simulink model "model"  (R2014a)
(part 1 of 4)
settings: Solver=VariableStepAuto  StartTime=0.0  StopTime=10.0  RelTol=1e-3
libraries: powerlib x952
settings Model: Creator=lej  LastModifiedBy=leimhofe
settings DataIOCC: SaveFormat=Dataset
settings OptimizationCC: SimCompilerOptimization=off
settings DebuggingCC: MergeDetectMultiDrivingBlocksExec=error  SolverPrmCheckMsg=none  FrameProcessingCompatibilityMsg=error  AllowSymbolicDim=off
settings HardwareCC: ProdBitPerPointer=64  ProdLargestAtomicFloat=Float  ProdIntDivRoundTo=Zero  ProdEndianess=LittleEndian  ProdWordSize=64  ProdHWDeviceType=Intel->x86-64 (Windows64)
settings RTWCC: RTWCompilerOptimization=off
settings GRTTargetCC: GeneratePreprocessorConditionals=Use local settings
settings ConfigComp: CovMetricSettings=dw  CovHtmlReporting=on  CovSaveCumulativeToWorkspaceVar=on  CovSaveSingleToWorkspaceVar=on  CovExternalEMLEnable=off

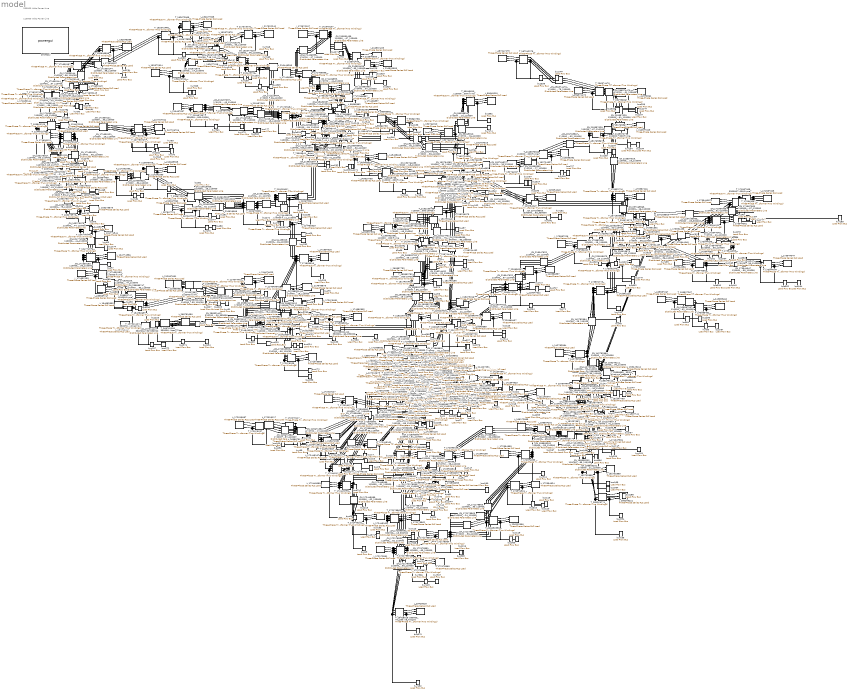
== system model ==
  note: 110000 Volts Power Line
  note: 330000 Volts Power Line
  G_166814917_Kauno_Algirdo_Brazausko_HE : powerlib/Electrical Sources/Three-Phase Source  Voltage=110000  PhaseAngle=0  Frequency=60  InternalConnection=Yg  SpecifyImpedance=on  Resistance=0.8929  Inductance=16.58e-3  ShortCircuitLevel=100e6  BaseVoltage=110000  XRratio=7  BusType=swing  Pref=0  Qref=0  Qmin=-inf  Qmax=inf
  G_172589995_ : powerlib/Electrical Sources/Three-Phase Source  Voltage=330000  PhaseAngle=0  Frequency=60  InternalConnection=Yg  SpecifyImpedance=on  Resistance=0.8929  Inductance=16.58e-3  ShortCircuitLevel=100e6  BaseVoltage=330000  XRratio=7  BusType=swing  Pref=0  Qref=0  Qmin=-inf  Qmax=inf
  L_{25698690,75909941,88726161,95066966,95066982,95866738,99049777,99049787,99049810,103275527,103275551,103275559,103275575,103554499,103560163,104774536,104774544,105587267,106172865,124462106,127212679,130577811..130577812,134987741,135644003,135895688,142782984,149408618,149815795,150992936,151097769,151237667,151783148,151783156,153249112,158244489,158505202,171229484,171406897,171406899,171630121,171630143..171630144,171630149,171630153,171630156..171630157,171809316,171868832,171987005,172018985,172019051,172019085,172019087,172019090,172019115,172019117,172019127,172178550..172178551,172178556,172178560,172178562..172178563,172394893,172394923..172394924,172394941,172407405,172445089,172445101..172445103,172445107,172590051,172590075..172590076,172590080..172590081,172590088,172590095..172590098,172590100..172590101,172590105,172590108,172590115..172590116,172978107,173582215..173582216,173582225..173582226,173591498,173591500,173591502,173593029,173612890,173765447,173944045,173944047,173944055..173944057,173944061,174045384,174586802,175315244,176323123,181769867,187242275,192646598,192672875,192672898,192672903,192672905,192672914,192677018,192702885,192764283,192764310,192764316,192764327,192764330..192764331,192764337,192764347,194082693,207755729..207755730,209204254,210449206,210457037,210457043,210550993,210551439,210555392,210557029,210609525,210612962,210619008,210619011,210995832,212007661,214227031,214455329,214649879,214649882,214674623,215632387,215671382,217323242,217391080,218047622,218214432,218216075,218223015..218223016,219077432,219084048,220065702,220915873,220986987,220989437,221105370,226292390,231990061,239589747,243085462,257169562..257169563,257507721,257684864..257684865,258321412,260552752,265807988,280078882,280269221,296374470} (182 alike) : powerlib/Elements/Three-Phase Series RLC Load  LConnTagsString=A|B|C  Configuration=Y (grounded)  NominalVoltage=110000  NominalFrequency=60  ActivePower=100000  InductivePower=100  CapacitivePower=100  Measurements=None  LoadType=constant Z
  L_{29428018,172590050,197911127,220065689,268781050} (5 alike) : powerlib/Elements/Three-Phase Series RLC Load  LConnTagsString=A|B|C  Configuration=Y (grounded)  NominalVoltage=330000  NominalFrequency=60  ActivePower=100000  InductivePower=100  CapacitivePower=100  Measurements=None  LoadType=constant Z
  T_103275527__ : powerlib/Elements/Three-Phase Transformer (Two Windings)  Winding1Connection=Yg  UNITS=pu  NominalPower=[ 250e6 , 60 ]  Winding1=[110000,0.002,0.08]  Winding2Connection=Yg  Winding2=[110000,0.002,0.08]  SetSaturation=off  Rm=500  Lm=500  Saturation=[ 0,0 ; 0.0024,1.2 ; 1.0,1.52 ]  Hysteresis=off  DataFile='hysteresis'  SetInitialFlux=off  InitialFluxes=[ 0.8 , -0.8 , 0.7 ]  Measurements=None  MoreParameters=off  BreakLoop=off  DataType=off  TransfoNumber=1
  T_103275551__ : powerlib/Elements/Three-Phase Transformer (Two Windings)  Winding1Connection=Yg  UNITS=pu  NominalPower=[ 250e6 , 60 ]  Winding1=[110000,0.002,0.08]  Winding2Connection=Yg  Winding2=[110000,0.002,0.08]  SetSaturation=off  Rm=500  Lm=500  Saturation=[ 0,0 ; 0.0024,1.2 ; 1.0,1.52 ]  Hysteresis=off  DataFile='hysteresis'  SetInitialFlux=off  InitialFluxes=[ 0.8 , -0.8 , 0.7 ]  Measurements=None  MoreParameters=off  BreakLoop=off  DataType=off  TransfoNumber=1
  T_103275559__ : powerlib/Elements/Three-Phase Transformer (Two Windings)  Winding1Connection=Yg  UNITS=pu  NominalPower=[ 250e6 , 60 ]  Winding1=[110000,0.002,0.08]  Winding2Connection=Yg  Winding2=[110000,0.002,0.08]  SetSaturation=off  Rm=500  Lm=500  Saturation=[ 0,0 ; 0.0024,1.2 ; 1.0,1.52 ]  Hysteresis=off  DataFile='hysteresis'  SetInitialFlux=off  InitialFluxes=[ 0.8 , -0.8 , 0.7 ]  Measurements=None  MoreParameters=off  BreakLoop=off  DataType=off  TransfoNumber=1
  T_103275575__ : powerlib/Elements/Three-Phase Transformer (Two Windings)  Winding1Connection=Yg  UNITS=pu  NominalPower=[ 250e6 , 60 ]  Winding1=[110000,0.002,0.08]  Winding2Connection=Yg  Winding2=[110000,0.002,0.08]  SetSaturation=off  Rm=500  Lm=500  Saturation=[ 0,0 ; 0.0024,1.2 ; 1.0,1.52 ]  Hysteresis=off  DataFile='hysteresis'  SetInitialFlux=off  InitialFluxes=[ 0.8 , -0.8 , 0.7 ]  Measurements=None  MoreParameters=off  BreakLoop=off  DataType=off  TransfoNumber=1
  T_103554499__ : powerlib/Elements/Three-Phase Transformer (Two Windings)  Winding1Connection=Yg  UNITS=pu  NominalPower=[ 250e6 , 60 ]  Winding1=[110000,0.002,0.08]  Winding2Connection=Yg  Winding2=[110000,0.002,0.08]  SetSaturation=off  Rm=500  Lm=500  Saturation=[ 0,0 ; 0.0024,1.2 ; 1.0,1.52 ]  Hysteresis=off  DataFile='hysteresis'  SetInitialFlux=off  InitialFluxes=[ 0.8 , -0.8 , 0.7 ]  Measurements=None  MoreParameters=off  BreakLoop=off  DataType=off  TransfoNumber=1
  T_103560163__ : powerlib/Elements/Three-Phase Transformer (Two Windings)  Winding1Connection=Yg  UNITS=pu  NominalPower=[ 250e6 , 60 ]  Winding1=[110000,0.002,0.08]  Winding2Connection=Yg  Winding2=[110000,0.002,0.08]  SetSaturation=off  Rm=500  Lm=500  Saturation=[ 0,0 ; 0.0024,1.2 ; 1.0,1.52 ]  Hysteresis=off  DataFile='hysteresis'  SetInitialFlux=off  InitialFluxes=[ 0.8 , -0.8 , 0.7 ]  Measurements=None  MoreParameters=off  BreakLoop=off  DataType=off  TransfoNumber=1
  T_104774536__ : powerlib/Elements/Three-Phase Transformer (Two Windings)  Winding1Connection=Yg  UNITS=pu  NominalPower=[ 250e6 , 60 ]  Winding1=[110000,0.002,0.08]  Winding2Connection=Yg  Winding2=[110000,0.002,0.08]  SetSaturation=off  Rm=500  Lm=500  Saturation=[ 0,0 ; 0.0024,1.2 ; 1.0,1.52 ]  Hysteresis=off  DataFile='hysteresis'  SetInitialFlux=off  InitialFluxes=[ 0.8 , -0.8 , 0.7 ]  Measurements=None  MoreParameters=off  BreakLoop=off  DataType=off  TransfoNumber=1
  T_104774544__ : powerlib/Elements/Three-Phase Transformer (Two Windings)  Winding1Connection=Yg  UNITS=pu  NominalPower=[ 250e6 , 60 ]  Winding1=[110000,0.002,0.08]  Winding2Connection=Yg  Winding2=[110000,0.002,0.08]  SetSaturation=off  Rm=500  Lm=500  Saturation=[ 0,0 ; 0.0024,1.2 ; 1.0,1.52 ]  Hysteresis=off  DataFile='hysteresis'  SetInitialFlux=off  InitialFluxes=[ 0.8 , -0.8 , 0.7 ]  Measurements=None  MoreParameters=off  BreakLoop=off  DataType=off  TransfoNumber=1
  T_105587267__ : powerlib/Elements/Three-Phase Transformer (Two Windings)  Winding1Connection=Yg  UNITS=pu  NominalPower=[ 250e6 , 60 ]  Winding1=[110000,0.002,0.08]  Winding2Connection=Yg  Winding2=[110000,0.002,0.08]  SetSaturation=off  Rm=500  Lm=500  Saturation=[ 0,0 ; 0.0024,1.2 ; 1.0,1.52 ]  Hysteresis=off  DataFile='hysteresis'  SetInitialFlux=off  InitialFluxes=[ 0.8 , -0.8 , 0.7 ]  Measurements=None  MoreParameters=off  BreakLoop=off  DataType=off  TransfoNumber=1
  T_106172865__ : powerlib/Elements/Three-Phase Transformer (Two Windings)  Winding1Connection=Yg  UNITS=pu  NominalPower=[ 250e6 , 60 ]  Winding1=[110000,0.002,0.08]  Winding2Connection=Yg  Winding2=[110000,0.002,0.08]  SetSaturation=off  Rm=500  Lm=500  Saturation=[ 0,0 ; 0.0024,1.2 ; 1.0,1.52 ]  Hysteresis=off  DataFile='hysteresis'  SetInitialFlux=off  InitialFluxes=[ 0.8 , -0.8 , 0.7 ]  Measurements=None  MoreParameters=off  BreakLoop=off  DataType=off  TransfoNumber=1
  T_124462106__ : powerlib/Elements/Three-Phase Transformer (Two Windings)  Winding1Connection=Yg  UNITS=pu  NominalPower=[ 250e6 , 60 ]  Winding1=[110000,0.002,0.08]  Winding2Connection=Yg  Winding2=[110000,0.002,0.08]  SetSaturation=off  Rm=500  Lm=500  Saturation=[ 0,0 ; 0.0024,1.2 ; 1.0,1.52 ]  Hysteresis=off  DataFile='hysteresis'  SetInitialFlux=off  InitialFluxes=[ 0.8 , -0.8 , 0.7 ]  Measurements=None  MoreParameters=off  BreakLoop=off  DataType=off  TransfoNumber=1
  T_127212679__Noreikiškių_TP : powerlib/Elements/Three-Phase Transformer (Two Windings)  Winding1Connection=Yg  UNITS=pu  NominalPower=[ 250e6 , 60 ]  Winding1=[110000,0.002,0.08]  Winding2Connection=Yg  Winding2=[110000,0.002,0.08]  SetSaturation=off  Rm=500  Lm=500  Saturation=[ 0,0 ; 0.0024,1.2 ; 1.0,1.52 ]  Hysteresis=off  DataFile='hysteresis'  SetInitialFlux=off  InitialFluxes=[ 0.8 , -0.8 , 0.7 ]  Measurements=None  MoreParameters=off  BreakLoop=off  DataType=off  TransfoNumber=1
  T_130577811__Vilijampolės_TP : powerlib/Elements/Three-Phase Transformer (Two Windings)  Winding1Connection=Yg  UNITS=pu  NominalPower=[ 250e6 , 60 ]  Winding1=[110000,0.002,0.08]  Winding2Connection=Yg  Winding2=[110000,0.002,0.08]  SetSaturation=off  Rm=500  Lm=500  Saturation=[ 0,0 ; 0.0024,1.2 ; 1.0,1.52 ]  Hysteresis=off  DataFile='hysteresis'  SetInitialFlux=off  InitialFluxes=[ 0.8 , -0.8 , 0.7 ]  Measurements=None  MoreParameters=off  BreakLoop=off  DataType=off  TransfoNumber=1
  T_130577812__Šilainių_TP : powerlib/Elements/Three-Phase Transformer (Two Windings)  Winding1Connection=Yg  UNITS=pu  NominalPower=[ 250e6 , 60 ]  Winding1=[110000,0.002,0.08]  Winding2Connection=Yg  Winding2=[110000,0.002,0.08]  SetSaturation=off  Rm=500  Lm=500  Saturation=[ 0,0 ; 0.0024,1.2 ; 1.0,1.52 ]  Hysteresis=off  DataFile='hysteresis'  SetInitialFlux=off  InitialFluxes=[ 0.8 , -0.8 , 0.7 ]  Measurements=None  MoreParameters=off  BreakLoop=off  DataType=off  TransfoNumber=1
  T_134987741__ : powerlib/Elements/Three-Phase Transformer (Two Windings)  Winding1Connection=Yg  UNITS=pu  NominalPower=[ 250e6 , 60 ]  Winding1=[110000,0.002,0.08]  Winding2Connection=Yg  Winding2=[110000,0.002,0.08]  SetSaturation=off  Rm=500  Lm=500  Saturation=[ 0,0 ; 0.0024,1.2 ; 1.0,1.52 ]  Hysteresis=off  DataFile='hysteresis'  SetInitialFlux=off  InitialFluxes=[ 0.8 , -0.8 , 0.7 ]  Measurements=None  MoreParameters=off  BreakLoop=off  DataType=off  TransfoNumber=1
  T_135644003__ : powerlib/Elements/Three-Phase Transformer (Two Windings)  Winding1Connection=Yg  UNITS=pu  NominalPower=[ 250e6 , 60 ]  Winding1=[110000,0.002,0.08]  Winding2Connection=Yg  Winding2=[110000,0.002,0.08]  SetSaturation=off  Rm=500  Lm=500  Saturation=[ 0,0 ; 0.0024,1.2 ; 1.0,1.52 ]  Hysteresis=off  DataFile='hysteresis'  SetInitialFlux=off  InitialFluxes=[ 0.8 , -0.8 , 0.7 ]  Measurements=None  MoreParameters=off  BreakLoop=off  DataType=off  TransfoNumber=1
  T_135895688__Palemono_Traukos_TP : powerlib/Elements/Three-Phase Transformer (Two Windings)  Winding1Connection=Yg  UNITS=pu  NominalPower=[ 250e6 , 60 ]  Winding1=[110000,0.002,0.08]  Winding2Connection=Yg  Winding2=[110000,0.002,0.08]  SetSaturation=off  Rm=500  Lm=500  Saturation=[ 0,0 ; 0.0024,1.2 ; 1.0,1.52 ]  Hysteresis=off  DataFile='hysteresis'  SetInitialFlux=off  InitialFluxes=[ 0.8 , -0.8 , 0.7 ]  Measurements=None  MoreParameters=off  BreakLoop=off  DataType=off  TransfoNumber=1
  T_142782984__ : powerlib/Elements/Three-Phase Transformer (Two Windings)  Winding1Connection=Yg  UNITS=pu  NominalPower=[ 250e6 , 60 ]  Winding1=[110000,0.002,0.08]  Winding2Connection=Yg  Winding2=[110000,0.002,0.08]  SetSaturation=off  Rm=500  Lm=500  Saturation=[ 0,0 ; 0.0024,1.2 ; 1.0,1.52 ]  Hysteresis=off  DataFile='hysteresis'  SetInitialFlux=off  InitialFluxes=[ 0.8 , -0.8 , 0.7 ]  Measurements=None  MoreParameters=off  BreakLoop=off  DataType=off  TransfoNumber=1
  T_149408618__ : powerlib/Elements/Three-Phase Transformer (Two Windings)  Winding1Connection=Yg  UNITS=pu  NominalPower=[ 250e6 , 60 ]  Winding1=[110000,0.002,0.08]  Winding2Connection=Yg  Winding2=[110000,0.002,0.08]  SetSaturation=off  Rm=500  Lm=500  Saturation=[ 0,0 ; 0.0024,1.2 ; 1.0,1.52 ]  Hysteresis=off  DataFile='hysteresis'  SetInitialFlux=off  InitialFluxes=[ 0.8 , -0.8 , 0.7 ]  Measurements=None  MoreParameters=off  BreakLoop=off  DataType=off  TransfoNumber=1
  T_149815795_110000;35000;fixme_ : powerlib/Elements/Three-Phase Transformer (Two Windings)  Winding1Connection=Yg  UNITS=pu  NominalPower=[ 250e6 , 60 ]  Winding1=[110000,0.002,0.08]  Winding2Connection=Yg  Winding2=[110000,0.002,0.08]  SetSaturation=off  Rm=500  Lm=500  Saturation=[ 0,0 ; 0.0024,1.2 ; 1.0,1.52 ]  Hysteresis=off  DataFile='hysteresis'  SetInitialFlux=off  InitialFluxes=[ 0.8 , -0.8 , 0.7 ]  Measurements=None  MoreParameters=off  BreakLoop=off  DataType=off  TransfoNumber=1
  T_150992936_110000;35000;fixme_ : powerlib/Elements/Three-Phase Transformer (Two Windings)  Winding1Connection=Yg  UNITS=pu  NominalPower=[ 250e6 , 60 ]  Winding1=[110000,0.002,0.08]  Winding2Connection=Yg  Winding2=[110000,0.002,0.08]  SetSaturation=off  Rm=500  Lm=500  Saturation=[ 0,0 ; 0.0024,1.2 ; 1.0,1.52 ]  Hysteresis=off  DataFile='hysteresis'  SetInitialFlux=off  InitialFluxes=[ 0.8 , -0.8 , 0.7 ]  Measurements=None  MoreParameters=off  BreakLoop=off  DataType=off  TransfoNumber=1
  T_151097769__ : powerlib/Elements/Three-Phase Transformer (Two Windings)  Winding1Connection=Yg  UNITS=pu  NominalPower=[ 250e6 , 60 ]  Winding1=[110000,0.002,0.08]  Winding2Connection=Yg  Winding2=[110000,0.002,0.08]  SetSaturation=off  Rm=500  Lm=500  Saturation=[ 0,0 ; 0.0024,1.2 ; 1.0,1.52 ]  Hysteresis=off  DataFile='hysteresis'  SetInitialFlux=off  InitialFluxes=[ 0.8 , -0.8 , 0.7 ]  Measurements=None  MoreParameters=off  BreakLoop=off  DataType=off  TransfoNumber=1
  T_151237667__ : powerlib/Elements/Three-Phase Transformer (Two Windings)  Winding1Connection=Yg  UNITS=pu  NominalPower=[ 250e6 , 60 ]  Winding1=[110000,0.002,0.08]  Winding2Connection=Yg  Winding2=[110000,0.002,0.08]  SetSaturation=off  Rm=500  Lm=500  Saturation=[ 0,0 ; 0.0024,1.2 ; 1.0,1.52 ]  Hysteresis=off  DataFile='hysteresis'  SetInitialFlux=off  InitialFluxes=[ 0.8 , -0.8 , 0.7 ]  Measurements=None  MoreParameters=off  BreakLoop=off  DataType=off  TransfoNumber=1
  T_151783148_110000;fixme_ : powerlib/Elements/Three-Phase Transformer (Two Windings)  Winding1Connection=Yg  UNITS=pu  NominalPower=[ 250e6 , 60 ]  Winding1=[110000,0.002,0.08]  Winding2Connection=Yg  Winding2=[110000,0.002,0.08]  SetSaturation=off  Rm=500  Lm=500  Saturation=[ 0,0 ; 0.0024,1.2 ; 1.0,1.52 ]  Hysteresis=off  DataFile='hysteresis'  SetInitialFlux=off  InitialFluxes=[ 0.8 , -0.8 , 0.7 ]  Measurements=None  MoreParameters=off  BreakLoop=off  DataType=off  TransfoNumber=1
  T_151783156__ : powerlib/Elements/Three-Phase Transformer (Two Windings)  Winding1Connection=Yg  UNITS=pu  NominalPower=[ 250e6 , 60 ]  Winding1=[110000,0.002,0.08]  Winding2Connection=Yg  Winding2=[110000,0.002,0.08]  SetSaturation=off  Rm=500  Lm=500  Saturation=[ 0,0 ; 0.0024,1.2 ; 1.0,1.52 ]  Hysteresis=off  DataFile='hysteresis'  SetInitialFlux=off  InitialFluxes=[ 0.8 , -0.8 , 0.7 ]  Measurements=None  MoreParameters=off  BreakLoop=off  DataType=off  TransfoNumber=1
  T_153249112__ : powerlib/Elements/Three-Phase Transformer (Two Windings)  Winding1Connection=Yg  UNITS=pu  NominalPower=[ 250e6 , 60 ]  Winding1=[110000,0.002,0.08]  Winding2Connection=Yg  Winding2=[110000,0.002,0.08]  SetSaturation=off  Rm=500  Lm=500  Saturation=[ 0,0 ; 0.0024,1.2 ; 1.0,1.52 ]  Hysteresis=off  DataFile='hysteresis'  SetInitialFlux=off  InitialFluxes=[ 0.8 , -0.8 , 0.7 ]  Measurements=None  MoreParameters=off  BreakLoop=off  DataType=off  TransfoNumber=1
  T_158244489__Palemono_TP : powerlib/Elements/Three-Phase Transformer (Two Windings)  Winding1Connection=Yg  UNITS=pu  NominalPower=[ 250e6 , 60 ]  Winding1=[110000,0.002,0.08]  Winding2Connection=Yg  Winding2=[110000,0.002,0.08]  SetSaturation=off  Rm=500  Lm=500  Saturation=[ 0,0 ; 0.0024,1.2 ; 1.0,1.52 ]  Hysteresis=off  DataFile='hysteresis'  SetInitialFlux=off  InitialFluxes=[ 0.8 , -0.8 , 0.7 ]  Measurements=None  MoreParameters=off  BreakLoop=off  DataType=off  TransfoNumber=1
  T_158505202__ : powerlib/Elements/Three-Phase Transformer (Two Windings)  Winding1Connection=Yg  UNITS=pu  NominalPower=[ 250e6 , 60 ]  Winding1=[330000,0.002,0.08]  Winding2Connection=Yg  Winding2=[110000,0.002,0.08]  SetSaturation=off  Rm=500  Lm=500  Saturation=[ 0,0 ; 0.0024,1.2 ; 1.0,1.52 ]  Hysteresis=off  DataFile='hysteresis'  SetInitialFlux=off  InitialFluxes=[ 0.8 , -0.8 , 0.7 ]  Measurements=None  MoreParameters=off  BreakLoop=off  DataType=off  TransfoNumber=1
  T_171229484__ : powerlib/Elements/Three-Phase Transformer (Two Windings)  Winding1Connection=Yg  UNITS=pu  NominalPower=[ 250e6 , 60 ]  Winding1=[110000,0.002,0.08]  Winding2Connection=Yg  Winding2=[110000,0.002,0.08]  SetSaturation=off  Rm=500  Lm=500  Saturation=[ 0,0 ; 0.0024,1.2 ; 1.0,1.52 ]  Hysteresis=off  DataFile='hysteresis'  SetInitialFlux=off  InitialFluxes=[ 0.8 , -0.8 , 0.7 ]  Measurements=None  MoreParameters=off  BreakLoop=off  DataType=off  TransfoNumber=1
  T_171406897__ : powerlib/Elements/Three-Phase Transformer (Two Windings)  Winding1Connection=Yg  UNITS=pu  NominalPower=[ 250e6 , 60 ]  Winding1=[110000,0.002,0.08]  Winding2Connection=Yg  Winding2=[110000,0.002,0.08]  SetSaturation=off  Rm=500  Lm=500  Saturation=[ 0,0 ; 0.0024,1.2 ; 1.0,1.52 ]  Hysteresis=off  DataFile='hysteresis'  SetInitialFlux=off  InitialFluxes=[ 0.8 , -0.8 , 0.7 ]  Measurements=None  MoreParameters=off  BreakLoop=off  DataType=off  TransfoNumber=1
  T_171406899__ : powerlib/Elements/Three-Phase Transformer (Two Windings)  Winding1Connection=Yg  UNITS=pu  NominalPower=[ 250e6 , 60 ]  Winding1=[110000,0.002,0.08]  Winding2Connection=Yg  Winding2=[110000,0.002,0.08]  SetSaturation=off  Rm=500  Lm=500  Saturation=[ 0,0 ; 0.0024,1.2 ; 1.0,1.52 ]  Hysteresis=off  DataFile='hysteresis'  SetInitialFlux=off  InitialFluxes=[ 0.8 , -0.8 , 0.7 ]  Measurements=None  MoreParameters=off  BreakLoop=off  DataType=off  TransfoNumber=1
  T_171630121__ : powerlib/Elements/Three-Phase Transformer (Two Windings)  Winding1Connection=Yg  UNITS=pu  NominalPower=[ 250e6 , 60 ]  Winding1=[110000,0.002,0.08]  Winding2Connection=Yg  Winding2=[110000,0.002,0.08]  SetSaturation=off  Rm=500  Lm=500  Saturation=[ 0,0 ; 0.0024,1.2 ; 1.0,1.52 ]  Hysteresis=off  DataFile='hysteresis'  SetInitialFlux=off  InitialFluxes=[ 0.8 , -0.8 , 0.7 ]  Measurements=None  MoreParameters=off  BreakLoop=off  DataType=off  TransfoNumber=1
  T_171630143__ : powerlib/Elements/Three-Phase Transformer (Two Windings)  Winding1Connection=Yg  UNITS=pu  NominalPower=[ 250e6 , 60 ]  Winding1=[110000,0.002,0.08]  Winding2Connection=Yg  Winding2=[110000,0.002,0.08]  SetSaturation=off  Rm=500  Lm=500  Saturation=[ 0,0 ; 0.0024,1.2 ; 1.0,1.52 ]  Hysteresis=off  DataFile='hysteresis'  SetInitialFlux=off  InitialFluxes=[ 0.8 , -0.8 , 0.7 ]  Measurements=None  MoreParameters=off  BreakLoop=off  DataType=off  TransfoNumber=1
  T_171630144__ : powerlib/Elements/Three-Phase Transformer (Two Windings)  Winding1Connection=Yg  UNITS=pu  NominalPower=[ 250e6 , 60 ]  Winding1=[110000,0.002,0.08]  Winding2Connection=Yg  Winding2=[110000,0.002,0.08]  SetSaturation=off  Rm=500  Lm=500  Saturation=[ 0,0 ; 0.0024,1.2 ; 1.0,1.52 ]  Hysteresis=off  DataFile='hysteresis'  SetInitialFlux=off  InitialFluxes=[ 0.8 , -0.8 , 0.7 ]  Measurements=None  MoreParameters=off  BreakLoop=off  DataType=off  TransfoNumber=1
  T_171630149__ : powerlib/Elements/Three-Phase Transformer (Two Windings)  Winding1Connection=Yg  UNITS=pu  NominalPower=[ 250e6 , 60 ]  Winding1=[110000,0.002,0.08]  Winding2Connection=Yg  Winding2=[110000,0.002,0.08]  SetSaturation=off  Rm=500  Lm=500  Saturation=[ 0,0 ; 0.0024,1.2 ; 1.0,1.52 ]  Hysteresis=off  DataFile='hysteresis'  SetInitialFlux=off  InitialFluxes=[ 0.8 , -0.8 , 0.7 ]  Measurements=None  MoreParameters=off  BreakLoop=off  DataType=off  TransfoNumber=1
  T_171630153_110000;fixme_ : powerlib/Elements/Three-Phase Transformer (Two Windings)  Winding1Connection=Yg  UNITS=pu  NominalPower=[ 250e6 , 60 ]  Winding1=[110000,0.002,0.08]  Winding2Connection=Yg  Winding2=[110000,0.002,0.08]  SetSaturation=off  Rm=500  Lm=500  Saturation=[ 0,0 ; 0.0024,1.2 ; 1.0,1.52 ]  Hysteresis=off  DataFile='hysteresis'  SetInitialFlux=off  InitialFluxes=[ 0.8 , -0.8 , 0.7 ]  Measurements=None  MoreParameters=off  BreakLoop=off  DataType=off  TransfoNumber=1
  T_171630156__ : powerlib/Elements/Three-Phase Transformer (Two Windings)  Winding1Connection=Yg  UNITS=pu  NominalPower=[ 250e6 , 60 ]  Winding1=[110000,0.002,0.08]  Winding2Connection=Yg  Winding2=[110000,0.002,0.08]  SetSaturation=off  Rm=500  Lm=500  Saturation=[ 0,0 ; 0.0024,1.2 ; 1.0,1.52 ]  Hysteresis=off  DataFile='hysteresis'  SetInitialFlux=off  InitialFluxes=[ 0.8 , -0.8 , 0.7 ]  Measurements=None  MoreParameters=off  BreakLoop=off  DataType=off  TransfoNumber=1
  T_171630157__ : powerlib/Elements/Three-Phase Transformer (Two Windings)  Winding1Connection=Yg  UNITS=pu  NominalPower=[ 250e6 , 60 ]  Winding1=[110000,0.002,0.08]  Winding2Connection=Yg  Winding2=[110000,0.002,0.08]  SetSaturation=off  Rm=500  Lm=500  Saturation=[ 0,0 ; 0.0024,1.2 ; 1.0,1.52 ]  Hysteresis=off  DataFile='hysteresis'  SetInitialFlux=off  InitialFluxes=[ 0.8 , -0.8 , 0.7 ]  Measurements=None  MoreParameters=off  BreakLoop=off  DataType=off  TransfoNumber=1
  T_171809316__ : powerlib/Elements/Three-Phase Transformer (Two Windings)  Winding1Connection=Yg  UNITS=pu  NominalPower=[ 250e6 , 60 ]  Winding1=[110000,0.002,0.08]  Winding2Connection=Yg  Winding2=[110000,0.002,0.08]  SetSaturation=off  Rm=500  Lm=500  Saturation=[ 0,0 ; 0.0024,1.2 ; 1.0,1.52 ]  Hysteresis=off  DataFile='hysteresis'  SetInitialFlux=off  InitialFluxes=[ 0.8 , -0.8 , 0.7 ]  Measurements=None  MoreParameters=off  BreakLoop=off  DataType=off  TransfoNumber=1
  T_171868832__ : powerlib/Elements/Three-Phase Transformer (Two Windings)  Winding1Connection=Yg  UNITS=pu  NominalPower=[ 250e6 , 60 ]  Winding1=[110000,0.002,0.08]  Winding2Connection=Yg  Winding2=[110000,0.002,0.08]  SetSaturation=off  Rm=500  Lm=500  Saturation=[ 0,0 ; 0.0024,1.2 ; 1.0,1.52 ]  Hysteresis=off  DataFile='hysteresis'  SetInitialFlux=off  InitialFluxes=[ 0.8 , -0.8 , 0.7 ]  Measurements=None  MoreParameters=off  BreakLoop=off  DataType=off  TransfoNumber=1
  T_171987005_330000;110000;fixme_ : powerlib/Elements/Three-Phase Transformer (Two Windings)  Winding1Connection=Yg  UNITS=pu  NominalPower=[ 250e6 , 60 ]  Winding1=[330000,0.002,0.08]  Winding2Connection=Yg  Winding2=[110000,0.002,0.08]  SetSaturation=off  Rm=500  Lm=500  Saturation=[ 0,0 ; 0.0024,1.2 ; 1.0,1.52 ]  Hysteresis=off  DataFile='hysteresis'  SetInitialFlux=off  InitialFluxes=[ 0.8 , -0.8 , 0.7 ]  Measurements=None  MoreParameters=off  BreakLoop=off  DataType=off  TransfoNumber=1
  T_172018985__ : powerlib/Elements/Three-Phase Transformer (Two Windings)  Winding1Connection=Yg  UNITS=pu  NominalPower=[ 250e6 , 60 ]  Winding1=[110000,0.002,0.08]  Winding2Connection=Yg  Winding2=[110000,0.002,0.08]  SetSaturation=off  Rm=500  Lm=500  Saturation=[ 0,0 ; 0.0024,1.2 ; 1.0,1.52 ]  Hysteresis=off  DataFile='hysteresis'  SetInitialFlux=off  InitialFluxes=[ 0.8 , -0.8 , 0.7 ]  Measurements=None  MoreParameters=off  BreakLoop=off  DataType=off  TransfoNumber=1
  T_172019051__ : powerlib/Elements/Three-Phase Transformer (Two Windings)  Winding1Connection=Yg  UNITS=pu  NominalPower=[ 250e6 , 60 ]  Winding1=[110000,0.002,0.08]  Winding2Connection=Yg  Winding2=[110000,0.002,0.08]  SetSaturation=off  Rm=500  Lm=500  Saturation=[ 0,0 ; 0.0024,1.2 ; 1.0,1.52 ]  Hysteresis=off  DataFile='hysteresis'  SetInitialFlux=off  InitialFluxes=[ 0.8 , -0.8 , 0.7 ]  Measurements=None  MoreParameters=off  BreakLoop=off  DataType=off  TransfoNumber=1
  T_172019085__ : powerlib/Elements/Three-Phase Transformer (Two Windings)  Winding1Connection=Yg  UNITS=pu  NominalPower=[ 250e6 , 60 ]  Winding1=[110000,0.002,0.08]  Winding2Connection=Yg  Winding2=[110000,0.002,0.08]  SetSaturation=off  Rm=500  Lm=500  Saturation=[ 0,0 ; 0.0024,1.2 ; 1.0,1.52 ]  Hysteresis=off  DataFile='hysteresis'  SetInitialFlux=off  InitialFluxes=[ 0.8 , -0.8 , 0.7 ]  Measurements=None  MoreParameters=off  BreakLoop=off  DataType=off  TransfoNumber=1
  T_172019087__ : powerlib/Elements/Three-Phase Transformer (Two Windings)  Winding1Connection=Yg  UNITS=pu  NominalPower=[ 250e6 , 60 ]  Winding1=[110000,0.002,0.08]  Winding2Connection=Yg  Winding2=[110000,0.002,0.08]  SetSaturation=off  Rm=500  Lm=500  Saturation=[ 0,0 ; 0.0024,1.2 ; 1.0,1.52 ]  Hysteresis=off  DataFile='hysteresis'  SetInitialFlux=off  InitialFluxes=[ 0.8 , -0.8 , 0.7 ]  Measurements=None  MoreParameters=off  BreakLoop=off  DataType=off  TransfoNumber=1
  T_172019090__ : powerlib/Elements/Three-Phase Transformer (Two Windings)  Winding1Connection=Yg  UNITS=pu  NominalPower=[ 250e6 , 60 ]  Winding1=[110000,0.002,0.08]  Winding2Connection=Yg  Winding2=[110000,0.002,0.08]  SetSaturation=off  Rm=500  Lm=500  Saturation=[ 0,0 ; 0.0024,1.2 ; 1.0,1.52 ]  Hysteresis=off  DataFile='hysteresis'  SetInitialFlux=off  InitialFluxes=[ 0.8 , -0.8 , 0.7 ]  Measurements=None  MoreParameters=off  BreakLoop=off  DataType=off  TransfoNumber=1
  T_172019115__Aleksoto_TP : powerlib/Elements/Three-Phase Transformer (Two Windings)  Winding1Connection=Yg  UNITS=pu  NominalPower=[ 250e6 , 60 ]  Winding1=[110000,0.002,0.08]  Winding2Connection=Yg  Winding2=[110000,0.002,0.08]  SetSaturation=off  Rm=500  Lm=500  Saturation=[ 0,0 ; 0.0024,1.2 ; 1.0,1.52 ]  Hysteresis=off  DataFile='hysteresis'  SetInitialFlux=off  InitialFluxes=[ 0.8 , -0.8 , 0.7 ]  Measurements=None  MoreParameters=off  BreakLoop=off  DataType=off  TransfoNumber=1
  T_172019117__ : powerlib/Elements/Three-Phase Transformer (Two Windings)  Winding1Connection=Yg  UNITS=pu  NominalPower=[ 250e6 , 60 ]  Winding1=[110000,0.002,0.08]  Winding2Connection=Yg  Winding2=[110000,0.002,0.08]  SetSaturation=off  Rm=500  Lm=500  Saturation=[ 0,0 ; 0.0024,1.2 ; 1.0,1.52 ]  Hysteresis=off  DataFile='hysteresis'  SetInitialFlux=off  InitialFluxes=[ 0.8 , -0.8 , 0.7 ]  Measurements=None  MoreParameters=off  BreakLoop=off  DataType=off  TransfoNumber=1
  T_172019127__ : powerlib/Elements/Three-Phase Transformer (Two Windings)  Winding1Connection=Yg  UNITS=pu  NominalPower=[ 250e6 , 60 ]  Winding1=[110000,0.002,0.08]  Winding2Connection=Yg  Winding2=[110000,0.002,0.08]  SetSaturation=off  Rm=500  Lm=500  Saturation=[ 0,0 ; 0.0024,1.2 ; 1.0,1.52 ]  Hysteresis=off  DataFile='hysteresis'  SetInitialFlux=off  InitialFluxes=[ 0.8 , -0.8 , 0.7 ]  Measurements=None  MoreParameters=off  BreakLoop=off  DataType=off  TransfoNumber=1
  T_172178550__ : powerlib/Elements/Three-Phase Transformer (Two Windings)  Winding1Connection=Yg  UNITS=pu  NominalPower=[ 250e6 , 60 ]  Winding1=[110000,0.002,0.08]  Winding2Connection=Yg  Winding2=[110000,0.002,0.08]  SetSaturation=off  Rm=500  Lm=500  Saturation=[ 0,0 ; 0.0024,1.2 ; 1.0,1.52 ]  Hysteresis=off  DataFile='hysteresis'  SetInitialFlux=off  InitialFluxes=[ 0.8 , -0.8 , 0.7 ]  Measurements=None  MoreParameters=off  BreakLoop=off  DataType=off  TransfoNumber=1
  T_172178551__ : powerlib/Elements/Three-Phase Transformer (Two Windings)  Winding1Connection=Yg  UNITS=pu  NominalPower=[ 250e6 , 60 ]  Winding1=[110000,0.002,0.08]  Winding2Connection=Yg  Winding2=[110000,0.002,0.08]  SetSaturation=off  Rm=500  Lm=500  Saturation=[ 0,0 ; 0.0024,1.2 ; 1.0,1.52 ]  Hysteresis=off  DataFile='hysteresis'  SetInitialFlux=off  InitialFluxes=[ 0.8 , -0.8 , 0.7 ]  Measurements=None  MoreParameters=off  BreakLoop=off  DataType=off  TransfoNumber=1
  T_172178556__ : powerlib/Elements/Three-Phase Transformer (Two Windings)  Winding1Connection=Yg  UNITS=pu  NominalPower=[ 250e6 , 60 ]  Winding1=[110000,0.002,0.08]  Winding2Connection=Yg  Winding2=[110000,0.002,0.08]  SetSaturation=off  Rm=500  Lm=500  Saturation=[ 0,0 ; 0.0024,1.2 ; 1.0,1.52 ]  Hysteresis=off  DataFile='hysteresis'  SetInitialFlux=off  InitialFluxes=[ 0.8 , -0.8 , 0.7 ]  Measurements=None  MoreParameters=off  BreakLoop=off  DataType=off  TransfoNumber=1
  T_172178560__ : powerlib/Elements/Three-Phase Transformer (Two Windings)  Winding1Connection=Yg  UNITS=pu  NominalPower=[ 250e6 , 60 ]  Winding1=[110000,0.002,0.08]  Winding2Connection=Yg  Winding2=[110000,0.002,0.08]  SetSaturation=off  Rm=500  Lm=500  Saturation=[ 0,0 ; 0.0024,1.2 ; 1.0,1.52 ]  Hysteresis=off  DataFile='hysteresis'  SetInitialFlux=off  InitialFluxes=[ 0.8 , -0.8 , 0.7 ]  Measurements=None  MoreParameters=off  BreakLoop=off  DataType=off  TransfoNumber=1
  T_172178562__ : powerlib/Elements/Three-Phase Transformer (Two Windings)  Winding1Connection=Yg  UNITS=pu  NominalPower=[ 250e6 , 60 ]  Winding1=[110000,0.002,0.08]  Winding2Connection=Yg  Winding2=[110000,0.002,0.08]  SetSaturation=off  Rm=500  Lm=500  Saturation=[ 0,0 ; 0.0024,1.2 ; 1.0,1.52 ]  Hysteresis=off  DataFile='hysteresis'  SetInitialFlux=off  InitialFluxes=[ 0.8 , -0.8 , 0.7 ]  Measurements=None  MoreParameters=off  BreakLoop=off  DataType=off  TransfoNumber=1
  T_172178563__ : powerlib/Elements/Three-Phase Transformer (Two Windings)  Winding1Connection=Yg  UNITS=pu  NominalPower=[ 250e6 , 60 ]  Winding1=[110000,0.002,0.08]  Winding2Connection=Yg  Winding2=[110000,0.002,0.08]  SetSaturation=off  Rm=500  Lm=500  Saturation=[ 0,0 ; 0.0024,1.2 ; 1.0,1.52 ]  Hysteresis=off  DataFile='hysteresis'  SetInitialFlux=off  InitialFluxes=[ 0.8 , -0.8 , 0.7 ]  Measurements=None  MoreParameters=off  BreakLoop=off  DataType=off  TransfoNumber=1
  T_172394893__ : powerlib/Elements/Three-Phase Transformer (Two Windings)  Winding1Connection=Yg  UNITS=pu  NominalPower=[ 250e6 , 60 ]  Winding1=[110000,0.002,0.08]  Winding2Connection=Yg  Winding2=[110000,0.002,0.08]  SetSaturation=off  Rm=500  Lm=500  Saturation=[ 0,0 ; 0.0024,1.2 ; 1.0,1.52 ]  Hysteresis=off  DataFile='hysteresis'  SetInitialFlux=off  InitialFluxes=[ 0.8 , -0.8 , 0.7 ]  Measurements=None  MoreParameters=off  BreakLoop=off  DataType=off  TransfoNumber=1
  T_172394923__ : powerlib/Elements/Three-Phase Transformer (Two Windings)  Winding1Connection=Yg  UNITS=pu  NominalPower=[ 250e6 , 60 ]  Winding1=[110000,0.002,0.08]  Winding2Connection=Yg  Winding2=[110000,0.002,0.08]  SetSaturation=off  Rm=500  Lm=500  Saturation=[ 0,0 ; 0.0024,1.2 ; 1.0,1.52 ]  Hysteresis=off  DataFile='hysteresis'  SetInitialFlux=off  InitialFluxes=[ 0.8 , -0.8 , 0.7 ]  Measurements=None  MoreParameters=off  BreakLoop=off  DataType=off  TransfoNumber=1
  T_172394924__ : powerlib/Elements/Three-Phase Transformer (Two Windings)  Winding1Connection=Yg  UNITS=pu  NominalPower=[ 250e6 , 60 ]  Winding1=[110000,0.002,0.08]  Winding2Connection=Yg  Winding2=[110000,0.002,0.08]  SetSaturation=off  Rm=500  Lm=500  Saturation=[ 0,0 ; 0.0024,1.2 ; 1.0,1.52 ]  Hysteresis=off  DataFile='hysteresis'  SetInitialFlux=off  InitialFluxes=[ 0.8 , -0.8 , 0.7 ]  Measurements=None  MoreParameters=off  BreakLoop=off  DataType=off  TransfoNumber=1
  T_172394941__ : powerlib/Elements/Three-Phase Transformer (Two Windings)  Winding1Connection=Yg  UNITS=pu  NominalPower=[ 250e6 , 60 ]  Winding1=[110000,0.002,0.08]  Winding2Connection=Yg  Winding2=[110000,0.002,0.08]  SetSaturation=off  Rm=500  Lm=500  Saturation=[ 0,0 ; 0.0024,1.2 ; 1.0,1.52 ]  Hysteresis=off  DataFile='hysteresis'  SetInitialFlux=off  InitialFluxes=[ 0.8 , -0.8 , 0.7 ]  Measurements=None  MoreParameters=off  BreakLoop=off  DataType=off  TransfoNumber=1
  T_172407405__ : powerlib/Elements/Three-Phase Transformer (Two Windings)  Winding1Connection=Yg  UNITS=pu  NominalPower=[ 250e6 , 60 ]  Winding1=[110000,0.002,0.08]  Winding2Connection=Yg  Winding2=[110000,0.002,0.08]  SetSaturation=off  Rm=500  Lm=500  Saturation=[ 0,0 ; 0.0024,1.2 ; 1.0,1.52 ]  Hysteresis=off  DataFile='hysteresis'  SetInitialFlux=off  InitialFluxes=[ 0.8 , -0.8 , 0.7 ]  Measurements=None  MoreParameters=off  BreakLoop=off  DataType=off  TransfoNumber=1
  T_172445089__ : powerlib/Elements/Three-Phase Transformer (Two Windings)  Winding1Connection=Yg  UNITS=pu  NominalPower=[ 250e6 , 60 ]  Winding1=[110000,0.002,0.08]  Winding2Connection=Yg  Winding2=[110000,0.002,0.08]  SetSaturation=off  Rm=500  Lm=500  Saturation=[ 0,0 ; 0.0024,1.2 ; 1.0,1.52 ]  Hysteresis=off  DataFile='hysteresis'  SetInitialFlux=off  InitialFluxes=[ 0.8 , -0.8 , 0.7 ]  Measurements=None  MoreParameters=off  BreakLoop=off  DataType=off  TransfoNumber=1
  T_172445101__ : powerlib/Elements/Three-Phase Transformer (Two Windings)  Winding1Connection=Yg  UNITS=pu  NominalPower=[ 250e6 , 60 ]  Winding1=[110000,0.002,0.08]  Winding2Connection=Yg  Winding2=[110000,0.002,0.08]  SetSaturation=off  Rm=500  Lm=500  Saturation=[ 0,0 ; 0.0024,1.2 ; 1.0,1.52 ]  Hysteresis=off  DataFile='hysteresis'  SetInitialFlux=off  InitialFluxes=[ 0.8 , -0.8 , 0.7 ]  Measurements=None  MoreParameters=off  BreakLoop=off  DataType=off  TransfoNumber=1
  T_172445102__ : powerlib/Elements/Three-Phase Transformer (Two Windings)  Winding1Connection=Yg  UNITS=pu  NominalPower=[ 250e6 , 60 ]  Winding1=[110000,0.002,0.08]  Winding2Connection=Yg  Winding2=[110000,0.002,0.08]  SetSaturation=off  Rm=500  Lm=500  Saturation=[ 0,0 ; 0.0024,1.2 ; 1.0,1.52 ]  Hysteresis=off  DataFile='hysteresis'  SetInitialFlux=off  InitialFluxes=[ 0.8 , -0.8 , 0.7 ]  Measurements=None  MoreParameters=off  BreakLoop=off  DataType=off  TransfoNumber=1
  T_172445103__ : powerlib/Elements/Three-Phase Transformer (Two Windings)  Winding1Connection=Yg  UNITS=pu  NominalPower=[ 250e6 , 60 ]  Winding1=[110000,0.002,0.08]  Winding2Connection=Yg  Winding2=[110000,0.002,0.08]  SetSaturation=off  Rm=500  Lm=500  Saturation=[ 0,0 ; 0.0024,1.2 ; 1.0,1.52 ]  Hysteresis=off  DataFile='hysteresis'  SetInitialFlux=off  InitialFluxes=[ 0.8 , -0.8 , 0.7 ]  Measurements=None  MoreParameters=off  BreakLoop=off  DataType=off  TransfoNumber=1
  T_172445107__ : powerlib/Elements/Three-Phase Transformer (Two Windings)  Winding1Connection=Yg  UNITS=pu  NominalPower=[ 250e6 , 60 ]  Winding1=[110000,0.002,0.08]  Winding2Connection=Yg  Winding2=[110000,0.002,0.08]  SetSaturation=off  Rm=500  Lm=500  Saturation=[ 0,0 ; 0.0024,1.2 ; 1.0,1.52 ]  Hysteresis=off  DataFile='hysteresis'  SetInitialFlux=off  InitialFluxes=[ 0.8 , -0.8 , 0.7 ]  Measurements=None  MoreParameters=off  BreakLoop=off  DataType=off  TransfoNumber=1
  T_172590050_330000_ : powerlib/Elements/Three-Phase Transformer (Two Windings)  Winding1Connection=Yg  UNITS=pu  NominalPower=[ 250e6 , 60 ]  Winding1=[330000,0.002,0.08]  Winding2Connection=Yg  Winding2=[330000,0.002,0.08]  SetSaturation=off  Rm=500  Lm=500  Saturation=[ 0,0 ; 0.0024,1.2 ; 1.0,1.52 ]  Hysteresis=off  DataFile='hysteresis'  SetInitialFlux=off  InitialFluxes=[ 0.8 , -0.8 , 0.7 ]  Measurements=None  MoreParameters=off  BreakLoop=off  DataType=off  TransfoNumber=1
  T_172590051__ : powerlib/Elements/Three-Phase Transformer (Two Windings)  Winding1Connection=Yg  UNITS=pu  NominalPower=[ 250e6 , 60 ]  Winding1=[330000,0.002,0.08]  Winding2Connection=Yg  Winding2=[110000,0.002,0.08]  SetSaturation=off  Rm=500  Lm=500  Saturation=[ 0,0 ; 0.0024,1.2 ; 1.0,1.52 ]  Hysteresis=off  DataFile='hysteresis'  SetInitialFlux=off  InitialFluxes=[ 0.8 , -0.8 , 0.7 ]  Measurements=None  MoreParameters=off  BreakLoop=off  DataType=off  TransfoNumber=1
  T_172590075__Žasmos_TP : powerlib/Elements/Three-Phase Transformer (Two Windings)  Winding1Connection=Yg  UNITS=pu  NominalPower=[ 250e6 , 60 ]  Winding1=[110000,0.002,0.08]  Winding2Connection=Yg  Winding2=[110000,0.002,0.08]  SetSaturation=off  Rm=500  Lm=500  Saturation=[ 0,0 ; 0.0024,1.2 ; 1.0,1.52 ]  Hysteresis=off  DataFile='hysteresis'  SetInitialFlux=off  InitialFluxes=[ 0.8 , -0.8 , 0.7 ]  Measurements=None  MoreParameters=off  BreakLoop=off  DataType=off  TransfoNumber=1
  T_172590076__ : powerlib/Elements/Three-Phase Transformer (Two Windings)  Winding1Connection=Yg  UNITS=pu  NominalPower=[ 250e6 , 60 ]  Winding1=[110000,0.002,0.08]  Winding2Connection=Yg  Winding2=[110000,0.002,0.08]  SetSaturation=off  Rm=500  Lm=500  Saturation=[ 0,0 ; 0.0024,1.2 ; 1.0,1.52 ]  Hysteresis=off  DataFile='hysteresis'  SetInitialFlux=off  InitialFluxes=[ 0.8 , -0.8 , 0.7 ]  Measurements=None  MoreParameters=off  BreakLoop=off  DataType=off  TransfoNumber=1
  T_172590080__ : powerlib/Elements/Three-Phase Transformer (Two Windings)  Winding1Connection=Yg  UNITS=pu  NominalPower=[ 250e6 , 60 ]  Winding1=[110000,0.002,0.08]  Winding2Connection=Yg  Winding2=[110000,0.002,0.08]  SetSaturation=off  Rm=500  Lm=500  Saturation=[ 0,0 ; 0.0024,1.2 ; 1.0,1.52 ]  Hysteresis=off  DataFile='hysteresis'  SetInitialFlux=off  InitialFluxes=[ 0.8 , -0.8 , 0.7 ]  Measurements=None  MoreParameters=off  BreakLoop=off  DataType=off  TransfoNumber=1
  T_172590081__ : powerlib/Elements/Three-Phase Transformer (Two Windings)  Winding1Connection=Yg  UNITS=pu  NominalPower=[ 250e6 , 60 ]  Winding1=[110000,0.002,0.08]  Winding2Connection=Yg  Winding2=[110000,0.002,0.08]  SetSaturation=off  Rm=500  Lm=500  Saturation=[ 0,0 ; 0.0024,1.2 ; 1.0,1.52 ]  Hysteresis=off  DataFile='hysteresis'  SetInitialFlux=off  InitialFluxes=[ 0.8 , -0.8 , 0.7 ]  Measurements=None  MoreParameters=off  BreakLoop=off  DataType=off  TransfoNumber=1
  T_172590088__ : powerlib/Elements/Three-Phase Transformer (Two Windings)  Winding1Connection=Yg  UNITS=pu  NominalPower=[ 250e6 , 60 ]  Winding1=[110000,0.002,0.08]  Winding2Connection=Yg  Winding2=[110000,0.002,0.08]  SetSaturation=off  Rm=500  Lm=500  Saturation=[ 0,0 ; 0.0024,1.2 ; 1.0,1.52 ]  Hysteresis=off  DataFile='hysteresis'  SetInitialFlux=off  InitialFluxes=[ 0.8 , -0.8 , 0.7 ]  Measurements=None  MoreParameters=off  BreakLoop=off  DataType=off  TransfoNumber=1
  T_172590095__ : powerlib/Elements/Three-Phase Transformer (Two Windings)  Winding1Connection=Yg  UNITS=pu  NominalPower=[ 250e6 , 60 ]  Winding1=[110000,0.002,0.08]  Winding2Connection=Yg  Winding2=[110000,0.002,0.08]  SetSaturation=off  Rm=500  Lm=500  Saturation=[ 0,0 ; 0.0024,1.2 ; 1.0,1.52 ]  Hysteresis=off  DataFile='hysteresis'  SetInitialFlux=off  InitialFluxes=[ 0.8 , -0.8 , 0.7 ]  Measurements=None  MoreParameters=off  BreakLoop=off  DataType=off  TransfoNumber=1
  T_172590096__ : powerlib/Elements/Three-Phase Transformer (Two Windings)  Winding1Connection=Yg  UNITS=pu  NominalPower=[ 250e6 , 60 ]  Winding1=[110000,0.002,0.08]  Winding2Connection=Yg  Winding2=[110000,0.002,0.08]  SetSaturation=off  Rm=500  Lm=500  Saturation=[ 0,0 ; 0.0024,1.2 ; 1.0,1.52 ]  Hysteresis=off  DataFile='hysteresis'  SetInitialFlux=off  InitialFluxes=[ 0.8 , -0.8 , 0.7 ]  Measurements=None  MoreParameters=off  BreakLoop=off  DataType=off  TransfoNumber=1
  T_172590097__ : powerlib/Elements/Three-Phase Transformer (Two Windings)  Winding1Connection=Yg  UNITS=pu  NominalPower=[ 250e6 , 60 ]  Winding1=[110000,0.002,0.08]  Winding2Connection=Yg  Winding2=[110000,0.002,0.08]  SetSaturation=off  Rm=500  Lm=500  Saturation=[ 0,0 ; 0.0024,1.2 ; 1.0,1.52 ]  Hysteresis=off  DataFile='hysteresis'  SetInitialFlux=off  InitialFluxes=[ 0.8 , -0.8 , 0.7 ]  Measurements=None  MoreParameters=off  BreakLoop=off  DataType=off  TransfoNumber=1
  T_172590098__Drobės_TP : powerlib/Elements/Three-Phase Transformer (Two Windings)  Winding1Connection=Yg  UNITS=pu  NominalPower=[ 250e6 , 60 ]  Winding1=[110000,0.002,0.08]  Winding2Connection=Yg  Winding2=[110000,0.002,0.08]  SetSaturation=off  Rm=500  Lm=500  Saturation=[ 0,0 ; 0.0024,1.2 ; 1.0,1.52 ]  Hysteresis=off  DataFile='hysteresis'  SetInitialFlux=off  InitialFluxes=[ 0.8 , -0.8 , 0.7 ]  Measurements=None  MoreParameters=off  BreakLoop=off  DataType=off  TransfoNumber=1
  T_172590100__Rokų_TP : powerlib/Elements/Three-Phase Transformer (Two Windings)  Winding1Connection=Yg  UNITS=pu  NominalPower=[ 250e6 , 60 ]  Winding1=[110000,0.002,0.08]  Winding2Connection=Yg  Winding2=[110000,0.002,0.08]  SetSaturation=off  Rm=500  Lm=500  Saturation=[ 0,0 ; 0.0024,1.2 ; 1.0,1.52 ]  Hysteresis=off  DataFile='hysteresis'  SetInitialFlux=off  InitialFluxes=[ 0.8 , -0.8 , 0.7 ]  Measurements=None  MoreParameters=off  BreakLoop=off  DataType=off  TransfoNumber=1
  T_172590101__Petrašiūnų_TP : powerlib/Elements/Three-Phase Transformer (Two Windings)  Winding1Connection=Yg  UNITS=pu  NominalPower=[ 250e6 , 60 ]  Winding1=[110000,0.002,0.08]  Winding2Connection=Yg  Winding2=[110000,0.002,0.08]  SetSaturation=off  Rm=500  Lm=500  Saturation=[ 0,0 ; 0.0024,1.2 ; 1.0,1.52 ]  Hysteresis=off  DataFile='hysteresis'  SetInitialFlux=off  InitialFluxes=[ 0.8 , -0.8 , 0.7 ]  Measurements=None  MoreParameters=off  BreakLoop=off  DataType=off  TransfoNumber=1
  T_172590105__Ketaus_TP : powerlib/Elements/Three-Phase Transformer (Two Windings)  Winding1Connection=Yg  UNITS=pu  NominalPower=[ 250e6 , 60 ]  Winding1=[110000,0.002,0.08]  Winding2Connection=Yg  Winding2=[110000,0.002,0.08]  SetSaturation=off  Rm=500  Lm=500  Saturation=[ 0,0 ; 0.0024,1.2 ; 1.0,1.52 ]  Hysteresis=off  DataFile='hysteresis'  SetInitialFlux=off  InitialFluxes=[ 0.8 , -0.8 , 0.7 ]  Measurements=None  MoreParameters=off  BreakLoop=off  DataType=off  TransfoNumber=1
  T_172590108__ : powerlib/Elements/Three-Phase Transformer (Two Windings)  Winding1Connection=Yg  UNITS=pu  NominalPower=[ 250e6 , 60 ]  Winding1=[110000,0.002,0.08]  Winding2Connection=Yg  Winding2=[110000,0.002,0.08]  SetSaturation=off  Rm=500  Lm=500  Saturation=[ 0,0 ; 0.0024,1.2 ; 1.0,1.52 ]  Hysteresis=off  DataFile='hysteresis'  SetInitialFlux=off  InitialFluxes=[ 0.8 , -0.8 , 0.7 ]  Measurements=None  MoreParameters=off  BreakLoop=off  DataType=off  TransfoNumber=1
  T_172590115_330000;110000;fixme_ : powerlib/Elements/Three-Phase Transformer (Two Windings)  Winding1Connection=Yg  UNITS=pu  NominalPower=[ 250e6 , 60 ]  Winding1=[330000,0.002,0.08]  Winding2Connection=Yg  Winding2=[110000,0.002,0.08]  SetSaturation=off  Rm=500  Lm=500  Saturation=[ 0,0 ; 0.0024,1.2 ; 1.0,1.52 ]  Hysteresis=off  DataFile='hysteresis'  SetInitialFlux=off  InitialFluxes=[ 0.8 , -0.8 , 0.7 ]  Measurements=None  MoreParameters=off  BreakLoop=off  DataType=off  TransfoNumber=1
  T_172590116__ : powerlib/Elements/Three-Phase Transformer (Two Windings)  Winding1Connection=Yg  UNITS=pu  NominalPower=[ 250e6 , 60 ]  Winding1=[110000,0.002,0.08]  Winding2Connection=Yg  Winding2=[110000,0.002,0.08]  SetSaturation=off  Rm=500  Lm=500  Saturation=[ 0,0 ; 0.0024,1.2 ; 1.0,1.52 ]  Hysteresis=off  DataFile='hysteresis'  SetInitialFlux=off  InitialFluxes=[ 0.8 , -0.8 , 0.7 ]  Measurements=None  MoreParameters=off  BreakLoop=off  DataType=off  TransfoNumber=1
  T_172978107__ : powerlib/Elements/Three-Phase Transformer (Two Windings)  Winding1Connection=Yg  UNITS=pu  NominalPower=[ 250e6 , 60 ]  Winding1=[110000,0.002,0.08]  Winding2Connection=Yg  Winding2=[110000,0.002,0.08]  SetSaturation=off  Rm=500  Lm=500  Saturation=[ 0,0 ; 0.0024,1.2 ; 1.0,1.52 ]  Hysteresis=off  DataFile='hysteresis'  SetInitialFlux=off  InitialFluxes=[ 0.8 , -0.8 , 0.7 ]  Measurements=None  MoreParameters=off  BreakLoop=off  DataType=off  TransfoNumber=1
  T_173582215__ : powerlib/Elements/Three-Phase Transformer (Two Windings)  Winding1Connection=Yg  UNITS=pu  NominalPower=[ 250e6 , 60 ]  Winding1=[110000,0.002,0.08]  Winding2Connection=Yg  Winding2=[110000,0.002,0.08]  SetSaturation=off  Rm=500  Lm=500  Saturation=[ 0,0 ; 0.0024,1.2 ; 1.0,1.52 ]  Hysteresis=off  DataFile='hysteresis'  SetInitialFlux=off  InitialFluxes=[ 0.8 , -0.8 , 0.7 ]  Measurements=None  MoreParameters=off  BreakLoop=off  DataType=off  TransfoNumber=1
  T_173582216__ : powerlib/Elements/Three-Phase Transformer (Two Windings)  Winding1Connection=Yg  UNITS=pu  NominalPower=[ 250e6 , 60 ]  Winding1=[110000,0.002,0.08]  Winding2Connection=Yg  Winding2=[110000,0.002,0.08]  SetSaturation=off  Rm=500  Lm=500  Saturation=[ 0,0 ; 0.0024,1.2 ; 1.0,1.52 ]  Hysteresis=off  DataFile='hysteresis'  SetInitialFlux=off  InitialFluxes=[ 0.8 , -0.8 , 0.7 ]  Measurements=None  MoreParameters=off  BreakLoop=off  DataType=off  TransfoNumber=1
  T_173582225__ : powerlib/Elements/Three-Phase Transformer (Two Windings)  Winding1Connection=Yg  UNITS=pu  NominalPower=[ 250e6 , 60 ]  Winding1=[110000,0.002,0.08]  Winding2Connection=Yg  Winding2=[110000,0.002,0.08]  SetSaturation=off  Rm=500  Lm=500  Saturation=[ 0,0 ; 0.0024,1.2 ; 1.0,1.52 ]  Hysteresis=off  DataFile='hysteresis'  SetInitialFlux=off  InitialFluxes=[ 0.8 , -0.8 , 0.7 ]  Measurements=None  MoreParameters=off  BreakLoop=off  DataType=off  TransfoNumber=1
  T_173582226__ : powerlib/Elements/Three-Phase Transformer (Two Windings)  Winding1Connection=Yg  UNITS=pu  NominalPower=[ 250e6 , 60 ]  Winding1=[110000,0.002,0.08]  Winding2Connection=Yg  Winding2=[110000,0.002,0.08]  SetSaturation=off  Rm=500  Lm=500  Saturation=[ 0,0 ; 0.0024,1.2 ; 1.0,1.52 ]  Hysteresis=off  DataFile='hysteresis'  SetInitialFlux=off  InitialFluxes=[ 0.8 , -0.8 , 0.7 ]  Measurements=None  MoreParameters=off  BreakLoop=off  DataType=off  TransfoNumber=1
  T_173591498__ : powerlib/Elements/Three-Phase Transformer (Two Windings)  Winding1Connection=Yg  UNITS=pu  NominalPower=[ 250e6 , 60 ]  Winding1=[110000,0.002,0.08]  Winding2Connection=Yg  Winding2=[110000,0.002,0.08]  SetSaturation=off  Rm=500  Lm=500  Saturation=[ 0,0 ; 0.0024,1.2 ; 1.0,1.52 ]  Hysteresis=off  DataFile='hysteresis'  SetInitialFlux=off  InitialFluxes=[ 0.8 , -0.8 , 0.7 ]  Measurements=None  MoreParameters=off  BreakLoop=off  DataType=off  TransfoNumber=1
  T_173591500__ : powerlib/Elements/Three-Phase Transformer (Two Windings)  Winding1Connection=Yg  UNITS=pu  NominalPower=[ 250e6 , 60 ]  Winding1=[110000,0.002,0.08]  Winding2Connection=Yg  Winding2=[110000,0.002,0.08]  SetSaturation=off  Rm=500  Lm=500  Saturation=[ 0,0 ; 0.0024,1.2 ; 1.0,1.52 ]  Hysteresis=off  DataFile='hysteresis'  SetInitialFlux=off  InitialFluxes=[ 0.8 , -0.8 , 0.7 ]  Measurements=None  MoreParameters=off  BreakLoop=off  DataType=off  TransfoNumber=1
  T_173591502__ : powerlib/Elements/Three-Phase Transformer (Two Windings)  Winding1Connection=Yg  UNITS=pu  NominalPower=[ 250e6 , 60 ]  Winding1=[110000,0.002,0.08]  Winding2Connection=Yg  Winding2=[110000,0.002,0.08]  SetSaturation=off  Rm=500  Lm=500  Saturation=[ 0,0 ; 0.0024,1.2 ; 1.0,1.52 ]  Hysteresis=off  DataFile='hysteresis'  SetInitialFlux=off  InitialFluxes=[ 0.8 , -0.8 , 0.7 ]  Measurements=None  MoreParameters=off  BreakLoop=off  DataType=off  TransfoNumber=1
  T_173593029__Šilko_TP : powerlib/Elements/Three-Phase Transformer (Two Windings)  Winding1Connection=Yg  UNITS=pu  NominalPower=[ 250e6 , 60 ]  Winding1=[110000,0.002,0.08]  Winding2Connection=Yg  Winding2=[110000,0.002,0.08]  SetSaturation=off  Rm=500  Lm=500  Saturation=[ 0,0 ; 0.0024,1.2 ; 1.0,1.52 ]  Hysteresis=off  DataFile='hysteresis'  SetInitialFlux=off  InitialFluxes=[ 0.8 , -0.8 , 0.7 ]  Measurements=None  MoreParameters=off  BreakLoop=off  DataType=off  TransfoNumber=1
  T_173612890__Garliavos_TP : powerlib/Elements/Three-Phase Transformer (Two Windings)  Winding1Connection=Yg  UNITS=pu  NominalPower=[ 250e6 , 60 ]  Winding1=[110000,0.002,0.08]  Winding2Connection=Yg  Winding2=[110000,0.002,0.08]  SetSaturation=off  Rm=500  Lm=500  Saturation=[ 0,0 ; 0.0024,1.2 ; 1.0,1.52 ]  Hysteresis=off  DataFile='hysteresis'  SetInitialFlux=off  InitialFluxes=[ 0.8 , -0.8 , 0.7 ]  Measurements=None  MoreParameters=off  BreakLoop=off  DataType=off  TransfoNumber=1
  T_173765447__Pluošto_TP : powerlib/Elements/Three-Phase Transformer (Two Windings)  Winding1Connection=Yg  UNITS=pu  NominalPower=[ 250e6 , 60 ]  Winding1=[110000,0.002,0.08]  Winding2Connection=Yg  Winding2=[110000,0.002,0.08]  SetSaturation=off  Rm=500  Lm=500  Saturation=[ 0,0 ; 0.0024,1.2 ; 1.0,1.52 ]  Hysteresis=off  DataFile='hysteresis'  SetInitialFlux=off  InitialFluxes=[ 0.8 , -0.8 , 0.7 ]  Measurements=None  MoreParameters=off  BreakLoop=off  DataType=off  TransfoNumber=1
  T_173944045__ : powerlib/Elements/Three-Phase Transformer (Two Windings)  Winding1Connection=Yg  UNITS=pu  NominalPower=[ 250e6 , 60 ]  Winding1=[110000,0.002,0.08]  Winding2Connection=Yg  Winding2=[110000,0.002,0.08]  SetSaturation=off  Rm=500  Lm=500  Saturation=[ 0,0 ; 0.0024,1.2 ; 1.0,1.52 ]  Hysteresis=off  DataFile='hysteresis'  SetInitialFlux=off  InitialFluxes=[ 0.8 , -0.8 , 0.7 ]  Measurements=None  MoreParameters=off  BreakLoop=off  DataType=off  TransfoNumber=1
  T_173944047__ : powerlib/Elements/Three-Phase Transformer (Two Windings)  Winding1Connection=Yg  UNITS=pu  NominalPower=[ 250e6 , 60 ]  Winding1=[110000,0.002,0.08]  Winding2Connection=Yg  Winding2=[110000,0.002,0.08]  SetSaturation=off  Rm=500  Lm=500  Saturation=[ 0,0 ; 0.0024,1.2 ; 1.0,1.52 ]  Hysteresis=off  DataFile='hysteresis'  SetInitialFlux=off  InitialFluxes=[ 0.8 , -0.8 , 0.7 ]  Measurements=None  MoreParameters=off  BreakLoop=off  DataType=off  TransfoNumber=1
  T_173944055__ : powerlib/Elements/Three-Phase Transformer (Two Windings)  Winding1Connection=Yg  UNITS=pu  NominalPower=[ 250e6 , 60 ]  Winding1=[110000,0.002,0.08]  Winding2Connection=Yg  Winding2=[110000,0.002,0.08]  SetSaturation=off  Rm=500  Lm=500  Saturation=[ 0,0 ; 0.0024,1.2 ; 1.0,1.52 ]  Hysteresis=off  DataFile='hysteresis'  SetInitialFlux=off  InitialFluxes=[ 0.8 , -0.8 , 0.7 ]  Measurements=None  MoreParameters=off  BreakLoop=off  DataType=off  TransfoNumber=1
  T_173944056__ : powerlib/Elements/Three-Phase Transformer (Two Windings)  Winding1Connection=Yg  UNITS=pu  NominalPower=[ 250e6 , 60 ]  Winding1=[110000,0.002,0.08]  Winding2Connection=Yg  Winding2=[110000,0.002,0.08]  SetSaturation=off  Rm=500  Lm=500  Saturation=[ 0,0 ; 0.0024,1.2 ; 1.0,1.52 ]  Hysteresis=off  DataFile='hysteresis'  SetInitialFlux=off  InitialFluxes=[ 0.8 , -0.8 , 0.7 ]  Measurements=None  MoreParameters=off  BreakLoop=off  DataType=off  TransfoNumber=1
  T_173944057__ : powerlib/Elements/Three-Phase Transformer (Two Windings)  Winding1Connection=Yg  UNITS=pu  NominalPower=[ 250e6 , 60 ]  Winding1=[110000,0.002,0.08]  Winding2Connection=Yg  Winding2=[110000,0.002,0.08]  SetSaturation=off  Rm=500  Lm=500  Saturation=[ 0,0 ; 0.0024,1.2 ; 1.0,1.52 ]  Hysteresis=off  DataFile='hysteresis'  SetInitialFlux=off  InitialFluxes=[ 0.8 , -0.8 , 0.7 ]  Measurements=None  MoreParameters=off  BreakLoop=off  DataType=off  TransfoNumber=1
  T_173944061__ : powerlib/Elements/Three-Phase Transformer (Two Windings)  Winding1Connection=Yg  UNITS=pu  NominalPower=[ 250e6 , 60 ]  Winding1=[110000,0.002,0.08]  Winding2Connection=Yg  Winding2=[110000,0.002,0.08]  SetSaturation=off  Rm=500  Lm=500  Saturation=[ 0,0 ; 0.0024,1.2 ; 1.0,1.52 ]  Hysteresis=off  DataFile='hysteresis'  SetInitialFlux=off  InitialFluxes=[ 0.8 , -0.8 , 0.7 ]  Measurements=None  MoreParameters=off  BreakLoop=off  DataType=off  TransfoNumber=1
  T_174045384__ : powerlib/Elements/Three-Phase Transformer (Two Windings)  Winding1Connection=Yg  UNITS=pu  NominalPower=[ 250e6 , 60 ]  Winding1=[110000,0.002,0.08]  Winding2Connection=Yg  Winding2=[110000,0.002,0.08]  SetSaturation=off  Rm=500  Lm=500  Saturation=[ 0,0 ; 0.0024,1.2 ; 1.0,1.52 ]  Hysteresis=off  DataFile='hysteresis'  SetInitialFlux=off  InitialFluxes=[ 0.8 , -0.8 , 0.7 ]  Measurements=None  MoreParameters=off  BreakLoop=off  DataType=off  TransfoNumber=1
  T_174586802__ : powerlib/Elements/Three-Phase Transformer (Two Windings)  Winding1Connection=Yg  UNITS=pu  NominalPower=[ 250e6 , 60 ]  Winding1=[110000,0.002,0.08]  Winding2Connection=Yg  Winding2=[110000,0.002,0.08]  SetSaturation=off  Rm=500  Lm=500  Saturation=[ 0,0 ; 0.0024,1.2 ; 1.0,1.52 ]  Hysteresis=off  DataFile='hysteresis'  SetInitialFlux=off  InitialFluxes=[ 0.8 , -0.8 , 0.7 ]  Measurements=None  MoreParameters=off  BreakLoop=off  DataType=off  TransfoNumber=1
  T_175315244__ : powerlib/Elements/Three-Phase Transformer (Two Windings)  Winding1Connection=Yg  UNITS=pu  NominalPower=[ 250e6 , 60 ]  Winding1=[110000,0.002,0.08]  Winding2Connection=Yg  Winding2=[110000,0.002,0.08]  SetSaturation=off  Rm=500  Lm=500  Saturation=[ 0,0 ; 0.0024,1.2 ; 1.0,1.52 ]  Hysteresis=off  DataFile='hysteresis'  SetInitialFlux=off  InitialFluxes=[ 0.8 , -0.8 , 0.7 ]  Measurements=None  MoreParameters=off  BreakLoop=off  DataType=off  TransfoNumber=1
  T_176323123__ : powerlib/Elements/Three-Phase Transformer (Two Windings)  Winding1Connection=Yg  UNITS=pu  NominalPower=[ 250e6 , 60 ]  Winding1=[110000,0.002,0.08]  Winding2Connection=Yg  Winding2=[110000,0.002,0.08]  SetSaturation=off  Rm=500  Lm=500  Saturation=[ 0,0 ; 0.0024,1.2 ; 1.0,1.52 ]  Hysteresis=off  DataFile='hysteresis'  SetInitialFlux=off  InitialFluxes=[ 0.8 , -0.8 , 0.7 ]  Measurements=None  MoreParameters=off  BreakLoop=off  DataType=off  TransfoNumber=1
  T_181769867__ : powerlib/Elements/Three-Phase Transformer (Two Windings)  Winding1Connection=Yg  UNITS=pu  NominalPower=[ 250e6 , 60 ]  Winding1=[110000,0.002,0.08]  Winding2Connection=Yg  Winding2=[110000,0.002,0.08]  SetSaturation=off  Rm=500  Lm=500  Saturation=[ 0,0 ; 0.0024,1.2 ; 1.0,1.52 ]  Hysteresis=off  DataFile='hysteresis'  SetInitialFlux=off  InitialFluxes=[ 0.8 , -0.8 , 0.7 ]  Measurements=None  MoreParameters=off  BreakLoop=off  DataType=off  TransfoNumber=1
  T_187242275__ : powerlib/Elements/Three-Phase Transformer (Two Windings)  Winding1Connection=Yg  UNITS=pu  NominalPower=[ 250e6 , 60 ]  Winding1=[110000,0.002,0.08]  Winding2Connection=Yg  Winding2=[110000,0.002,0.08]  SetSaturation=off  Rm=500  Lm=500  Saturation=[ 0,0 ; 0.0024,1.2 ; 1.0,1.52 ]  Hysteresis=off  DataFile='hysteresis'  SetInitialFlux=off  InitialFluxes=[ 0.8 , -0.8 , 0.7 ]  Measurements=None  MoreParameters=off  BreakLoop=off  DataType=off  TransfoNumber=1
  T_192646598__ : powerlib/Elements/Three-Phase Transformer (Two Windings)  Winding1Connection=Yg  UNITS=pu  NominalPower=[ 250e6 , 60 ]  Winding1=[110000,0.002,0.08]  Winding2Connection=Yg  Winding2=[110000,0.002,0.08]  SetSaturation=off  Rm=500  Lm=500  Saturation=[ 0,0 ; 0.0024,1.2 ; 1.0,1.52 ]  Hysteresis=off  DataFile='hysteresis'  SetInitialFlux=off  InitialFluxes=[ 0.8 , -0.8 , 0.7 ]  Measurements=None  MoreParameters=off  BreakLoop=off  DataType=off  TransfoNumber=1
  T_192672875__ : powerlib/Elements/Three-Phase Transformer (Two Windings)  Winding1Connection=Yg  UNITS=pu  NominalPower=[ 250e6 , 60 ]  Winding1=[110000,0.002,0.08]  Winding2Connection=Yg  Winding2=[110000,0.002,0.08]  SetSaturation=off  Rm=500  Lm=500  Saturation=[ 0,0 ; 0.0024,1.2 ; 1.0,1.52 ]  Hysteresis=off  DataFile='hysteresis'  SetInitialFlux=off  InitialFluxes=[ 0.8 , -0.8 , 0.7 ]  Measurements=None  MoreParameters=off  BreakLoop=off  DataType=off  TransfoNumber=1
  T_192672898__ : powerlib/Elements/Three-Phase Transformer (Two Windings)  Winding1Connection=Yg  UNITS=pu  NominalPower=[ 250e6 , 60 ]  Winding1=[110000,0.002,0.08]  Winding2Connection=Yg  Winding2=[110000,0.002,0.08]  SetSaturation=off  Rm=500  Lm=500  Saturation=[ 0,0 ; 0.0024,1.2 ; 1.0,1.52 ]  Hysteresis=off  DataFile='hysteresis'  SetInitialFlux=off  InitialFluxes=[ 0.8 , -0.8 , 0.7 ]  Measurements=None  MoreParameters=off  BreakLoop=off  DataType=off  TransfoNumber=1
  T_192672903__ : powerlib/Elements/Three-Phase Transformer (Two Windings)  Winding1Connection=Yg  UNITS=pu  NominalPower=[ 250e6 , 60 ]  Winding1=[110000,0.002,0.08]  Winding2Connection=Yg  Winding2=[110000,0.002,0.08]  SetSaturation=off  Rm=500  Lm=500  Saturation=[ 0,0 ; 0.0024,1.2 ; 1.0,1.52 ]  Hysteresis=off  DataFile='hysteresis'  SetInitialFlux=off  InitialFluxes=[ 0.8 , -0.8 , 0.7 ]  Measurements=None  MoreParameters=off  BreakLoop=off  DataType=off  TransfoNumber=1
  T_192672905__ : powerlib/Elements/Three-Phase Transformer (Two Windings)  Winding1Connection=Yg  UNITS=pu  NominalPower=[ 250e6 , 60 ]  Winding1=[110000,0.002,0.08]  Winding2Connection=Yg  Winding2=[110000,0.002,0.08]  SetSaturation=off  Rm=500  Lm=500  Saturation=[ 0,0 ; 0.0024,1.2 ; 1.0,1.52 ]  Hysteresis=off  DataFile='hysteresis'  SetInitialFlux=off  InitialFluxes=[ 0.8 , -0.8 , 0.7 ]  Measurements=None  MoreParameters=off  BreakLoop=off  DataType=off  TransfoNumber=1
  T_192672914__ : powerlib/Elements/Three-Phase Transformer (Two Windings)  Winding1Connection=Yg  UNITS=pu  NominalPower=[ 250e6 , 60 ]  Winding1=[110000,0.002,0.08]  Winding2Connection=Yg  Winding2=[110000,0.002,0.08]  SetSaturation=off  Rm=500  Lm=500  Saturation=[ 0,0 ; 0.0024,1.2 ; 1.0,1.52 ]  Hysteresis=off  DataFile='hysteresis'  SetInitialFlux=off  InitialFluxes=[ 0.8 , -0.8 , 0.7 ]  Measurements=None  MoreParameters=off  BreakLoop=off  DataType=off  TransfoNumber=1
  T_192677018__ : powerlib/Elements/Three-Phase Transformer (Two Windings)  Winding1Connection=Yg  UNITS=pu  NominalPower=[ 250e6 , 60 ]  Winding1=[110000,0.002,0.08]  Winding2Connection=Yg  Winding2=[110000,0.002,0.08]  SetSaturation=off  Rm=500  Lm=500  Saturation=[ 0,0 ; 0.0024,1.2 ; 1.0,1.52 ]  Hysteresis=off  DataFile='hysteresis'  SetInitialFlux=off  InitialFluxes=[ 0.8 , -0.8 , 0.7 ]  Measurements=None  MoreParameters=off  BreakLoop=off  DataType=off  TransfoNumber=1
  T_192702885__ : powerlib/Elements/Three-Phase Transformer (Two Windings)  Winding1Connection=Yg  UNITS=pu  NominalPower=[ 250e6 , 60 ]  Winding1=[110000,0.002,0.08]  Winding2Connection=Yg  Winding2=[110000,0.002,0.08]  SetSaturation=off  Rm=500  Lm=500  Saturation=[ 0,0 ; 0.0024,1.2 ; 1.0,1.52 ]  Hysteresis=off  DataFile='hysteresis'  SetInitialFlux=off  InitialFluxes=[ 0.8 , -0.8 , 0.7 ]  Measurements=None  MoreParameters=off  BreakLoop=off  DataType=off  TransfoNumber=1
  T_192764283_330000;110000;fixme_ : powerlib/Elements/Three-Phase Transformer (Two Windings)  Winding1Connection=Yg  UNITS=pu  NominalPower=[ 250e6 , 60 ]  Winding1=[330000,0.002,0.08]  Winding2Connection=Yg  Winding2=[110000,0.002,0.08]  SetSaturation=off  Rm=500  Lm=500  Saturation=[ 0,0 ; 0.0024,1.2 ; 1.0,1.52 ]  Hysteresis=off  DataFile='hysteresis'  SetInitialFlux=off  InitialFluxes=[ 0.8 , -0.8 , 0.7 ]  Measurements=None  MoreParameters=off  BreakLoop=off  DataType=off  TransfoNumber=1
  T_192764310__ : powerlib/Elements/Three-Phase Transformer (Two Windings)  Winding1Connection=Yg  UNITS=pu  NominalPower=[ 250e6 , 60 ]  Winding1=[110000,0.002,0.08]  Winding2Connection=Yg  Winding2=[110000,0.002,0.08]  SetSaturation=off  Rm=500  Lm=500  Saturation=[ 0,0 ; 0.0024,1.2 ; 1.0,1.52 ]  Hysteresis=off  DataFile='hysteresis'  SetInitialFlux=off  InitialFluxes=[ 0.8 , -0.8 , 0.7 ]  Measurements=None  MoreParameters=off  BreakLoop=off  DataType=off  TransfoNumber=1
  T_192764316__ : powerlib/Elements/Three-Phase Transformer (Two Windings)  Winding1Connection=Yg  UNITS=pu  NominalPower=[ 250e6 , 60 ]  Winding1=[110000,0.002,0.08]  Winding2Connection=Yg  Winding2=[110000,0.002,0.08]  SetSaturation=off  Rm=500  Lm=500  Saturation=[ 0,0 ; 0.0024,1.2 ; 1.0,1.52 ]  Hysteresis=off  DataFile='hysteresis'  SetInitialFlux=off  InitialFluxes=[ 0.8 , -0.8 , 0.7 ]  Measurements=None  MoreParameters=off  BreakLoop=off  DataType=off  TransfoNumber=1
  T_192764327__ : powerlib/Elements/Three-Phase Transformer (Two Windings)  Winding1Connection=Yg  UNITS=pu  NominalPower=[ 250e6 , 60 ]  Winding1=[110000,0.002,0.08]  Winding2Connection=Yg  Winding2=[110000,0.002,0.08]  SetSaturation=off  Rm=500  Lm=500  Saturation=[ 0,0 ; 0.0024,1.2 ; 1.0,1.52 ]  Hysteresis=off  DataFile='hysteresis'  SetInitialFlux=off  InitialFluxes=[ 0.8 , -0.8 , 0.7 ]  Measurements=None  MoreParameters=off  BreakLoop=off  DataType=off  TransfoNumber=1
  T_192764330__ : powerlib/Elements/Three-Phase Transformer (Two Windings)  Winding1Connection=Yg  UNITS=pu  NominalPower=[ 250e6 , 60 ]  Winding1=[110000,0.002,0.08]  Winding2Connection=Yg  Winding2=[110000,0.002,0.08]  SetSaturation=off  Rm=500  Lm=500  Saturation=[ 0,0 ; 0.0024,1.2 ; 1.0,1.52 ]  Hysteresis=off  DataFile='hysteresis'  SetInitialFlux=off  InitialFluxes=[ 0.8 , -0.8 , 0.7 ]  Measurements=None  MoreParameters=off  BreakLoop=off  DataType=off  TransfoNumber=1
  T_192764331__ : powerlib/Elements/Three-Phase Transformer (Two Windings)  Winding1Connection=Yg  UNITS=pu  NominalPower=[ 250e6 , 60 ]  Winding1=[110000,0.002,0.08]  Winding2Connection=Yg  Winding2=[110000,0.002,0.08]  SetSaturation=off  Rm=500  Lm=500  Saturation=[ 0,0 ; 0.0024,1.2 ; 1.0,1.52 ]  Hysteresis=off  DataFile='hysteresis'  SetInitialFlux=off  InitialFluxes=[ 0.8 , -0.8 , 0.7 ]  Measurements=None  MoreParameters=off  BreakLoop=off  DataType=off  TransfoNumber=1
  T_192764337_110000;fixme_ : powerlib/Elements/Three-Phase Transformer (Two Windings)  Winding1Connection=Yg  UNITS=pu  NominalPower=[ 250e6 , 60 ]  Winding1=[110000,0.002,0.08]  Winding2Connection=Yg  Winding2=[110000,0.002,0.08]  SetSaturation=off  Rm=500  Lm=500  Saturation=[ 0,0 ; 0.0024,1.2 ; 1.0,1.52 ]  Hysteresis=off  DataFile='hysteresis'  SetInitialFlux=off  InitialFluxes=[ 0.8 , -0.8 , 0.7 ]  Measurements=None  MoreParameters=off  BreakLoop=off  DataType=off  TransfoNumber=1
  T_192764347_110000;fixme_ : powerlib/Elements/Three-Phase Transformer (Two Windings)  Winding1Connection=Yg  UNITS=pu  NominalPower=[ 250e6 , 60 ]  Winding1=[110000,0.002,0.08]  Winding2Connection=Yg  Winding2=[110000,0.002,0.08]  SetSaturation=off  Rm=500  Lm=500  Saturation=[ 0,0 ; 0.0024,1.2 ; 1.0,1.52 ]  Hysteresis=off  DataFile='hysteresis'  SetInitialFlux=off  InitialFluxes=[ 0.8 , -0.8 , 0.7 ]  Measurements=None  MoreParameters=off  BreakLoop=off  DataType=off  TransfoNumber=1
  T_194082693__ : powerlib/Elements/Three-Phase Transformer (Two Windings)  Winding1Connection=Yg  UNITS=pu  NominalPower=[ 250e6 , 60 ]  Winding1=[110000,0.002,0.08]  Winding2Connection=Yg  Winding2=[110000,0.002,0.08]  SetSaturation=off  Rm=500  Lm=500  Saturation=[ 0,0 ; 0.0024,1.2 ; 1.0,1.52 ]  Hysteresis=off  DataFile='hysteresis'  SetInitialFlux=off  InitialFluxes=[ 0.8 , -0.8 , 0.7 ]  Measurements=None  MoreParameters=off  BreakLoop=off  DataType=off  TransfoNumber=1
  T_197911127_330000;110000;15000;6000_ПС_330_кВ_«Советск» : powerlib/Elements/Three-Phase Transformer (Two Windings)  Winding1Connection=Yg  UNITS=pu  NominalPower=[ 250e6 , 60 ]  Winding1=[330000,0.002,0.08]  Winding2Connection=Yg  Winding2=[330000,0.002,0.08]  SetSaturation=off  Rm=500  Lm=500  Saturation=[ 0,0 ; 0.0024,1.2 ; 1.0,1.52 ]  Hysteresis=off  DataFile='hysteresis'  SetInitialFlux=off  InitialFluxes=[ 0.8 , -0.8 , 0.7 ]  Measurements=None  MoreParameters=off  BreakLoop=off  DataType=off  TransfoNumber=1
  T_207755729__ : powerlib/Elements/Three-Phase Transformer (Two Windings)  Winding1Connection=Yg  UNITS=pu  NominalPower=[ 250e6 , 60 ]  Winding1=[110000,0.002,0.08]  Winding2Connection=Yg  Winding2=[110000,0.002,0.08]  SetSaturation=off  Rm=500  Lm=500  Saturation=[ 0,0 ; 0.0024,1.2 ; 1.0,1.52 ]  Hysteresis=off  DataFile='hysteresis'  SetInitialFlux=off  InitialFluxes=[ 0.8 , -0.8 , 0.7 ]  Measurements=None  MoreParameters=off  BreakLoop=off  DataType=off  TransfoNumber=1
  T_207755730__ : powerlib/Elements/Three-Phase Transformer (Two Windings)  Winding1Connection=Yg  UNITS=pu  NominalPower=[ 250e6 , 60 ]  Winding1=[110000,0.002,0.08]  Winding2Connection=Yg  Winding2=[110000,0.002,0.08]  SetSaturation=off  Rm=500  Lm=500  Saturation=[ 0,0 ; 0.0024,1.2 ; 1.0,1.52 ]  Hysteresis=off  DataFile='hysteresis'  SetInitialFlux=off  InitialFluxes=[ 0.8 , -0.8 , 0.7 ]  Measurements=None  MoreParameters=off  BreakLoop=off  DataType=off  TransfoNumber=1
  T_209204254__ : powerlib/Elements/Three-Phase Transformer (Two Windings)  Winding1Connection=Yg  UNITS=pu  NominalPower=[ 250e6 , 60 ]  Winding1=[110000,0.002,0.08]  Winding2Connection=Yg  Winding2=[110000,0.002,0.08]  SetSaturation=off  Rm=500  Lm=500  Saturation=[ 0,0 ; 0.0024,1.2 ; 1.0,1.52 ]  Hysteresis=off  DataFile='hysteresis'  SetInitialFlux=off  InitialFluxes=[ 0.8 , -0.8 , 0.7 ]  Measurements=None  MoreParameters=off  BreakLoop=off  DataType=off  TransfoNumber=1
  T_210449206__ : powerlib/Elements/Three-Phase Transformer (Two Windings)  Winding1Connection=Yg  UNITS=pu  NominalPower=[ 250e6 , 60 ]  Winding1=[110000,0.002,0.08]  Winding2Connection=Yg  Winding2=[110000,0.002,0.08]  SetSaturation=off  Rm=500  Lm=500  Saturation=[ 0,0 ; 0.0024,1.2 ; 1.0,1.52 ]  Hysteresis=off  DataFile='hysteresis'  SetInitialFlux=off  InitialFluxes=[ 0.8 , -0.8 , 0.7 ]  Measurements=None  MoreParameters=off  BreakLoop=off  DataType=off  TransfoNumber=1
  T_210457037_330000;110000;10000_ : powerlib/Elements/Three-Phase Transformer (Two Windings)  Winding1Connection=Yg  UNITS=pu  NominalPower=[ 250e6 , 60 ]  Winding1=[110000,0.002,0.08]  Winding2Connection=Yg  Winding2=[110000,0.002,0.08]  SetSaturation=off  Rm=500  Lm=500  Saturation=[ 0,0 ; 0.0024,1.2 ; 1.0,1.52 ]  Hysteresis=off  DataFile='hysteresis'  SetInitialFlux=off  InitialFluxes=[ 0.8 , -0.8 , 0.7 ]  Measurements=None  MoreParameters=off  BreakLoop=off  DataType=off  TransfoNumber=1
  T_210457043__ : powerlib/Elements/Three-Phase Transformer (Two Windings)  Winding1Connection=Yg  UNITS=pu  NominalPower=[ 250e6 , 60 ]  Winding1=[110000,0.002,0.08]  Winding2Connection=Yg  Winding2=[110000,0.002,0.08]  SetSaturation=off  Rm=500  Lm=500  Saturation=[ 0,0 ; 0.0024,1.2 ; 1.0,1.52 ]  Hysteresis=off  DataFile='hysteresis'  SetInitialFlux=off  InitialFluxes=[ 0.8 , -0.8 , 0.7 ]  Measurements=None  MoreParameters=off  BreakLoop=off  DataType=off  TransfoNumber=1
  T_210550993__ : powerlib/Elements/Three-Phase Transformer (Two Windings)  Winding1Connection=Yg  UNITS=pu  NominalPower=[ 250e6 , 60 ]  Winding1=[110000,0.002,0.08]  Winding2Connection=Yg  Winding2=[110000,0.002,0.08]  SetSaturation=off  Rm=500  Lm=500  Saturation=[ 0,0 ; 0.0024,1.2 ; 1.0,1.52 ]  Hysteresis=off  DataFile='hysteresis'  SetInitialFlux=off  InitialFluxes=[ 0.8 , -0.8 , 0.7 ]  Measurements=None  MoreParameters=off  BreakLoop=off  DataType=off  TransfoNumber=1
  T_210551439__ : powerlib/Elements/Three-Phase Transformer (Two Windings)  Winding1Connection=Yg  UNITS=pu  NominalPower=[ 250e6 , 60 ]  Winding1=[110000,0.002,0.08]  Winding2Connection=Yg  Winding2=[110000,0.002,0.08]  SetSaturation=off  Rm=500  Lm=500  Saturation=[ 0,0 ; 0.0024,1.2 ; 1.0,1.52 ]  Hysteresis=off  DataFile='hysteresis'  SetInitialFlux=off  InitialFluxes=[ 0.8 , -0.8 , 0.7 ]  Measurements=None  MoreParameters=off  BreakLoop=off  DataType=off  TransfoNumber=1
  T_210555392_110000;35000;fixme_ : powerlib/Elements/Three-Phase Transformer (Two Windings)  Winding1Connection=Yg  UNITS=pu  NominalPower=[ 250e6 , 60 ]  Winding1=[110000,0.002,0.08]  Winding2Connection=Yg  Winding2=[110000,0.002,0.08]  SetSaturation=off  Rm=500  Lm=500  Saturation=[ 0,0 ; 0.0024,1.2 ; 1.0,1.52 ]  Hysteresis=off  DataFile='hysteresis'  SetInitialFlux=off  InitialFluxes=[ 0.8 , -0.8 , 0.7 ]  Measurements=None  MoreParameters=off  BreakLoop=off  DataType=off  TransfoNumber=1
  T_210557029_110000;35000;fixme_ : powerlib/Elements/Three-Phase Transformer (Two Windings)  Winding1Connection=Yg  UNITS=pu  NominalPower=[ 250e6 , 60 ]  Winding1=[110000,0.002,0.08]  Winding2Connection=Yg  Winding2=[110000,0.002,0.08]  SetSaturation=off  Rm=500  Lm=500  Saturation=[ 0,0 ; 0.0024,1.2 ; 1.0,1.52 ]  Hysteresis=off  DataFile='hysteresis'  SetInitialFlux=off  InitialFluxes=[ 0.8 , -0.8 , 0.7 ]  Measurements=None  MoreParameters=off  BreakLoop=off  DataType=off  TransfoNumber=1
  T_210609525__ : powerlib/Elements/Three-Phase Transformer (Two Windings)  Winding1Connection=Yg  UNITS=pu  NominalPower=[ 250e6 , 60 ]  Winding1=[110000,0.002,0.08]  Winding2Connection=Yg  Winding2=[110000,0.002,0.08]  SetSaturation=off  Rm=500  Lm=500  Saturation=[ 0,0 ; 0.0024,1.2 ; 1.0,1.52 ]  Hysteresis=off  DataFile='hysteresis'  SetInitialFlux=off  InitialFluxes=[ 0.8 , -0.8 , 0.7 ]  Measurements=None  MoreParameters=off  BreakLoop=off  DataType=off  TransfoNumber=1
  T_210612962__ : powerlib/Elements/Three-Phase Transformer (Two Windings)  Winding1Connection=Yg  UNITS=pu  NominalPower=[ 250e6 , 60 ]  Winding1=[110000,0.002,0.08]  Winding2Connection=Yg  Winding2=[110000,0.002,0.08]  SetSaturation=off  Rm=500  Lm=500  Saturation=[ 0,0 ; 0.0024,1.2 ; 1.0,1.52 ]  Hysteresis=off  DataFile='hysteresis'  SetInitialFlux=off  InitialFluxes=[ 0.8 , -0.8 , 0.7 ]  Measurements=None  MoreParameters=off  BreakLoop=off  DataType=off  TransfoNumber=1
  T_210619008__ : powerlib/Elements/Three-Phase Transformer (Two Windings)  Winding1Connection=Yg  UNITS=pu  NominalPower=[ 250e6 , 60 ]  Winding1=[110000,0.002,0.08]  Winding2Connection=Yg  Winding2=[110000,0.002,0.08]  SetSaturation=off  Rm=500  Lm=500  Saturation=[ 0,0 ; 0.0024,1.2 ; 1.0,1.52 ]  Hysteresis=off  DataFile='hysteresis'  SetInitialFlux=off  InitialFluxes=[ 0.8 , -0.8 , 0.7 ]  Measurements=None  MoreParameters=off  BreakLoop=off  DataType=off  TransfoNumber=1
  T_210619011__ : powerlib/Elements/Three-Phase Transformer (Two Windings)  Winding1Connection=Yg  UNITS=pu  NominalPower=[ 250e6 , 60 ]  Winding1=[110000,0.002,0.08]  Winding2Connection=Yg  Winding2=[110000,0.002,0.08]  SetSaturation=off  Rm=500  Lm=500  Saturation=[ 0,0 ; 0.0024,1.2 ; 1.0,1.52 ]  Hysteresis=off  DataFile='hysteresis'  SetInitialFlux=off  InitialFluxes=[ 0.8 , -0.8 , 0.7 ]  Measurements=None  MoreParameters=off  BreakLoop=off  DataType=off  TransfoNumber=1
  T_210995832__ : powerlib/Elements/Three-Phase Transformer (Two Windings)  Winding1Connection=Yg  UNITS=pu  NominalPower=[ 250e6 , 60 ]  Winding1=[110000,0.002,0.08]  Winding2Connection=Yg  Winding2=[110000,0.002,0.08]  SetSaturation=off  Rm=500  Lm=500  Saturation=[ 0,0 ; 0.0024,1.2 ; 1.0,1.52 ]  Hysteresis=off  DataFile='hysteresis'  SetInitialFlux=off  InitialFluxes=[ 0.8 , -0.8 , 0.7 ]  Measurements=None  MoreParameters=off  BreakLoop=off  DataType=off  TransfoNumber=1
  T_212007661_110000;fixme_ : powerlib/Elements/Three-Phase Transformer (Two Windings)  Winding1Connection=Yg  UNITS=pu  NominalPower=[ 250e6 , 60 ]  Winding1=[110000,0.002,0.08]  Winding2Connection=Yg  Winding2=[110000,0.002,0.08]  SetSaturation=off  Rm=500  Lm=500  Saturation=[ 0,0 ; 0.0024,1.2 ; 1.0,1.52 ]  Hysteresis=off  DataFile='hysteresis'  SetInitialFlux=off  InitialFluxes=[ 0.8 , -0.8 , 0.7 ]  Measurements=None  MoreParameters=off  BreakLoop=off  DataType=off  TransfoNumber=1
  T_214227031__ : powerlib/Elements/Three-Phase Transformer (Two Windings)  Winding1Connection=Yg  UNITS=pu  NominalPower=[ 250e6 , 60 ]  Winding1=[110000,0.002,0.08]  Winding2Connection=Yg  Winding2=[110000,0.002,0.08]  SetSaturation=off  Rm=500  Lm=500  Saturation=[ 0,0 ; 0.0024,1.2 ; 1.0,1.52 ]  Hysteresis=off  DataFile='hysteresis'  SetInitialFlux=off  InitialFluxes=[ 0.8 , -0.8 , 0.7 ]  Measurements=None  MoreParameters=off  BreakLoop=off  DataType=off  TransfoNumber=1
  T_214455329__ : powerlib/Elements/Three-Phase Transformer (Two Windings)  Winding1Connection=Yg  UNITS=pu  NominalPower=[ 250e6 , 60 ]  Winding1=[110000,0.002,0.08]  Winding2Connection=Yg  Winding2=[110000,0.002,0.08]  SetSaturation=off  Rm=500  Lm=500  Saturation=[ 0,0 ; 0.0024,1.2 ; 1.0,1.52 ]  Hysteresis=off  DataFile='hysteresis'  SetInitialFlux=off  InitialFluxes=[ 0.8 , -0.8 , 0.7 ]  Measurements=None  MoreParameters=off  BreakLoop=off  DataType=off  TransfoNumber=1
  T_214649879__ : powerlib/Elements/Three-Phase Transformer (Two Windings)  Winding1Connection=Yg  UNITS=pu  NominalPower=[ 250e6 , 60 ]  Winding1=[110000,0.002,0.08]  Winding2Connection=Yg  Winding2=[110000,0.002,0.08]  SetSaturation=off  Rm=500  Lm=500  Saturation=[ 0,0 ; 0.0024,1.2 ; 1.0,1.52 ]  Hysteresis=off  DataFile='hysteresis'  SetInitialFlux=off  InitialFluxes=[ 0.8 , -0.8 , 0.7 ]  Measurements=None  MoreParameters=off  BreakLoop=off  DataType=off  TransfoNumber=1
  T_214649882__ : powerlib/Elements/Three-Phase Transformer (Two Windings)  Winding1Connection=Yg  UNITS=pu  NominalPower=[ 250e6 , 60 ]  Winding1=[110000,0.002,0.08]  Winding2Connection=Yg  Winding2=[110000,0.002,0.08]  SetSaturation=off  Rm=500  Lm=500  Saturation=[ 0,0 ; 0.0024,1.2 ; 1.0,1.52 ]  Hysteresis=off  DataFile='hysteresis'  SetInitialFlux=off  InitialFluxes=[ 0.8 , -0.8 , 0.7 ]  Measurements=None  MoreParameters=off  BreakLoop=off  DataType=off  TransfoNumber=1
  T_214674623__ : powerlib/Elements/Three-Phase Transformer (Two Windings)  Winding1Connection=Yg  UNITS=pu  NominalPower=[ 250e6 , 60 ]  Winding1=[110000,0.002,0.08]  Winding2Connection=Yg  Winding2=[110000,0.002,0.08]  SetSaturation=off  Rm=500  Lm=500  Saturation=[ 0,0 ; 0.0024,1.2 ; 1.0,1.52 ]  Hysteresis=off  DataFile='hysteresis'  SetInitialFlux=off  InitialFluxes=[ 0.8 , -0.8 , 0.7 ]  Measurements=None  MoreParameters=off  BreakLoop=off  DataType=off  TransfoNumber=1
  T_215632387__ : powerlib/Elements/Three-Phase Transformer (Two Windings)  Winding1Connection=Yg  UNITS=pu  NominalPower=[ 250e6 , 60 ]  Winding1=[110000,0.002,0.08]  Winding2Connection=Yg  Winding2=[110000,0.002,0.08]  SetSaturation=off  Rm=500  Lm=500  Saturation=[ 0,0 ; 0.0024,1.2 ; 1.0,1.52 ]  Hysteresis=off  DataFile='hysteresis'  SetInitialFlux=off  InitialFluxes=[ 0.8 , -0.8 , 0.7 ]  Measurements=None  MoreParameters=off  BreakLoop=off  DataType=off  TransfoNumber=1
  T_215671382__ : powerlib/Elements/Three-Phase Transformer (Two Windings)  Winding1Connection=Yg  UNITS=pu  NominalPower=[ 250e6 , 60 ]  Winding1=[110000,0.002,0.08]  Winding2Connection=Yg  Winding2=[110000,0.002,0.08]  SetSaturation=off  Rm=500  Lm=500  Saturation=[ 0,0 ; 0.0024,1.2 ; 1.0,1.52 ]  Hysteresis=off  DataFile='hysteresis'  SetInitialFlux=off  InitialFluxes=[ 0.8 , -0.8 , 0.7 ]  Measurements=None  MoreParameters=off  BreakLoop=off  DataType=off  TransfoNumber=1
  T_217323242__ : powerlib/Elements/Three-Phase Transformer (Two Windings)  Winding1Connection=Yg  UNITS=pu  NominalPower=[ 250e6 , 60 ]  Winding1=[110000,0.002,0.08]  Winding2Connection=Yg  Winding2=[110000,0.002,0.08]  SetSaturation=off  Rm=500  Lm=500  Saturation=[ 0,0 ; 0.0024,1.2 ; 1.0,1.52 ]  Hysteresis=off  DataFile='hysteresis'  SetInitialFlux=off  InitialFluxes=[ 0.8 , -0.8 , 0.7 ]  Measurements=None  MoreParameters=off  BreakLoop=off  DataType=off  TransfoNumber=1
  T_217391080__ : powerlib/Elements/Three-Phase Transformer (Two Windings)  Winding1Connection=Yg  UNITS=pu  NominalPower=[ 250e6 , 60 ]  Winding1=[110000,0.002,0.08]  Winding2Connection=Yg  Winding2=[110000,0.002,0.08]  SetSaturation=off  Rm=500  Lm=500  Saturation=[ 0,0 ; 0.0024,1.2 ; 1.0,1.52 ]  Hysteresis=off  DataFile='hysteresis'  SetInitialFlux=off  InitialFluxes=[ 0.8 , -0.8 , 0.7 ]  Measurements=None  MoreParameters=off  BreakLoop=off  DataType=off  TransfoNumber=1
  T_218047622__ : powerlib/Elements/Three-Phase Transformer (Two Windings)  Winding1Connection=Yg  UNITS=pu  NominalPower=[ 250e6 , 60 ]  Winding1=[110000,0.002,0.08]  Winding2Connection=Yg  Winding2=[110000,0.002,0.08]  SetSaturation=off  Rm=500  Lm=500  Saturation=[ 0,0 ; 0.0024,1.2 ; 1.0,1.52 ]  Hysteresis=off  DataFile='hysteresis'  SetInitialFlux=off  InitialFluxes=[ 0.8 , -0.8 , 0.7 ]  Measurements=None  MoreParameters=off  BreakLoop=off  DataType=off  TransfoNumber=1
  T_218214432__ : powerlib/Elements/Three-Phase Transformer (Two Windings)  Winding1Connection=Yg  UNITS=pu  NominalPower=[ 250e6 , 60 ]  Winding1=[110000,0.002,0.08]  Winding2Connection=Yg  Winding2=[110000,0.002,0.08]  SetSaturation=off  Rm=500  Lm=500  Saturation=[ 0,0 ; 0.0024,1.2 ; 1.0,1.52 ]  Hysteresis=off  DataFile='hysteresis'  SetInitialFlux=off  InitialFluxes=[ 0.8 , -0.8 , 0.7 ]  Measurements=None  MoreParameters=off  BreakLoop=off  DataType=off  TransfoNumber=1
  T_218216075_110000;35000;10000_ : powerlib/Elements/Three-Phase Transformer (Two Windings)  Winding1Connection=Yg  UNITS=pu  NominalPower=[ 250e6 , 60 ]  Winding1=[110000,0.002,0.08]  Winding2Connection=Yg  Winding2=[110000,0.002,0.08]  SetSaturation=off  Rm=500  Lm=500  Saturation=[ 0,0 ; 0.0024,1.2 ; 1.0,1.52 ]  Hysteresis=off  DataFile='hysteresis'  SetInitialFlux=off  InitialFluxes=[ 0.8 , -0.8 , 0.7 ]  Measurements=None  MoreParameters=off  BreakLoop=off  DataType=off  TransfoNumber=1
  T_218223015__ : powerlib/Elements/Three-Phase Transformer (Two Windings)  Winding1Connection=Yg  UNITS=pu  NominalPower=[ 250e6 , 60 ]  Winding1=[110000,0.002,0.08]  Winding2Connection=Yg  Winding2=[110000,0.002,0.08]  SetSaturation=off  Rm=500  Lm=500  Saturation=[ 0,0 ; 0.0024,1.2 ; 1.0,1.52 ]  Hysteresis=off  DataFile='hysteresis'  SetInitialFlux=off  InitialFluxes=[ 0.8 , -0.8 , 0.7 ]  Measurements=None  MoreParameters=off  BreakLoop=off  DataType=off  TransfoNumber=1
  T_218223016__ : powerlib/Elements/Three-Phase Transformer (Two Windings)  Winding1Connection=Yg  UNITS=pu  NominalPower=[ 250e6 , 60 ]  Winding1=[110000,0.002,0.08]  Winding2Connection=Yg  Winding2=[110000,0.002,0.08]  SetSaturation=off  Rm=500  Lm=500  Saturation=[ 0,0 ; 0.0024,1.2 ; 1.0,1.52 ]  Hysteresis=off  DataFile='hysteresis'  SetInitialFlux=off  InitialFluxes=[ 0.8 , -0.8 , 0.7 ]  Measurements=None  MoreParameters=off  BreakLoop=off  DataType=off  TransfoNumber=1
  T_219077432_110000;fixme_ : powerlib/Elements/Three-Phase Transformer (Two Windings)  Winding1Connection=Yg  UNITS=pu  NominalPower=[ 250e6 , 60 ]  Winding1=[110000,0.002,0.08]  Winding2Connection=Yg  Winding2=[110000,0.002,0.08]  SetSaturation=off  Rm=500  Lm=500  Saturation=[ 0,0 ; 0.0024,1.2 ; 1.0,1.52 ]  Hysteresis=off  DataFile='hysteresis'  SetInitialFlux=off  InitialFluxes=[ 0.8 , -0.8 , 0.7 ]  Measurements=None  MoreParameters=off  BreakLoop=off  DataType=off  TransfoNumber=1
  T_219084048__ : powerlib/Elements/Three-Phase Transformer (Two Windings)  Winding1Connection=Yg  UNITS=pu  NominalPower=[ 250e6 , 60 ]  Winding1=[110000,0.002,0.08]  Winding2Connection=Yg  Winding2=[110000,0.002,0.08]  SetSaturation=off  Rm=500  Lm=500  Saturation=[ 0,0 ; 0.0024,1.2 ; 1.0,1.52 ]  Hysteresis=off  DataFile='hysteresis'  SetInitialFlux=off  InitialFluxes=[ 0.8 , -0.8 , 0.7 ]  Measurements=None  MoreParameters=off  BreakLoop=off  DataType=off  TransfoNumber=1
  T_220065689__ : powerlib/Elements/Three-Phase Transformer (Two Windings)  Winding1Connection=Yg  UNITS=pu  NominalPower=[ 250e6 , 60 ]  Winding1=[330000,0.002,0.08]  Winding2Connection=Yg  Winding2=[330000,0.002,0.08]  SetSaturation=off  Rm=500  Lm=500  Saturation=[ 0,0 ; 0.0024,1.2 ; 1.0,1.52 ]  Hysteresis=off  DataFile='hysteresis'  SetInitialFlux=off  InitialFluxes=[ 0.8 , -0.8 , 0.7 ]  Measurements=None  MoreParameters=off  BreakLoop=off  DataType=off  TransfoNumber=1
  T_220065702__ : powerlib/Elements/Three-Phase Transformer (Two Windings)  Winding1Connection=Yg  UNITS=pu  NominalPower=[ 250e6 , 60 ]  Winding1=[110000,0.002,0.08]  Winding2Connection=Yg  Winding2=[110000,0.002,0.08]  SetSaturation=off  Rm=500  Lm=500  Saturation=[ 0,0 ; 0.0024,1.2 ; 1.0,1.52 ]  Hysteresis=off  DataFile='hysteresis'  SetInitialFlux=off  InitialFluxes=[ 0.8 , -0.8 , 0.7 ]  Measurements=None  MoreParameters=off  BreakLoop=off  DataType=off  TransfoNumber=1
  T_220915873__ : powerlib/Elements/Three-Phase Transformer (Two Windings)  Winding1Connection=Yg  UNITS=pu  NominalPower=[ 250e6 , 60 ]  Winding1=[110000,0.002,0.08]  Winding2Connection=Yg  Winding2=[110000,0.002,0.08]  SetSaturation=off  Rm=500  Lm=500  Saturation=[ 0,0 ; 0.0024,1.2 ; 1.0,1.52 ]  Hysteresis=off  DataFile='hysteresis'  SetInitialFlux=off  InitialFluxes=[ 0.8 , -0.8 , 0.7 ]  Measurements=None  MoreParameters=off  BreakLoop=off  DataType=off  TransfoNumber=1
  T_220986987__ : powerlib/Elements/Three-Phase Transformer (Two Windings)  Winding1Connection=Yg  UNITS=pu  NominalPower=[ 250e6 , 60 ]  Winding1=[110000,0.002,0.08]  Winding2Connection=Yg  Winding2=[110000,0.002,0.08]  SetSaturation=off  Rm=500  Lm=500  Saturation=[ 0,0 ; 0.0024,1.2 ; 1.0,1.52 ]  Hysteresis=off  DataFile='hysteresis'  SetInitialFlux=off  InitialFluxes=[ 0.8 , -0.8 , 0.7 ]  Measurements=None  MoreParameters=off  BreakLoop=off  DataType=off  TransfoNumber=1
  T_220989437__ : powerlib/Elements/Three-Phase Transformer (Two Windings)  Winding1Connection=Yg  UNITS=pu  NominalPower=[ 250e6 , 60 ]  Winding1=[110000,0.002,0.08]  Winding2Connection=Yg  Winding2=[110000,0.002,0.08]  SetSaturation=off  Rm=500  Lm=500  Saturation=[ 0,0 ; 0.0024,1.2 ; 1.0,1.52 ]  Hysteresis=off  DataFile='hysteresis'  SetInitialFlux=off  InitialFluxes=[ 0.8 , -0.8 , 0.7 ]  Measurements=None  MoreParameters=off  BreakLoop=off  DataType=off  TransfoNumber=1
  T_221105370__ : powerlib/Elements/Three-Phase Transformer (Two Windings)  Winding1Connection=Yg  UNITS=pu  NominalPower=[ 250e6 , 60 ]  Winding1=[110000,0.002,0.08]  Winding2Connection=Yg  Winding2=[110000,0.002,0.08]  SetSaturation=off  Rm=500  Lm=500  Saturation=[ 0,0 ; 0.0024,1.2 ; 1.0,1.52 ]  Hysteresis=off  DataFile='hysteresis'  SetInitialFlux=off  InitialFluxes=[ 0.8 , -0.8 , 0.7 ]  Measurements=None  MoreParameters=off  BreakLoop=off  DataType=off  TransfoNumber=1
  T_226292390__ : powerlib/Elements/Three-Phase Transformer (Two Windings)  Winding1Connection=Yg  UNITS=pu  NominalPower=[ 250e6 , 60 ]  Winding1=[110000,0.002,0.08]  Winding2Connection=Yg  Winding2=[110000,0.002,0.08]  SetSaturation=off  Rm=500  Lm=500  Saturation=[ 0,0 ; 0.0024,1.2 ; 1.0,1.52 ]  Hysteresis=off  DataFile='hysteresis'  SetInitialFlux=off  InitialFluxes=[ 0.8 , -0.8 , 0.7 ]  Measurements=None  MoreParameters=off  BreakLoop=off  DataType=off  TransfoNumber=1
  T_231990061__ : powerlib/Elements/Three-Phase Transformer (Two Windings)  Winding1Connection=Yg  UNITS=pu  NominalPower=[ 250e6 , 60 ]  Winding1=[110000,0.002,0.08]  Winding2Connection=Yg  Winding2=[110000,0.002,0.08]  SetSaturation=off  Rm=500  Lm=500  Saturation=[ 0,0 ; 0.0024,1.2 ; 1.0,1.52 ]  Hysteresis=off  DataFile='hysteresis'  SetInitialFlux=off  InitialFluxes=[ 0.8 , -0.8 , 0.7 ]  Measurements=None  MoreParameters=off  BreakLoop=off  DataType=off  TransfoNumber=1
  T_239589747_110000;fixme_ : powerlib/Elements/Three-Phase Transformer (Two Windings)  Winding1Connection=Yg  UNITS=pu  NominalPower=[ 250e6 , 60 ]  Winding1=[110000,0.002,0.08]  Winding2Connection=Yg  Winding2=[110000,0.002,0.08]  SetSaturation=off  Rm=500  Lm=500  Saturation=[ 0,0 ; 0.0024,1.2 ; 1.0,1.52 ]  Hysteresis=off  DataFile='hysteresis'  SetInitialFlux=off  InitialFluxes=[ 0.8 , -0.8 , 0.7 ]  Measurements=None  MoreParameters=off  BreakLoop=off  DataType=off  TransfoNumber=1
  T_243085462__ : powerlib/Elements/Three-Phase Transformer (Two Windings)  Winding1Connection=Yg  UNITS=pu  NominalPower=[ 250e6 , 60 ]  Winding1=[110000,0.002,0.08]  Winding2Connection=Yg  Winding2=[110000,0.002,0.08]  SetSaturation=off  Rm=500  Lm=500  Saturation=[ 0,0 ; 0.0024,1.2 ; 1.0,1.52 ]  Hysteresis=off  DataFile='hysteresis'  SetInitialFlux=off  InitialFluxes=[ 0.8 , -0.8 , 0.7 ]  Measurements=None  MoreParameters=off  BreakLoop=off  DataType=off  TransfoNumber=1
  T_25698690__330kV_skirstymo_pastotė : powerlib/Elements/Three-Phase Transformer (Two Windings)  Winding1Connection=Yg  UNITS=pu  NominalPower=[ 250e6 , 60 ]  Winding1=[330000,0.002,0.08]  Winding2Connection=Yg  Winding2=[110000,0.002,0.08]  SetSaturation=off  Rm=500  Lm=500  Saturation=[ 0,0 ; 0.0024,1.2 ; 1.0,1.52 ]  Hysteresis=off  DataFile='hysteresis'  SetInitialFlux=off  InitialFluxes=[ 0.8 , -0.8 , 0.7 ]  Measurements=None  MoreParameters=off  BreakLoop=off  DataType=off  TransfoNumber=1
  T_257169562__Kauno_transformatorinė_pastotė : powerlib/Elements/Three-Phase Transformer (Two Windings)  Winding1Connection=Yg  UNITS=pu  NominalPower=[ 250e6 , 60 ]  Winding1=[330000,0.002,0.08]  Winding2Connection=Yg  Winding2=[110000,0.002,0.08]  SetSaturation=off  Rm=500  Lm=500  Saturation=[ 0,0 ; 0.0024,1.2 ; 1.0,1.52 ]  Hysteresis=off  DataFile='hysteresis'  SetInitialFlux=off  InitialFluxes=[ 0.8 , -0.8 , 0.7 ]  Measurements=None  MoreParameters=off  BreakLoop=off  DataType=off  TransfoNumber=1
  T_257169563__ : powerlib/Elements/Three-Phase Transformer (Two Windings)  Winding1Connection=Yg  UNITS=pu  NominalPower=[ 250e6 , 60 ]  Winding1=[330000,0.002,0.08]  Winding2Connection=Yg  Winding2=[110000,0.002,0.08]  SetSaturation=off  Rm=500  Lm=500  Saturation=[ 0,0 ; 0.0024,1.2 ; 1.0,1.52 ]  Hysteresis=off  DataFile='hysteresis'  SetInitialFlux=off  InitialFluxes=[ 0.8 , -0.8 , 0.7 ]  Measurements=None  MoreParameters=off  BreakLoop=off  DataType=off  TransfoNumber=1
  T_257507721__ : powerlib/Elements/Three-Phase Transformer (Two Windings)  Winding1Connection=Yg  UNITS=pu  NominalPower=[ 250e6 , 60 ]  Winding1=[110000,0.002,0.08]  Winding2Connection=Yg  Winding2=[110000,0.002,0.08]  SetSaturation=off  Rm=500  Lm=500  Saturation=[ 0,0 ; 0.0024,1.2 ; 1.0,1.52 ]  Hysteresis=off  DataFile='hysteresis'  SetInitialFlux=off  InitialFluxes=[ 0.8 , -0.8 , 0.7 ]  Measurements=None  MoreParameters=off  BreakLoop=off  DataType=off  TransfoNumber=1
  T_257684864__ : powerlib/Elements/Three-Phase Transformer (Two Windings)  Winding1Connection=Yg  UNITS=pu  NominalPower=[ 250e6 , 60 ]  Winding1=[110000,0.002,0.08]  Winding2Connection=Yg  Winding2=[110000,0.002,0.08]  SetSaturation=off  Rm=500  Lm=500  Saturation=[ 0,0 ; 0.0024,1.2 ; 1.0,1.52 ]  Hysteresis=off  DataFile='hysteresis'  SetInitialFlux=off  InitialFluxes=[ 0.8 , -0.8 , 0.7 ]  Measurements=None  MoreParameters=off  BreakLoop=off  DataType=off  TransfoNumber=1
  T_257684865__ : powerlib/Elements/Three-Phase Transformer (Two Windings)  Winding1Connection=Yg  UNITS=pu  NominalPower=[ 250e6 , 60 ]  Winding1=[110000,0.002,0.08]  Winding2Connection=Yg  Winding2=[110000,0.002,0.08]  SetSaturation=off  Rm=500  Lm=500  Saturation=[ 0,0 ; 0.0024,1.2 ; 1.0,1.52 ]  Hysteresis=off  DataFile='hysteresis'  SetInitialFlux=off  InitialFluxes=[ 0.8 , -0.8 , 0.7 ]  Measurements=None  MoreParameters=off  BreakLoop=off  DataType=off  TransfoNumber=1
  T_258321412__ : powerlib/Elements/Three-Phase Transformer (Two Windings)  Winding1Connection=Yg  UNITS=pu  NominalPower=[ 250e6 , 60 ]  Winding1=[330000,0.002,0.08]  Winding2Connection=Yg  Winding2=[110000,0.002,0.08]  SetSaturation=off  Rm=500  Lm=500  Saturation=[ 0,0 ; 0.0024,1.2 ; 1.0,1.52 ]  Hysteresis=off  DataFile='hysteresis'  SetInitialFlux=off  InitialFluxes=[ 0.8 , -0.8 , 0.7 ]  Measurements=None  MoreParameters=off  BreakLoop=off  DataType=off  TransfoNumber=1
  T_260552752_110000;35000;10000_ : powerlib/Elements/Three-Phase Transformer (Two Windings)  Winding1Connection=Yg  UNITS=pu  NominalPower=[ 250e6 , 60 ]  Winding1=[110000,0.002,0.08]  Winding2Connection=Yg  Winding2=[110000,0.002,0.08]  SetSaturation=off  Rm=500  Lm=500  Saturation=[ 0,0 ; 0.0024,1.2 ; 1.0,1.52 ]  Hysteresis=off  DataFile='hysteresis'  SetInitialFlux=off  InitialFluxes=[ 0.8 , -0.8 , 0.7 ]  Measurements=None  MoreParameters=off  BreakLoop=off  DataType=off  TransfoNumber=1
  T_265807988__ : powerlib/Elements/Three-Phase Transformer (Two Windings)  Winding1Connection=Yg  UNITS=pu  NominalPower=[ 250e6 , 60 ]  Winding1=[110000,0.002,0.08]  Winding2Connection=Yg  Winding2=[110000,0.002,0.08]  SetSaturation=off  Rm=500  Lm=500  Saturation=[ 0,0 ; 0.0024,1.2 ; 1.0,1.52 ]  Hysteresis=off  DataFile='hysteresis'  SetInitialFlux=off  InitialFluxes=[ 0.8 , -0.8 , 0.7 ]  Measurements=None  MoreParameters=off  BreakLoop=off  DataType=off  TransfoNumber=1
  T_268781050_330000_Bitėnai_Elektros_Tiltas : powerlib/Elements/Three-Phase Transformer (Two Windings)  Winding1Connection=Yg  UNITS=pu  NominalPower=[ 250e6 , 60 ]  Winding1=[330000,0.002,0.08]  Winding2Connection=Yg  Winding2=[330000,0.002,0.08]  SetSaturation=off  Rm=500  Lm=500  Saturation=[ 0,0 ; 0.0024,1.2 ; 1.0,1.52 ]  Hysteresis=off  DataFile='hysteresis'  SetInitialFlux=off  InitialFluxes=[ 0.8 , -0.8 , 0.7 ]  Measurements=None  MoreParameters=off  BreakLoop=off  DataType=off  TransfoNumber=1
  T_280078882__ : powerlib/Elements/Three-Phase Transformer (Two Windings)  Winding1Connection=Yg  UNITS=pu  NominalPower=[ 250e6 , 60 ]  Winding1=[110000,0.002,0.08]  Winding2Connection=Yg  Winding2=[110000,0.002,0.08]  SetSaturation=off  Rm=500  Lm=500  Saturation=[ 0,0 ; 0.0024,1.2 ; 1.0,1.52 ]  Hysteresis=off  DataFile='hysteresis'  SetInitialFlux=off  InitialFluxes=[ 0.8 , -0.8 , 0.7 ]  Measurements=None  MoreParameters=off  BreakLoop=off  DataType=off  TransfoNumber=1
  T_280269221__ : powerlib/Elements/Three-Phase Transformer (Two Windings)  Winding1Connection=Yg  UNITS=pu  NominalPower=[ 250e6 , 60 ]  Winding1=[110000,0.002,0.08]  Winding2Connection=Yg  Winding2=[110000,0.002,0.08]  SetSaturation=off  Rm=500  Lm=500  Saturation=[ 0,0 ; 0.0024,1.2 ; 1.0,1.52 ]  Hysteresis=off  DataFile='hysteresis'  SetInitialFlux=off  InitialFluxes=[ 0.8 , -0.8 , 0.7 ]  Measurements=None  MoreParameters=off  BreakLoop=off  DataType=off  TransfoNumber=1
  T_29428018_330000_ПС_330_кВ_Гродно : powerlib/Elements/Three-Phase Transformer (Two Windings)  Winding1Connection=Yg  UNITS=pu  NominalPower=[ 250e6 , 60 ]  Winding1=[330000,0.002,0.08]  Winding2Connection=Yg  Winding2=[330000,0.002,0.08]  SetSaturation=off  Rm=500  Lm=500  Saturation=[ 0,0 ; 0.0024,1.2 ; 1.0,1.52 ]  Hysteresis=off  DataFile='hysteresis'  SetInitialFlux=off  InitialFluxes=[ 0.8 , -0.8 , 0.7 ]  Measurements=None  MoreParameters=off  BreakLoop=off  DataType=off  TransfoNumber=1
  T_296374470__ : powerlib/Elements/Three-Phase Transformer (Two Windings)  Winding1Connection=Yg  UNITS=pu  NominalPower=[ 250e6 , 60 ]  Winding1=[110000,0.002,0.08]  Winding2Connection=Yg  Winding2=[110000,0.002,0.08]  SetSaturation=off  Rm=500  Lm=500  Saturation=[ 0,0 ; 0.0024,1.2 ; 1.0,1.52 ]  Hysteresis=off  DataFile='hysteresis'  SetInitialFlux=off  InitialFluxes=[ 0.8 , -0.8 , 0.7 ]  Measurements=None  MoreParameters=off  BreakLoop=off  DataType=off  TransfoNumber=1
  T_75909941__Bubių_pastotė : powerlib/Elements/Three-Phase Transformer (Two Windings)  Winding1Connection=Yg  UNITS=pu  NominalPower=[ 250e6 , 60 ]  Winding1=[110000,0.002,0.08]  Winding2Connection=Yg  Winding2=[110000,0.002,0.08]  SetSaturation=off  Rm=500  Lm=500  Saturation=[ 0,0 ; 0.0024,1.2 ; 1.0,1.52 ]  Hysteresis=off  DataFile='hysteresis'  SetInitialFlux=off  InitialFluxes=[ 0.8 , -0.8 , 0.7 ]  Measurements=None  MoreParameters=off  BreakLoop=off  DataType=off  TransfoNumber=1
  T_88726161__Eigulių_TP : powerlib/Elements/Three-Phase Transformer (Two Windings)  Winding1Connection=Yg  UNITS=pu  NominalPower=[ 250e6 , 60 ]  Winding1=[110000,0.002,0.08]  Winding2Connection=Yg  Winding2=[110000,0.002,0.08]  SetSaturation=off  Rm=500  Lm=500  Saturation=[ 0,0 ; 0.0024,1.2 ; 1.0,1.52 ]  Hysteresis=off  DataFile='hysteresis'  SetInitialFlux=off  InitialFluxes=[ 0.8 , -0.8 , 0.7 ]  Measurements=None  MoreParameters=off  BreakLoop=off  DataType=off  TransfoNumber=1
  T_95066966__Rėkyvos_pastotė : powerlib/Elements/Three-Phase Transformer (Two Windings)  Winding1Connection=Yg  UNITS=pu  NominalPower=[ 250e6 , 60 ]  Winding1=[110000,0.002,0.08]  Winding2Connection=Yg  Winding2=[110000,0.002,0.08]  SetSaturation=off  Rm=500  Lm=500  Saturation=[ 0,0 ; 0.0024,1.2 ; 1.0,1.52 ]  Hysteresis=off  DataFile='hysteresis'  SetInitialFlux=off  InitialFluxes=[ 0.8 , -0.8 , 0.7 ]  Measurements=None  MoreParameters=off  BreakLoop=off  DataType=off  TransfoNumber=1
  T_95066982__ : powerlib/Elements/Three-Phase Transformer (Two Windings)  Winding1Connection=Yg  UNITS=pu  NominalPower=[ 250e6 , 60 ]  Winding1=[110000,0.002,0.08]  Winding2Connection=Yg  Winding2=[110000,0.002,0.08]  SetSaturation=off  Rm=500  Lm=500  Saturation=[ 0,0 ; 0.0024,1.2 ; 1.0,1.52 ]  Hysteresis=off  DataFile='hysteresis'  SetInitialFlux=off  InitialFluxes=[ 0.8 , -0.8 , 0.7 ]  Measurements=None  MoreParameters=off  BreakLoop=off  DataType=off  TransfoNumber=1
  T_95866738__ : powerlib/Elements/Three-Phase Transformer (Two Windings)  Winding1Connection=Yg  UNITS=pu  NominalPower=[ 250e6 , 60 ]  Winding1=[110000,0.002,0.08]  Winding2Connection=Yg  Winding2=[110000,0.002,0.08]  SetSaturation=off  Rm=500  Lm=500  Saturation=[ 0,0 ; 0.0024,1.2 ; 1.0,1.52 ]  Hysteresis=off  DataFile='hysteresis'  SetInitialFlux=off  InitialFluxes=[ 0.8 , -0.8 , 0.7 ]  Measurements=None  MoreParameters=off  BreakLoop=off  DataType=off  TransfoNumber=1
  T_99049777__Gubernijos_pastotė : powerlib/Elements/Three-Phase Transformer (Two Windings)  Winding1Connection=Yg  UNITS=pu  NominalPower=[ 250e6 , 60 ]  Winding1=[110000,0.002,0.08]  Winding2Connection=Yg  Winding2=[110000,0.002,0.08]  SetSaturation=off  Rm=500  Lm=500  Saturation=[ 0,0 ; 0.0024,1.2 ; 1.0,1.52 ]  Hysteresis=off  DataFile='hysteresis'  SetInitialFlux=off  InitialFluxes=[ 0.8 , -0.8 , 0.7 ]  Measurements=None  MoreParameters=off  BreakLoop=off  DataType=off  TransfoNumber=1
  T_99049787__Zoknių_pastotė : powerlib/Elements/Three-Phase Transformer (Two Windings)  Winding1Connection=Yg  UNITS=pu  NominalPower=[ 250e6 , 60 ]  Winding1=[110000,0.002,0.08]  Winding2Connection=Yg  Winding2=[110000,0.002,0.08]  SetSaturation=off  Rm=500  Lm=500  Saturation=[ 0,0 ; 0.0024,1.2 ; 1.0,1.52 ]  Hysteresis=off  DataFile='hysteresis'  SetInitialFlux=off  InitialFluxes=[ 0.8 , -0.8 , 0.7 ]  Measurements=None  MoreParameters=off  BreakLoop=off  DataType=off  TransfoNumber=1
  T_99049810_110000;35000;fixme_ : powerlib/Elements/Three-Phase Transformer (Two Windings)  Winding1Connection=Yg  UNITS=pu  NominalPower=[ 250e6 , 60 ]  Winding1=[110000,0.002,0.08]  Winding2Connection=Yg  Winding2=[110000,0.002,0.08]  SetSaturation=off  Rm=500  Lm=500  Saturation=[ 0,0 ; 0.0024,1.2 ; 1.0,1.52 ]  Hysteresis=off  DataFile='hysteresis'  SetInitialFlux=off  InitialFluxes=[ 0.8 , -0.8 , 0.7 ]  Measurements=None  MoreParameters=off  BreakLoop=off  DataType=off  TransfoNumber=1
  _CN_103275527_110000_CN_103275551_110000 : powerlib/Elements/Distributed Parameters Line  Phases=3  Frequency=60  Resistance=[0.01273 0.3864]  Inductance="[0.9337e-3  4.1264e-3]"  Capacitance=[12.74e-9 7.751e-9]  Length=11.5173  x1=[0 0 0 0; 0.0001244 0 0 0; 0.0002488 0 0 0; 0.0003733 0 0 0; 0.0004977 0 0 0; 0.0006221 0 0 0]  x2=[0 0 0 0; 0.0001244 0 0 0; 0.0002488 0 0 0; 0.0003733 0 0 0; 0.0004977 0 0 0; 0.0006221 0 0 0]  x3=[0 0 0 0; 0.0001244 0 0 0; 0.0002488 0 0 0; 0.0003733 0 0 0; 0.0004977 0 0 0; 0.0006221 0 0 0]  x4=[0 0 0 0; 0.0001244 0 0 0; 0.0002488 0 0 0; 0.0003733 0 0 0; 0.0004977 0 0 0; 0.0006221 0 0 0]  x5=0  V1=ones(3,3)  V2=ones(3,3)  I1=ones(3,3)  I2=ones(3,3)  nHarmo=1  Measurements=None
  _CN_103275527_110000_CN_103275559_110000 : powerlib/Elements/Distributed Parameters Line  Phases=3  Frequency=60  Resistance=[0.01273 0.3864]  Inductance="[0.9337e-3  4.1264e-3]"  Capacitance=[12.74e-9 7.751e-9]  Length=6.9865  x1=[0 0 0 0; 0.0001244 0 0 0; 0.0002488 0 0 0; 0.0003733 0 0 0; 0.0004977 0 0 0; 0.0006221 0 0 0]  x2=[0 0 0 0; 0.0001244 0 0 0; 0.0002488 0 0 0; 0.0003733 0 0 0; 0.0004977 0 0 0; 0.0006221 0 0 0]  x3=[0 0 0 0; 0.0001244 0 0 0; 0.0002488 0 0 0; 0.0003733 0 0 0; 0.0004977 0 0 0; 0.0006221 0 0 0]  x4=[0 0 0 0; 0.0001244 0 0 0; 0.0002488 0 0 0; 0.0003733 0 0 0; 0.0004977 0 0 0; 0.0006221 0 0 0]  x5=0  V1=ones(3,3)  V2=ones(3,3)  I1=ones(3,3)  I2=ones(3,3)  nHarmo=1  Measurements=None
  _CN_103275527_110000_CN_103560163_110000 : powerlib/Elements/Distributed Parameters Line  Phases=3  Frequency=60  Resistance=[0.01273 0.3864]  Inductance="[0.9337e-3  4.1264e-3]"  Capacitance=[12.74e-9 7.751e-9]  Length=39.7331  x1=[0 0 0 0; 0.0001244 0 0 0; 0.0002488 0 0 0; 0.0003733 0 0 0; 0.0004977 0 0 0; 0.0006221 0 0 0]  x2=[0 0 0 0; 0.0001244 0 0 0; 0.0002488 0 0 0; 0.0003733 0 0 0; 0.0004977 0 0 0; 0.0006221 0 0 0]  x3=[0 0 0 0; 0.0001244 0 0 0; 0.0002488 0 0 0; 0.0003733 0 0 0; 0.0004977 0 0 0; 0.0006221 0 0 0]  x4=[0 0 0 0; 0.0001244 0 0 0; 0.0002488 0 0 0; 0.0003733 0 0 0; 0.0004977 0 0 0; 0.0006221 0 0 0]  x5=0  V1=ones(3,3)  V2=ones(3,3)  I1=ones(3,3)  I2=ones(3,3)  nHarmo=1  Measurements=None
  _CN_103275527_110000_CN_124462106_110000 : powerlib/Elements/Distributed Parameters Line  Phases=3  Frequency=60  Resistance=[0.01273 0.3864]  Inductance="[0.9337e-3  4.1264e-3]"  Capacitance=[12.74e-9 7.751e-9]  Length=39.1201  x1=[0 0 0 0; 0.0001244 0 0 0; 0.0002488 0 0 0; 0.0003733 0 0 0; 0.0004977 0 0 0; 0.0006221 0 0 0]  x2=[0 0 0 0; 0.0001244 0 0 0; 0.0002488 0 0 0; 0.0003733 0 0 0; 0.0004977 0 0 0; 0.0006221 0 0 0]  x3=[0 0 0 0; 0.0001244 0 0 0; 0.0002488 0 0 0; 0.0003733 0 0 0; 0.0004977 0 0 0; 0.0006221 0 0 0]  x4=[0 0 0 0; 0.0001244 0 0 0; 0.0002488 0 0 0; 0.0003733 0 0 0; 0.0004977 0 0 0; 0.0006221 0 0 0]  x5=0  V1=ones(3,3)  V2=ones(3,3)  I1=ones(3,3)  I2=ones(3,3)  nHarmo=1  Measurements=None
  _CN_103275527_110000_CN_171630121_110000 : powerlib/Elements/Distributed Parameters Line  Phases=3  Frequency=60  Resistance=[0.01273 0.3864]  Inductance="[0.9337e-3  4.1264e-3]"  Capacitance=[12.74e-9 7.751e-9]  Length=30.979  x1=[0 0 0 0; 0.0001244 0 0 0; 0.0002488 0 0 0; 0.0003733 0 0 0; 0.0004977 0 0 0; 0.0006221 0 0 0]  x2=[0 0 0 0; 0.0001244 0 0 0; 0.0002488 0 0 0; 0.0003733 0 0 0; 0.0004977 0 0 0; 0.0006221 0 0 0]  x3=[0 0 0 0; 0.0001244 0 0 0; 0.0002488 0 0 0; 0.0003733 0 0 0; 0.0004977 0 0 0; 0.0006221 0 0 0]  x4=[0 0 0 0; 0.0001244 0 0 0; 0.0002488 0 0 0; 0.0003733 0 0 0; 0.0004977 0 0 0; 0.0006221 0 0 0]  x5=0  V1=ones(3,3)  V2=ones(3,3)  I1=ones(3,3)  I2=ones(3,3)  nHarmo=1  Measurements=None
  _CN_103275527_110000_CN_209204254_110000 : powerlib/Elements/Distributed Parameters Line  Phases=3  Frequency=60  Resistance=[0.01273 0.3864]  Inductance="[0.9337e-3  4.1264e-3]"  Capacitance=[12.74e-9 7.751e-9]  Length=22.4417  x1=[0 0 0 0; 0.0001244 0 0 0; 0.0002488 0 0 0; 0.0003733 0 0 0; 0.0004977 0 0 0; 0.0006221 0 0 0]  x2=[0 0 0 0; 0.0001244 0 0 0; 0.0002488 0 0 0; 0.0003733 0 0 0; 0.0004977 0 0 0; 0.0006221 0 0 0]  x3=[0 0 0 0; 0.0001244 0 0 0; 0.0002488 0 0 0; 0.0003733 0 0 0; 0.0004977 0 0 0; 0.0006221 0 0 0]  x4=[0 0 0 0; 0.0001244 0 0 0; 0.0002488 0 0 0; 0.0003733 0 0 0; 0.0004977 0 0 0; 0.0006221 0 0 0]  x5=0  V1=ones(3,3)  V2=ones(3,3)  I1=ones(3,3)  I2=ones(3,3)  nHarmo=1  Measurements=None
  _CN_103275559_110000_CN_103275575_110000 : powerlib/Elements/Distributed Parameters Line  Phases=3  Frequency=60  Resistance=[0.01273 0.3864]  Inductance="[0.9337e-3  4.1264e-3]"  Capacitance=[12.74e-9 7.751e-9]  Length=11.2669  x1=[0 0 0 0; 0.0001244 0 0 0; 0.0002488 0 0 0; 0.0003733 0 0 0; 0.0004977 0 0 0; 0.0006221 0 0 0]  x2=[0 0 0 0; 0.0001244 0 0 0; 0.0002488 0 0 0; 0.0003733 0 0 0; 0.0004977 0 0 0; 0.0006221 0 0 0]  x3=[0 0 0 0; 0.0001244 0 0 0; 0.0002488 0 0 0; 0.0003733 0 0 0; 0.0004977 0 0 0; 0.0006221 0 0 0]  x4=[0 0 0 0; 0.0001244 0 0 0; 0.0002488 0 0 0; 0.0003733 0 0 0; 0.0004977 0 0 0; 0.0006221 0 0 0]  x5=0  V1=ones(3,3)  V2=ones(3,3)  I1=ones(3,3)  I2=ones(3,3)  nHarmo=1  Measurements=None
  _CN_103275575_110000_CN_104774544_110000 : powerlib/Elements/Distributed Parameters Line  Phases=3  Frequency=60  Resistance=[0.01273 0.3864]  Inductance="[0.9337e-3  4.1264e-3]"  Capacitance=[12.74e-9 7.751e-9]  Length=12.668  x1=[0 0 0 0; 0.0001244 0 0 0; 0.0002488 0 0 0; 0.0003733 0 0 0; 0.0004977 0 0 0; 0.0006221 0 0 0]  x2=[0 0 0 0; 0.0001244 0 0 0; 0.0002488 0 0 0; 0.0003733 0 0 0; 0.0004977 0 0 0; 0.0006221 0 0 0]  x3=[0 0 0 0; 0.0001244 0 0 0; 0.0002488 0 0 0; 0.0003733 0 0 0; 0.0004977 0 0 0; 0.0006221 0 0 0]  x4=[0 0 0 0; 0.0001244 0 0 0; 0.0002488 0 0 0; 0.0003733 0 0 0; 0.0004977 0 0 0; 0.0006221 0 0 0]  x5=0  V1=ones(3,3)  V2=ones(3,3)  I1=ones(3,3)  I2=ones(3,3)  nHarmo=1  Measurements=None
  _CN_103554499_110000_CN_217391080_110000 : powerlib/Elements/Distributed Parameters Line  Phases=3  Frequency=60  Resistance=[0.01273 0.3864]  Inductance="[0.9337e-3  4.1264e-3]"  Capacitance=[12.74e-9 7.751e-9]  Length=23.6117  x1=[0 0 0 0; 0.0001244 0 0 0; 0.0002488 0 0 0; 0.0003733 0 0 0; 0.0004977 0 0 0; 0.0006221 0 0 0]  x2=[0 0 0 0; 0.0001244 0 0 0; 0.0002488 0 0 0; 0.0003733 0 0 0; 0.0004977 0 0 0; 0.0006221 0 0 0]  x3=[0 0 0 0; 0.0001244 0 0 0; 0.0002488 0 0 0; 0.0003733 0 0 0; 0.0004977 0 0 0; 0.0006221 0 0 0]  x4=[0 0 0 0; 0.0001244 0 0 0; 0.0002488 0 0 0; 0.0003733 0 0 0; 0.0004977 0 0 0; 0.0006221 0 0 0]  x5=0  V1=ones(3,3)  V2=ones(3,3)  I1=ones(3,3)  I2=ones(3,3)  nHarmo=1  Measurements=None
  _CN_104774536_110000_CN_104774544_110000 : powerlib/Elements/Distributed Parameters Line  Phases=3  Frequency=60  Resistance=[0.01273 0.3864]  Inductance="[0.9337e-3  4.1264e-3]"  Capacitance=[12.74e-9 7.751e-9]  Length=14.8578  x1=[0 0 0 0; 0.0001244 0 0 0; 0.0002488 0 0 0; 0.0003733 0 0 0; 0.0004977 0 0 0; 0.0006221 0 0 0]  x2=[0 0 0 0; 0.0001244 0 0 0; 0.0002488 0 0 0; 0.0003733 0 0 0; 0.0004977 0 0 0; 0.0006221 0 0 0]  x3=[0 0 0 0; 0.0001244 0 0 0; 0.0002488 0 0 0; 0.0003733 0 0 0; 0.0004977 0 0 0; 0.0006221 0 0 0]  x4=[0 0 0 0; 0.0001244 0 0 0; 0.0002488 0 0 0; 0.0003733 0 0 0; 0.0004977 0 0 0; 0.0006221 0 0 0]  x5=0  V1=ones(3,3)  V2=ones(3,3)  I1=ones(3,3)  I2=ones(3,3)  nHarmo=1  Measurements=None
  _CN_105587267_110000_CN_243085462_110000 : powerlib/Elements/Distributed Parameters Line  Phases=3  Frequency=60  Resistance=[0.01273 0.3864]  Inductance="[0.9337e-3  4.1264e-3]"  Capacitance=[12.74e-9 7.751e-9]  Length=9.7055  x1=[0 0 0 0; 0.0001244 0 0 0; 0.0002488 0 0 0; 0.0003733 0 0 0; 0.0004977 0 0 0; 0.0006221 0 0 0]  x2=[0 0 0 0; 0.0001244 0 0 0; 0.0002488 0 0 0; 0.0003733 0 0 0; 0.0004977 0 0 0; 0.0006221 0 0 0]  x3=[0 0 0 0; 0.0001244 0 0 0; 0.0002488 0 0 0; 0.0003733 0 0 0; 0.0004977 0 0 0; 0.0006221 0 0 0]  x4=[0 0 0 0; 0.0001244 0 0 0; 0.0002488 0 0 0; 0.0003733 0 0 0; 0.0004977 0 0 0; 0.0006221 0 0 0]  x5=0  V1=ones(3,3)  V2=ones(3,3)  I1=ones(3,3)  I2=ones(3,3)  nHarmo=1  Measurements=None
  _CN_127212679_110000_CN_130577811_110000 : powerlib/Elements/Distributed Parameters Line  Phases=3  Frequency=60  Resistance=[0.01273 0.3864]  Inductance="[0.9337e-3  4.1264e-3]"  Capacitance=[12.74e-9 7.751e-9]  Length=4.4418  x1=[0 0 0 0; 0.0001244 0 0 0; 0.0002488 0 0 0; 0.0003733 0 0 0; 0.0004977 0 0 0; 0.0006221 0 0 0]  x2=[0 0 0 0; 0.0001244 0 0 0; 0.0002488 0 0 0; 0.0003733 0 0 0; 0.0004977 0 0 0; 0.0006221 0 0 0]  x3=[0 0 0 0; 0.0001244 0 0 0; 0.0002488 0 0 0; 0.0003733 0 0 0; 0.0004977 0 0 0; 0.0006221 0 0 0]  x4=[0 0 0 0; 0.0001244 0 0 0; 0.0002488 0 0 0; 0.0003733 0 0 0; 0.0004977 0 0 0; 0.0006221 0 0 0]  x5=0  V1=ones(3,3)  V2=ones(3,3)  I1=ones(3,3)  I2=ones(3,3)  nHarmo=1  Measurements=None
  _CN_127212679_110000_CN_172019115_110000 : powerlib/Elements/Distributed Parameters Line  Phases=3  Frequency=60  Resistance=[0.01273 0.3864]  Inductance="[0.9337e-3  4.1264e-3]"  Capacitance=[12.74e-9 7.751e-9]  Length=12.5087  x1=[0 0 0 0; 0.0001244 0 0 0; 0.0002488 0 0 0; 0.0003733 0 0 0; 0.0004977 0 0 0; 0.0006221 0 0 0]  x2=[0 0 0 0; 0.0001244 0 0 0; 0.0002488 0 0 0; 0.0003733 0 0 0; 0.0004977 0 0 0; 0.0006221 0 0 0]  x3=[0 0 0 0; 0.0001244 0 0 0; 0.0002488 0 0 0; 0.0003733 0 0 0; 0.0004977 0 0 0; 0.0006221 0 0 0]  x4=[0 0 0 0; 0.0001244 0 0 0; 0.0002488 0 0 0; 0.0003733 0 0 0; 0.0004977 0 0 0; 0.0006221 0 0 0]  x5=0  V1=ones(3,3)  V2=ones(3,3)  I1=ones(3,3)  I2=ones(3,3)  nHarmo=1  Measurements=None
  _CN_135644003_110000_CN_25698690_110000 : powerlib/Elements/Distributed Parameters Line  Phases=3  Frequency=60  Resistance=[0.01273 0.3864]  Inductance="[0.9337e-3  4.1264e-3]"  Capacitance=[12.74e-9 7.751e-9]  Length=32.3079  x1=[0 0 0 0; 0.0001244 0 0 0; 0.0002488 0 0 0; 0.0003733 0 0 0; 0.0004977 0 0 0; 0.0006221 0 0 0]  x2=[0 0 0 0; 0.0001244 0 0 0; 0.0002488 0 0 0; 0.0003733 0 0 0; 0.0004977 0 0 0; 0.0006221 0 0 0]  x3=[0 0 0 0; 0.0001244 0 0 0; 0.0002488 0 0 0; 0.0003733 0 0 0; 0.0004977 0 0 0; 0.0006221 0 0 0]  x4=[0 0 0 0; 0.0001244 0 0 0; 0.0002488 0 0 0; 0.0003733 0 0 0; 0.0004977 0 0 0; 0.0006221 0 0 0]  x5=0  V1=ones(3,3)  V2=ones(3,3)  I1=ones(3,3)  I2=ones(3,3)  nHarmo=1  Measurements=None
  _CN_135644003_110000_CN_257684864_110000 : powerlib/Elements/Distributed Parameters Line  Phases=3  Frequency=60  Resistance=[0.01273 0.3864]  Inductance="[0.9337e-3  4.1264e-3]"  Capacitance=[12.74e-9 7.751e-9]  Length=15.3655  x1=[0 0 0 0; 0.0001244 0 0 0; 0.0002488 0 0 0; 0.0003733 0 0 0; 0.0004977 0 0 0; 0.0006221 0 0 0]  x2=[0 0 0 0; 0.0001244 0 0 0; 0.0002488 0 0 0; 0.0003733 0 0 0; 0.0004977 0 0 0; 0.0006221 0 0 0]  x3=[0 0 0 0; 0.0001244 0 0 0; 0.0002488 0 0 0; 0.0003733 0 0 0; 0.0004977 0 0 0; 0.0006221 0 0 0]  x4=[0 0 0 0; 0.0001244 0 0 0; 0.0002488 0 0 0; 0.0003733 0 0 0; 0.0004977 0 0 0; 0.0006221 0 0 0]  x5=0  V1=ones(3,3)  V2=ones(3,3)  I1=ones(3,3)  I2=ones(3,3)  nHarmo=1  Measurements=None
  _CN_135644003_110000_CN_257684865_110000 : powerlib/Elements/Distributed Parameters Line  Phases=3  Frequency=60  Resistance=[0.01273 0.3864]  Inductance="[0.9337e-3  4.1264e-3]"  Capacitance=[12.74e-9 7.751e-9]  Length=6.0451  x1=[0 0 0 0; 0.0001244 0 0 0; 0.0002488 0 0 0; 0.0003733 0 0 0; 0.0004977 0 0 0; 0.0006221 0 0 0]  x2=[0 0 0 0; 0.0001244 0 0 0; 0.0002488 0 0 0; 0.0003733 0 0 0; 0.0004977 0 0 0; 0.0006221 0 0 0]  x3=[0 0 0 0; 0.0001244 0 0 0; 0.0002488 0 0 0; 0.0003733 0 0 0; 0.0004977 0 0 0; 0.0006221 0 0 0]  x4=[0 0 0 0; 0.0001244 0 0 0; 0.0002488 0 0 0; 0.0003733 0 0 0; 0.0004977 0 0 0; 0.0006221 0 0 0]  x5=0  V1=ones(3,3)  V2=ones(3,3)  I1=ones(3,3)  I2=ones(3,3)  nHarmo=1  Measurements=None
  _CN_142782984_110000_CN_153249112_110000 : powerlib/Elements/Distributed Parameters Line  Phases=3  Frequency=60  Resistance=[0.01273 0.3864]  Inductance="[0.9337e-3  4.1264e-3]"  Capacitance=[12.74e-9 7.751e-9]  Length=19.1818  x1=[0 0 0 0; 0.0001244 0 0 0; 0.0002488 0 0 0; 0.0003733 0 0 0; 0.0004977 0 0 0; 0.0006221 0 0 0]  x2=[0 0 0 0; 0.0001244 0 0 0; 0.0002488 0 0 0; 0.0003733 0 0 0; 0.0004977 0 0 0; 0.0006221 0 0 0]  x3=[0 0 0 0; 0.0001244 0 0 0; 0.0002488 0 0 0; 0.0003733 0 0 0; 0.0004977 0 0 0; 0.0006221 0 0 0]  x4=[0 0 0 0; 0.0001244 0 0 0; 0.0002488 0 0 0; 0.0003733 0 0 0; 0.0004977 0 0 0; 0.0006221 0 0 0]  x5=0  V1=ones(3,3)  V2=ones(3,3)  I1=ones(3,3)  I2=ones(3,3)  nHarmo=1  Measurements=None
  _CN_142782984_110000_CN_173582225_110000 : powerlib/Elements/Distributed Parameters Line  Phases=3  Frequency=60  Resistance=[0.01273 0.3864]  Inductance="[0.9337e-3  4.1264e-3]"  Capacitance=[12.74e-9 7.751e-9]  Length=35.0394  x1=[0 0 0 0; 0.0001244 0 0 0; 0.0002488 0 0 0; 0.0003733 0 0 0; 0.0004977 0 0 0; 0.0006221 0 0 0]  x2=[0 0 0 0; 0.0001244 0 0 0; 0.0002488 0 0 0; 0.0003733 0 0 0; 0.0004977 0 0 0; 0.0006221 0 0 0]  x3=[0 0 0 0; 0.0001244 0 0 0; 0.0002488 0 0 0; 0.0003733 0 0 0; 0.0004977 0 0 0; 0.0006221 0 0 0]  x4=[0 0 0 0; 0.0001244 0 0 0; 0.0002488 0 0 0; 0.0003733 0 0 0; 0.0004977 0 0 0; 0.0006221 0 0 0]  x5=0  V1=ones(3,3)  V2=ones(3,3)  I1=ones(3,3)  I2=ones(3,3)  nHarmo=1  Measurements=None
  _CN_142782984_110000_CN_25698690_110000 : powerlib/Elements/Distributed Parameters Line  Phases=3  Frequency=60  Resistance=[0.01273 0.3864]  Inductance="[0.9337e-3  4.1264e-3]"  Capacitance=[12.74e-9 7.751e-9]  Length=17.2748  x1=[0 0 0 0; 0.0001244 0 0 0; 0.0002488 0 0 0; 0.0003733 0 0 0; 0.0004977 0 0 0; 0.0006221 0 0 0]  x2=[0 0 0 0; 0.0001244 0 0 0; 0.0002488 0 0 0; 0.0003733 0 0 0; 0.0004977 0 0 0; 0.0006221 0 0 0]  x3=[0 0 0 0; 0.0001244 0 0 0; 0.0002488 0 0 0; 0.0003733 0 0 0; 0.0004977 0 0 0; 0.0006221 0 0 0]  x4=[0 0 0 0; 0.0001244 0 0 0; 0.0002488 0 0 0; 0.0003733 0 0 0; 0.0004977 0 0 0; 0.0006221 0 0 0]  x5=0  V1=ones(3,3)  V2=ones(3,3)  I1=ones(3,3)  I2=ones(3,3)  nHarmo=1  Measurements=None
  _CN_150992936_110000_CN_151783148_110000 : powerlib/Elements/Distributed Parameters Line  Phases=3  Frequency=60  Resistance=[0.01273 0.3864]  Inductance="[0.9337e-3  4.1264e-3]"  Capacitance=[12.74e-9 7.751e-9]  Length=15.3391  x1=[0 0 0 0; 0.0001244 0 0 0; 0.0002488 0 0 0; 0.0003733 0 0 0; 0.0004977 0 0 0; 0.0006221 0 0 0]  x2=[0 0 0 0; 0.0001244 0 0 0; 0.0002488 0 0 0; 0.0003733 0 0 0; 0.0004977 0 0 0; 0.0006221 0 0 0]  x3=[0 0 0 0; 0.0001244 0 0 0; 0.0002488 0 0 0; 0.0003733 0 0 0; 0.0004977 0 0 0; 0.0006221 0 0 0]  x4=[0 0 0 0; 0.0001244 0 0 0; 0.0002488 0 0 0; 0.0003733 0 0 0; 0.0004977 0 0 0; 0.0006221 0 0 0]  x5=0  V1=ones(3,3)  V2=ones(3,3)  I1=ones(3,3)  I2=ones(3,3)  nHarmo=1  Measurements=None
  _CN_150992936_110000_CN_218216075_110000 : powerlib/Elements/Distributed Parameters Line  Phases=3  Frequency=60  Resistance=[0.01273 0.3864]  Inductance="[0.9337e-3  4.1264e-3]"  Capacitance=[12.74e-9 7.751e-9]  Length=28.868  x1=[0 0 0 0; 0.0001244 0 0 0; 0.0002488 0 0 0; 0.0003733 0 0 0; 0.0004977 0 0 0; 0.0006221 0 0 0]  x2=[0 0 0 0; 0.0001244 0 0 0; 0.0002488 0 0 0; 0.0003733 0 0 0; 0.0004977 0 0 0; 0.0006221 0 0 0]  x3=[0 0 0 0; 0.0001244 0 0 0; 0.0002488 0 0 0; 0.0003733 0 0 0; 0.0004977 0 0 0; 0.0006221 0 0 0]  x4=[0 0 0 0; 0.0001244 0 0 0; 0.0002488 0 0 0; 0.0003733 0 0 0; 0.0004977 0 0 0; 0.0006221 0 0 0]  x5=0  V1=ones(3,3)  V2=ones(3,3)  I1=ones(3,3)  I2=ones(3,3)  nHarmo=1  Measurements=None
  _CN_151237667_110000_CN_134987741_110000 : powerlib/Elements/Distributed Parameters Line  Phases=3  Frequency=60  Resistance=[0.01273 0.3864]  Inductance="[0.9337e-3  4.1264e-3]"  Capacitance=[12.74e-9 7.751e-9]  Length=13.2437  x1=[0 0 0 0; 0.0001244 0 0 0; 0.0002488 0 0 0; 0.0003733 0 0 0; 0.0004977 0 0 0; 0.0006221 0 0 0]  x2=[0 0 0 0; 0.0001244 0 0 0; 0.0002488 0 0 0; 0.0003733 0 0 0; 0.0004977 0 0 0; 0.0006221 0 0 0]  x3=[0 0 0 0; 0.0001244 0 0 0; 0.0002488 0 0 0; 0.0003733 0 0 0; 0.0004977 0 0 0; 0.0006221 0 0 0]  x4=[0 0 0 0; 0.0001244 0 0 0; 0.0002488 0 0 0; 0.0003733 0 0 0; 0.0004977 0 0 0; 0.0006221 0 0 0]  x5=0  V1=ones(3,3)  V2=ones(3,3)  I1=ones(3,3)  I2=ones(3,3)  nHarmo=1  Measurements=None
  _CN_153249112_110000_CN_25698690_110000 : powerlib/Elements/Distributed Parameters Line  Phases=3  Frequency=60  Resistance=[0.01273 0.3864]  Inductance="[0.9337e-3  4.1264e-3]"  Capacitance=[12.74e-9 7.751e-9]  Length=3.9761  x1=[0 0 0 0; 0.0001244 0 0 0; 0.0002488 0 0 0; 0.0003733 0 0 0; 0.0004977 0 0 0; 0.0006221 0 0 0]  x2=[0 0 0 0; 0.0001244 0 0 0; 0.0002488 0 0 0; 0.0003733 0 0 0; 0.0004977 0 0 0; 0.0006221 0 0 0]  x3=[0 0 0 0; 0.0001244 0 0 0; 0.0002488 0 0 0; 0.0003733 0 0 0; 0.0004977 0 0 0; 0.0006221 0 0 0]  x4=[0 0 0 0; 0.0001244 0 0 0; 0.0002488 0 0 0; 0.0003733 0 0 0; 0.0004977 0 0 0; 0.0006221 0 0 0]  x5=0  V1=ones(3,3)  V2=ones(3,3)  I1=ones(3,3)  I2=ones(3,3)  nHarmo=1  Measurements=None
  _CN_158505202_110000_CN_106172865_110000 : powerlib/Elements/Distributed Parameters Line  Phases=3  Frequency=60  Resistance=[0.01273 0.3864]  Inductance="[0.9337e-3  4.1264e-3]"  Capacitance=[12.74e-9 7.751e-9]  Length=13.5924  x1=[0 0 0 0; 0.0001244 0 0 0; 0.0002488 0 0 0; 0.0003733 0 0 0; 0.0004977 0 0 0; 0.0006221 0 0 0]  x2=[0 0 0 0; 0.0001244 0 0 0; 0.0002488 0 0 0; 0.0003733 0 0 0; 0.0004977 0 0 0; 0.0006221 0 0 0]  x3=[0 0 0 0; 0.0001244 0 0 0; 0.0002488 0 0 0; 0.0003733 0 0 0; 0.0004977 0 0 0; 0.0006221 0 0 0]  x4=[0 0 0 0; 0.0001244 0 0 0; 0.0002488 0 0 0; 0.0003733 0 0 0; 0.0004977 0 0 0; 0.0006221 0 0 0]  x5=0  V1=ones(3,3)  V2=ones(3,3)  I1=ones(3,3)  I2=ones(3,3)  nHarmo=1  Measurements=None
  _CN_158505202_110000_CN_172394893_110000 : powerlib/Elements/Distributed Parameters Line  Phases=3  Frequency=60  Resistance=[0.01273 0.3864]  Inductance="[0.9337e-3  4.1264e-3]"  Capacitance=[12.74e-9 7.751e-9]  Length=27.0336  x1=[0 0 0 0; 0.0001244 0 0 0; 0.0002488 0 0 0; 0.0003733 0 0 0; 0.0004977 0 0 0; 0.0006221 0 0 0]  x2=[0 0 0 0; 0.0001244 0 0 0; 0.0002488 0 0 0; 0.0003733 0 0 0; 0.0004977 0 0 0; 0.0006221 0 0 0]  x3=[0 0 0 0; 0.0001244 0 0 0; 0.0002488 0 0 0; 0.0003733 0 0 0; 0.0004977 0 0 0; 0.0006221 0 0 0]  x4=[0 0 0 0; 0.0001244 0 0 0; 0.0002488 0 0 0; 0.0003733 0 0 0; 0.0004977 0 0 0; 0.0006221 0 0 0]  x5=0  V1=ones(3,3)  V2=ones(3,3)  I1=ones(3,3)  I2=ones(3,3)  nHarmo=1  Measurements=None
  _CN_158505202_110000_CN_176323123_110000 : powerlib/Elements/Distributed Parameters Line  Phases=3  Frequency=60  Resistance=[0.01273 0.3864]  Inductance="[0.9337e-3  4.1264e-3]"  Capacitance=[12.74e-9 7.751e-9]  Length=7.1726  x1=[0 0 0 0; 0.0001244 0 0 0; 0.0002488 0 0 0; 0.0003733 0 0 0; 0.0004977 0 0 0; 0.0006221 0 0 0]  x2=[0 0 0 0; 0.0001244 0 0 0; 0.0002488 0 0 0; 0.0003733 0 0 0; 0.0004977 0 0 0; 0.0006221 0 0 0]  x3=[0 0 0 0; 0.0001244 0 0 0; 0.0002488 0 0 0; 0.0003733 0 0 0; 0.0004977 0 0 0; 0.0006221 0 0 0]  x4=[0 0 0 0; 0.0001244 0 0 0; 0.0002488 0 0 0; 0.0003733 0 0 0; 0.0004977 0 0 0; 0.0006221 0 0 0]  x5=0  V1=ones(3,3)  V2=ones(3,3)  I1=ones(3,3)  I2=ones(3,3)  nHarmo=1  Measurements=None
  _CN_158505202_110000_CN_192702885_110000 : powerlib/Elements/Distributed Parameters Line  Phases=3  Frequency=60  Resistance=[0.01273 0.3864]  Inductance="[0.9337e-3  4.1264e-3]"  Capacitance=[12.74e-9 7.751e-9]  Length=40.7307  x1=[0 0 0 0; 0.0001244 0 0 0; 0.0002488 0 0 0; 0.0003733 0 0 0; 0.0004977 0 0 0; 0.0006221 0 0 0]  x2=[0 0 0 0; 0.0001244 0 0 0; 0.0002488 0 0 0; 0.0003733 0 0 0; 0.0004977 0 0 0; 0.0006221 0 0 0]  x3=[0 0 0 0; 0.0001244 0 0 0; 0.0002488 0 0 0; 0.0003733 0 0 0; 0.0004977 0 0 0; 0.0006221 0 0 0]  x4=[0 0 0 0; 0.0001244 0 0 0; 0.0002488 0 0 0; 0.0003733 0 0 0; 0.0004977 0 0 0; 0.0006221 0 0 0]  x5=0  V1=ones(3,3)  V2=ones(3,3)  I1=ones(3,3)  I2=ones(3,3)  nHarmo=1  Measurements=None
  _CN_158505202_110000_CN_280269221_110000 : powerlib/Elements/Distributed Parameters Line  Phases=3  Frequency=60  Resistance=[0.01273 0.3864]  Inductance="[0.9337e-3  4.1264e-3]"  Capacitance=[12.74e-9 7.751e-9]  Length=44.4617  x1=[0 0 0 0; 0.0001244 0 0 0; 0.0002488 0 0 0; 0.0003733 0 0 0; 0.0004977 0 0 0; 0.0006221 0 0 0]  x2=[0 0 0 0; 0.0001244 0 0 0; 0.0002488 0 0 0; 0.0003733 0 0 0; 0.0004977 0 0 0; 0.0006221 0 0 0]  x3=[0 0 0 0; 0.0001244 0 0 0; 0.0002488 0 0 0; 0.0003733 0 0 0; 0.0004977 0 0 0; 0.0006221 0 0 0]  x4=[0 0 0 0; 0.0001244 0 0 0; 0.0002488 0 0 0; 0.0003733 0 0 0; 0.0004977 0 0 0; 0.0006221 0 0 0]  x5=0  V1=ones(3,3)  V2=ones(3,3)  I1=ones(3,3)  I2=ones(3,3)  nHarmo=1  Measurements=None
  _CN_171229484_110000_CN_210449206_110000 : powerlib/Elements/Distributed Parameters Line  Phases=3  Frequency=60  Resistance=[0.01273 0.3864]  Inductance="[0.9337e-3  4.1264e-3]"  Capacitance=[12.74e-9 7.751e-9]  Length=31.2235  x1=[0 0 0 0; 0.0001244 0 0 0; 0.0002488 0 0 0; 0.0003733 0 0 0; 0.0004977 0 0 0; 0.0006221 0 0 0]  x2=[0 0 0 0; 0.0001244 0 0 0; 0.0002488 0 0 0; 0.0003733 0 0 0; 0.0004977 0 0 0; 0.0006221 0 0 0]  x3=[0 0 0 0; 0.0001244 0 0 0; 0.0002488 0 0 0; 0.0003733 0 0 0; 0.0004977 0 0 0; 0.0006221 0 0 0]  x4=[0 0 0 0; 0.0001244 0 0 0; 0.0002488 0 0 0; 0.0003733 0 0 0; 0.0004977 0 0 0; 0.0006221 0 0 0]  x5=0  V1=ones(3,3)  V2=ones(3,3)  I1=ones(3,3)  I2=ones(3,3)  nHarmo=1  Measurements=None
  _CN_171229484_110000_CN_210457037_110000 : powerlib/Elements/Distributed Parameters Line  Phases=3  Frequency=60  Resistance=[0.01273 0.3864]  Inductance="[0.9337e-3  4.1264e-3]"  Capacitance=[12.74e-9 7.751e-9]  Length=47.9123  x1=[0 0 0 0; 0.0001244 0 0 0; 0.0002488 0 0 0; 0.0003733 0 0 0; 0.0004977 0 0 0; 0.0006221 0 0 0]  x2=[0 0 0 0; 0.0001244 0 0 0; 0.0002488 0 0 0; 0.0003733 0 0 0; 0.0004977 0 0 0; 0.0006221 0 0 0]  x3=[0 0 0 0; 0.0001244 0 0 0; 0.0002488 0 0 0; 0.0003733 0 0 0; 0.0004977 0 0 0; 0.0006221 0 0 0]  x4=[0 0 0 0; 0.0001244 0 0 0; 0.0002488 0 0 0; 0.0003733 0 0 0; 0.0004977 0 0 0; 0.0006221 0 0 0]  x5=0  V1=ones(3,3)  V2=ones(3,3)  I1=ones(3,3)  I2=ones(3,3)  nHarmo=1  Measurements=None
  _CN_171229484_110000_CN_210457043_110000 : powerlib/Elements/Distributed Parameters Line  Phases=3  Frequency=60  Resistance=[0.01273 0.3864]  Inductance="[0.9337e-3  4.1264e-3]"  Capacitance=[12.74e-9 7.751e-9]  Length=24.5655  x1=[0 0 0 0; 0.0001244 0 0 0; 0.0002488 0 0 0; 0.0003733 0 0 0; 0.0004977 0 0 0; 0.0006221 0 0 0]  x2=[0 0 0 0; 0.0001244 0 0 0; 0.0002488 0 0 0; 0.0003733 0 0 0; 0.0004977 0 0 0; 0.0006221 0 0 0]  x3=[0 0 0 0; 0.0001244 0 0 0; 0.0002488 0 0 0; 0.0003733 0 0 0; 0.0004977 0 0 0; 0.0006221 0 0 0]  x4=[0 0 0 0; 0.0001244 0 0 0; 0.0002488 0 0 0; 0.0003733 0 0 0; 0.0004977 0 0 0; 0.0006221 0 0 0]  x5=0  V1=ones(3,3)  V2=ones(3,3)  I1=ones(3,3)  I2=ones(3,3)  nHarmo=1  Measurements=None
  _CN_171229484_110000_CN_75909941_110000 : powerlib/Elements/Distributed Parameters Line  Phases=3  Frequency=60  Resistance=[0.01273 0.3864]  Inductance="[0.9337e-3  4.1264e-3]"  Capacitance=[12.74e-9 7.751e-9]  Length=21.2128  x1=[0 0 0 0; 0.0001244 0 0 0; 0.0002488 0 0 0; 0.0003733 0 0 0; 0.0004977 0 0 0; 0.0006221 0 0 0]  x2=[0 0 0 0; 0.0001244 0 0 0; 0.0002488 0 0 0; 0.0003733 0 0 0; 0.0004977 0 0 0; 0.0006221 0 0 0]  x3=[0 0 0 0; 0.0001244 0 0 0; 0.0002488 0 0 0; 0.0003733 0 0 0; 0.0004977 0 0 0; 0.0006221 0 0 0]  x4=[0 0 0 0; 0.0001244 0 0 0; 0.0002488 0 0 0; 0.0003733 0 0 0; 0.0004977 0 0 0; 0.0006221 0 0 0]  x5=0  V1=ones(3,3)  V2=ones(3,3)  I1=ones(3,3)  I2=ones(3,3)  nHarmo=1  Measurements=None
  _CN_171229484_110000_CN_95066966_110000 : powerlib/Elements/Distributed Parameters Line  Phases=3  Frequency=60  Resistance=[0.01273 0.3864]  Inductance="[0.9337e-3  4.1264e-3]"  Capacitance=[12.74e-9 7.751e-9]  Length=33.8534  x1=[0 0 0 0; 0.0001244 0 0 0; 0.0002488 0 0 0; 0.0003733 0 0 0; 0.0004977 0 0 0; 0.0006221 0 0 0]  x2=[0 0 0 0; 0.0001244 0 0 0; 0.0002488 0 0 0; 0.0003733 0 0 0; 0.0004977 0 0 0; 0.0006221 0 0 0]  x3=[0 0 0 0; 0.0001244 0 0 0; 0.0002488 0 0 0; 0.0003733 0 0 0; 0.0004977 0 0 0; 0.0006221 0 0 0]  x4=[0 0 0 0; 0.0001244 0 0 0; 0.0002488 0 0 0; 0.0003733 0 0 0; 0.0004977 0 0 0; 0.0006221 0 0 0]  x5=0  V1=ones(3,3)  V2=ones(3,3)  I1=ones(3,3)  I2=ones(3,3)  nHarmo=1  Measurements=None
  _CN_171406897_110000_CN_99049777_110000 : powerlib/Elements/Distributed Parameters Line  Phases=3  Frequency=60  Resistance=[0.01273 0.3864]  Inductance="[0.9337e-3  4.1264e-3]"  Capacitance=[12.74e-9 7.751e-9]  Length=14.7466  x1=[0 0 0 0; 0.0001244 0 0 0; 0.0002488 0 0 0; 0.0003733 0 0 0; 0.0004977 0 0 0; 0.0006221 0 0 0]  x2=[0 0 0 0; 0.0001244 0 0 0; 0.0002488 0 0 0; 0.0003733 0 0 0; 0.0004977 0 0 0; 0.0006221 0 0 0]  x3=[0 0 0 0; 0.0001244 0 0 0; 0.0002488 0 0 0; 0.0003733 0 0 0; 0.0004977 0 0 0; 0.0006221 0 0 0]  x4=[0 0 0 0; 0.0001244 0 0 0; 0.0002488 0 0 0; 0.0003733 0 0 0; 0.0004977 0 0 0; 0.0006221 0 0 0]  x5=0  V1=ones(3,3)  V2=ones(3,3)  I1=ones(3,3)  I2=ones(3,3)  nHarmo=1  Measurements=None
  _CN_171406897_110000_CN_99049787_110000 : powerlib/Elements/Distributed Parameters Line  Phases=3  Frequency=60  Resistance=[0.01273 0.3864]  Inductance="[0.9337e-3  4.1264e-3]"  Capacitance=[12.74e-9 7.751e-9]  Length=22.3731  x1=[0 0 0 0; 0.0001244 0 0 0; 0.0002488 0 0 0; 0.0003733 0 0 0; 0.0004977 0 0 0; 0.0006221 0 0 0]  x2=[0 0 0 0; 0.0001244 0 0 0; 0.0002488 0 0 0; 0.0003733 0 0 0; 0.0004977 0 0 0; 0.0006221 0 0 0]  x3=[0 0 0 0; 0.0001244 0 0 0; 0.0002488 0 0 0; 0.0003733 0 0 0; 0.0004977 0 0 0; 0.0006221 0 0 0]  x4=[0 0 0 0; 0.0001244 0 0 0; 0.0002488 0 0 0; 0.0003733 0 0 0; 0.0004977 0 0 0; 0.0006221 0 0 0]  x5=0  V1=ones(3,3)  V2=ones(3,3)  I1=ones(3,3)  I2=ones(3,3)  nHarmo=1  Measurements=None
  _CN_171406899_110000_CN_172978107_110000 : powerlib/Elements/Distributed Parameters Line  Phases=3  Frequency=60  Resistance=[0.01273 0.3864]  Inductance="[0.9337e-3  4.1264e-3]"  Capacitance=[12.74e-9 7.751e-9]  Length=36.3851  x1=[0 0 0 0; 0.0001244 0 0 0; 0.0002488 0 0 0; 0.0003733 0 0 0; 0.0004977 0 0 0; 0.0006221 0 0 0]  x2=[0 0 0 0; 0.0001244 0 0 0; 0.0002488 0 0 0; 0.0003733 0 0 0; 0.0004977 0 0 0; 0.0006221 0 0 0]  x3=[0 0 0 0; 0.0001244 0 0 0; 0.0002488 0 0 0; 0.0003733 0 0 0; 0.0004977 0 0 0; 0.0006221 0 0 0]  x4=[0 0 0 0; 0.0001244 0 0 0; 0.0002488 0 0 0; 0.0003733 0 0 0; 0.0004977 0 0 0; 0.0006221 0 0 0]  x5=0  V1=ones(3,3)  V2=ones(3,3)  I1=ones(3,3)  I2=ones(3,3)  nHarmo=1  Measurements=None
  _CN_171406899_110000_CN_175315244_110000 : powerlib/Elements/Distributed Parameters Line  Phases=3  Frequency=60  Resistance=[0.01273 0.3864]  Inductance="[0.9337e-3  4.1264e-3]"  Capacitance=[12.74e-9 7.751e-9]  Length=11.2011  x1=[0 0 0 0; 0.0001244 0 0 0; 0.0002488 0 0 0; 0.0003733 0 0 0; 0.0004977 0 0 0; 0.0006221 0 0 0]  x2=[0 0 0 0; 0.0001244 0 0 0; 0.0002488 0 0 0; 0.0003733 0 0 0; 0.0004977 0 0 0; 0.0006221 0 0 0]  x3=[0 0 0 0; 0.0001244 0 0 0; 0.0002488 0 0 0; 0.0003733 0 0 0; 0.0004977 0 0 0; 0.0006221 0 0 0]  x4=[0 0 0 0; 0.0001244 0 0 0; 0.0002488 0 0 0; 0.0003733 0 0 0; 0.0004977 0 0 0; 0.0006221 0 0 0]  x5=0  V1=ones(3,3)  V2=ones(3,3)  I1=ones(3,3)  I2=ones(3,3)  nHarmo=1  Measurements=None
  _CN_171630121_110000_CN_103554499_110000 : powerlib/Elements/Distributed Parameters Line  Phases=3  Frequency=60  Resistance=[0.01273 0.3864]  Inductance="[0.9337e-3  4.1264e-3]"  Capacitance=[12.74e-9 7.751e-9]  Length=21.1917  x1=[0 0 0 0; 0.0001244 0 0 0; 0.0002488 0 0 0; 0.0003733 0 0 0; 0.0004977 0 0 0; 0.0006221 0 0 0]  x2=[0 0 0 0; 0.0001244 0 0 0; 0.0002488 0 0 0; 0.0003733 0 0 0; 0.0004977 0 0 0; 0.0006221 0 0 0]  x3=[0 0 0 0; 0.0001244 0 0 0; 0.0002488 0 0 0; 0.0003733 0 0 0; 0.0004977 0 0 0; 0.0006221 0 0 0]  x4=[0 0 0 0; 0.0001244 0 0 0; 0.0002488 0 0 0; 0.0003733 0 0 0; 0.0004977 0 0 0; 0.0006221 0 0 0]  x5=0  V1=ones(3,3)  V2=ones(3,3)  I1=ones(3,3)  I2=ones(3,3)  nHarmo=1  Measurements=None
  _CN_171630121_110000_CN_207755729_110000 : powerlib/Elements/Distributed Parameters Line  Phases=3  Frequency=60  Resistance=[0.01273 0.3864]  Inductance="[0.9337e-3  4.1264e-3]"  Capacitance=[12.74e-9 7.751e-9]  Length=37.4246  x1=[0 0 0 0; 0.0001244 0 0 0; 0.0002488 0 0 0; 0.0003733 0 0 0; 0.0004977 0 0 0; 0.0006221 0 0 0]  x2=[0 0 0 0; 0.0001244 0 0 0; 0.0002488 0 0 0; 0.0003733 0 0 0; 0.0004977 0 0 0; 0.0006221 0 0 0]  x3=[0 0 0 0; 0.0001244 0 0 0; 0.0002488 0 0 0; 0.0003733 0 0 0; 0.0004977 0 0 0; 0.0006221 0 0 0]  x4=[0 0 0 0; 0.0001244 0 0 0; 0.0002488 0 0 0; 0.0003733 0 0 0; 0.0004977 0 0 0; 0.0006221 0 0 0]  x5=0  V1=ones(3,3)  V2=ones(3,3)  I1=ones(3,3)  I2=ones(3,3)  nHarmo=1  Measurements=None
  _CN_171630121_110000_CN_207755730_110000 : powerlib/Elements/Distributed Parameters Line  Phases=3  Frequency=60  Resistance=[0.01273 0.3864]  Inductance="[0.9337e-3  4.1264e-3]"  Capacitance=[12.74e-9 7.751e-9]  Length=36.7793  x1=[0 0 0 0; 0.0001244 0 0 0; 0.0002488 0 0 0; 0.0003733 0 0 0; 0.0004977 0 0 0; 0.0006221 0 0 0]  x2=[0 0 0 0; 0.0001244 0 0 0; 0.0002488 0 0 0; 0.0003733 0 0 0; 0.0004977 0 0 0; 0.0006221 0 0 0]  x3=[0 0 0 0; 0.0001244 0 0 0; 0.0002488 0 0 0; 0.0003733 0 0 0; 0.0004977 0 0 0; 0.0006221 0 0 0]  x4=[0 0 0 0; 0.0001244 0 0 0; 0.0002488 0 0 0; 0.0003733 0 0 0; 0.0004977 0 0 0; 0.0006221 0 0 0]  x5=0  V1=ones(3,3)  V2=ones(3,3)  I1=ones(3,3)  I2=ones(3,3)  nHarmo=1  Measurements=None
  _CN_171630144_110000_CN_103560163_110000 : powerlib/Elements/Distributed Parameters Line  Phases=3  Frequency=60  Resistance=[0.01273 0.3864]  Inductance="[0.9337e-3  4.1264e-3]"  Capacitance=[12.74e-9 7.751e-9]  Length=16.9304  x1=[0 0 0 0; 0.0001244 0 0 0; 0.0002488 0 0 0; 0.0003733 0 0 0; 0.0004977 0 0 0; 0.0006221 0 0 0]  x2=[0 0 0 0; 0.0001244 0 0 0; 0.0002488 0 0 0; 0.0003733 0 0 0; 0.0004977 0 0 0; 0.0006221 0 0 0]  x3=[0 0 0 0; 0.0001244 0 0 0; 0.0002488 0 0 0; 0.0003733 0 0 0; 0.0004977 0 0 0; 0.0006221 0 0 0]  x4=[0 0 0 0; 0.0001244 0 0 0; 0.0002488 0 0 0; 0.0003733 0 0 0; 0.0004977 0 0 0; 0.0006221 0 0 0]  x5=0  V1=ones(3,3)  V2=ones(3,3)  I1=ones(3,3)  I2=ones(3,3)  nHarmo=1  Measurements=None
  _CN_171630144_110000_CN_171630143_110000 : powerlib/Elements/Distributed Parameters Line  Phases=3  Frequency=60  Resistance=[0.01273 0.3864]  Inductance="[0.9337e-3  4.1264e-3]"  Capacitance=[12.74e-9 7.751e-9]  Length=16.6218  x1=[0 0 0 0; 0.0001244 0 0 0; 0.0002488 0 0 0; 0.0003733 0 0 0; 0.0004977 0 0 0; 0.0006221 0 0 0]  x2=[0 0 0 0; 0.0001244 0 0 0; 0.0002488 0 0 0; 0.0003733 0 0 0; 0.0004977 0 0 0; 0.0006221 0 0 0]  x3=[0 0 0 0; 0.0001244 0 0 0; 0.0002488 0 0 0; 0.0003733 0 0 0; 0.0004977 0 0 0; 0.0006221 0 0 0]  x4=[0 0 0 0; 0.0001244 0 0 0; 0.0002488 0 0 0; 0.0003733 0 0 0; 0.0004977 0 0 0; 0.0006221 0 0 0]  x5=0  V1=ones(3,3)  V2=ones(3,3)  I1=ones(3,3)  I2=ones(3,3)  nHarmo=1  Measurements=None
  _CN_171630144_110000_CN_171630149_110000 : powerlib/Elements/Distributed Parameters Line  Phases=3  Frequency=60  Resistance=[0.01273 0.3864]  Inductance="[0.9337e-3  4.1264e-3]"  Capacitance=[12.74e-9 7.751e-9]  Length=11.8118  x1=[0 0 0 0; 0.0001244 0 0 0; 0.0002488 0 0 0; 0.0003733 0 0 0; 0.0004977 0 0 0; 0.0006221 0 0 0]  x2=[0 0 0 0; 0.0001244 0 0 0; 0.0002488 0 0 0; 0.0003733 0 0 0; 0.0004977 0 0 0; 0.0006221 0 0 0]  x3=[0 0 0 0; 0.0001244 0 0 0; 0.0002488 0 0 0; 0.0003733 0 0 0; 0.0004977 0 0 0; 0.0006221 0 0 0]  x4=[0 0 0 0; 0.0001244 0 0 0; 0.0002488 0 0 0; 0.0003733 0 0 0; 0.0004977 0 0 0; 0.0006221 0 0 0]  x5=0  V1=ones(3,3)  V2=ones(3,3)  I1=ones(3,3)  I2=ones(3,3)  nHarmo=1  Measurements=None
  _CN_171630144_110000_CN_171630156_110000 : powerlib/Elements/Distributed Parameters Line  Phases=3  Frequency=60  Resistance=[0.01273 0.3864]  Inductance="[0.9337e-3  4.1264e-3]"  Capacitance=[12.74e-9 7.751e-9]  Length=2.0475  x1=[0 0 0 0; 0.0001244 0 0 0; 0.0002488 0 0 0; 0.0003733 0 0 0; 0.0004977 0 0 0; 0.0006221 0 0 0]  x2=[0 0 0 0; 0.0001244 0 0 0; 0.0002488 0 0 0; 0.0003733 0 0 0; 0.0004977 0 0 0; 0.0006221 0 0 0]  x3=[0 0 0 0; 0.0001244 0 0 0; 0.0002488 0 0 0; 0.0003733 0 0 0; 0.0004977 0 0 0; 0.0006221 0 0 0]  x4=[0 0 0 0; 0.0001244 0 0 0; 0.0002488 0 0 0; 0.0003733 0 0 0; 0.0004977 0 0 0; 0.0006221 0 0 0]  x5=0  V1=ones(3,3)  V2=ones(3,3)  I1=ones(3,3)  I2=ones(3,3)  nHarmo=1  Measurements=None
  _CN_171630144_110000_CN_171630157_110000 : powerlib/Elements/Distributed Parameters Line  Phases=3  Frequency=60  Resistance=[0.01273 0.3864]  Inductance="[0.9337e-3  4.1264e-3]"  Capacitance=[12.74e-9 7.751e-9]  Length=30.3843  x1=[0 0 0 0; 0.0001244 0 0 0; 0.0002488 0 0 0; 0.0003733 0 0 0; 0.0004977 0 0 0; 0.0006221 0 0 0]  x2=[0 0 0 0; 0.0001244 0 0 0; 0.0002488 0 0 0; 0.0003733 0 0 0; 0.0004977 0 0 0; 0.0006221 0 0 0]  x3=[0 0 0 0; 0.0001244 0 0 0; 0.0002488 0 0 0; 0.0003733 0 0 0; 0.0004977 0 0 0; 0.0006221 0 0 0]  x4=[0 0 0 0; 0.0001244 0 0 0; 0.0002488 0 0 0; 0.0003733 0 0 0; 0.0004977 0 0 0; 0.0006221 0 0 0]  x5=0  V1=ones(3,3)  V2=ones(3,3)  I1=ones(3,3)  I2=ones(3,3)  nHarmo=1  Measurements=None
  _CN_171630144_110000_CN_192646598_110000 : powerlib/Elements/Distributed Parameters Line  Phases=3  Frequency=60  Resistance=[0.01273 0.3864]  Inductance="[0.9337e-3  4.1264e-3]"  Capacitance=[12.74e-9 7.751e-9]  Length=47.8209  x1=[0 0 0 0; 0.0001244 0 0 0; 0.0002488 0 0 0; 0.0003733 0 0 0; 0.0004977 0 0 0; 0.0006221 0 0 0]  x2=[0 0 0 0; 0.0001244 0 0 0; 0.0002488 0 0 0; 0.0003733 0 0 0; 0.0004977 0 0 0; 0.0006221 0 0 0]  x3=[0 0 0 0; 0.0001244 0 0 0; 0.0002488 0 0 0; 0.0003733 0 0 0; 0.0004977 0 0 0; 0.0006221 0 0 0]  x4=[0 0 0 0; 0.0001244 0 0 0; 0.0002488 0 0 0; 0.0003733 0 0 0; 0.0004977 0 0 0; 0.0006221 0 0 0]  x5=0  V1=ones(3,3)  V2=ones(3,3)  I1=ones(3,3)  I2=ones(3,3)  nHarmo=1  Measurements=None
  _CN_171630144_110000_CN_192672898_110000 : powerlib/Elements/Distributed Parameters Line  Phases=3  Frequency=60  Resistance=[0.01273 0.3864]  Inductance="[0.9337e-3  4.1264e-3]"  Capacitance=[12.74e-9 7.751e-9]  Length=77.7515  x1=[0 0 0 0; 0.0001244 0 0 0; 0.0002488 0 0 0; 0.0003733 0 0 0; 0.0004977 0 0 0; 0.0006221 0 0 0]  x2=[0 0 0 0; 0.0001244 0 0 0; 0.0002488 0 0 0; 0.0003733 0 0 0; 0.0004977 0 0 0; 0.0006221 0 0 0]  x3=[0 0 0 0; 0.0001244 0 0 0; 0.0002488 0 0 0; 0.0003733 0 0 0; 0.0004977 0 0 0; 0.0006221 0 0 0]  x4=[0 0 0 0; 0.0001244 0 0 0; 0.0002488 0 0 0; 0.0003733 0 0 0; 0.0004977 0 0 0; 0.0006221 0 0 0]  x5=0  V1=ones(3,3)  V2=ones(3,3)  I1=ones(3,3)  I2=ones(3,3)  nHarmo=1  Measurements=None
  _CN_171630153_110000_CN_104774536_110000 : powerlib/Elements/Distributed Parameters Line  Phases=3  Frequency=60  Resistance=[0.01273 0.3864]  Inductance="[0.9337e-3  4.1264e-3]"  Capacitance=[12.74e-9 7.751e-9]  Length=10.3358  x1=[0 0 0 0; 0.0001244 0 0 0; 0.0002488 0 0 0; 0.0003733 0 0 0; 0.0004977 0 0 0; 0.0006221 0 0 0]  x2=[0 0 0 0; 0.0001244 0 0 0; 0.0002488 0 0 0; 0.0003733 0 0 0; 0.0004977 0 0 0; 0.0006221 0 0 0]  x3=[0 0 0 0; 0.0001244 0 0 0; 0.0002488 0 0 0; 0.0003733 0 0 0; 0.0004977 0 0 0; 0.0006221 0 0 0]  x4=[0 0 0 0; 0.0001244 0 0 0; 0.0002488 0 0 0; 0.0003733 0 0 0; 0.0004977 0 0 0; 0.0006221 0 0 0]  x5=0  V1=ones(3,3)  V2=ones(3,3)  I1=ones(3,3)  I2=ones(3,3)  nHarmo=1  Measurements=None
  _CN_171630153_110000_CN_239589747_110000 : powerlib/Elements/Distributed Parameters Line  Phases=3  Frequency=60  Resistance=[0.01273 0.3864]  Inductance="[0.9337e-3  4.1264e-3]"  Capacitance=[12.74e-9 7.751e-9]  Length=12.8314  x1=[0 0 0 0; 0.0001244 0 0 0; 0.0002488 0 0 0; 0.0003733 0 0 0; 0.0004977 0 0 0; 0.0006221 0 0 0]  x2=[0 0 0 0; 0.0001244 0 0 0; 0.0002488 0 0 0; 0.0003733 0 0 0; 0.0004977 0 0 0; 0.0006221 0 0 0]  x3=[0 0 0 0; 0.0001244 0 0 0; 0.0002488 0 0 0; 0.0003733 0 0 0; 0.0004977 0 0 0; 0.0006221 0 0 0]  x4=[0 0 0 0; 0.0001244 0 0 0; 0.0002488 0 0 0; 0.0003733 0 0 0; 0.0004977 0 0 0; 0.0006221 0 0 0]  x5=0  V1=ones(3,3)  V2=ones(3,3)  I1=ones(3,3)  I2=ones(3,3)  nHarmo=1  Measurements=None
  _CN_171868832_110000_CN_218223015_110000 : powerlib/Elements/Distributed Parameters Line  Phases=3  Frequency=60  Resistance=[0.01273 0.3864]  Inductance="[0.9337e-3  4.1264e-3]"  Capacitance=[12.74e-9 7.751e-9]  Length=22.2049  x1=[0 0 0 0; 0.0001244 0 0 0; 0.0002488 0 0 0; 0.0003733 0 0 0; 0.0004977 0 0 0; 0.0006221 0 0 0]  x2=[0 0 0 0; 0.0001244 0 0 0; 0.0002488 0 0 0; 0.0003733 0 0 0; 0.0004977 0 0 0; 0.0006221 0 0 0]  x3=[0 0 0 0; 0.0001244 0 0 0; 0.0002488 0 0 0; 0.0003733 0 0 0; 0.0004977 0 0 0; 0.0006221 0 0 0]  x4=[0 0 0 0; 0.0001244 0 0 0; 0.0002488 0 0 0; 0.0003733 0 0 0; 0.0004977 0 0 0; 0.0006221 0 0 0]  x5=0  V1=ones(3,3)  V2=ones(3,3)  I1=ones(3,3)  I2=ones(3,3)  nHarmo=1  Measurements=None
  _CN_171868832_110000_CN_220065702_110000 : powerlib/Elements/Distributed Parameters Line  Phases=3  Frequency=60  Resistance=[0.01273 0.3864]  Inductance="[0.9337e-3  4.1264e-3]"  Capacitance=[12.74e-9 7.751e-9]  Length=30.6164  x1=[0 0 0 0; 0.0001244 0 0 0; 0.0002488 0 0 0; 0.0003733 0 0 0; 0.0004977 0 0 0; 0.0006221 0 0 0]  x2=[0 0 0 0; 0.0001244 0 0 0; 0.0002488 0 0 0; 0.0003733 0 0 0; 0.0004977 0 0 0; 0.0006221 0 0 0]  x3=[0 0 0 0; 0.0001244 0 0 0; 0.0002488 0 0 0; 0.0003733 0 0 0; 0.0004977 0 0 0; 0.0006221 0 0 0]  x4=[0 0 0 0; 0.0001244 0 0 0; 0.0002488 0 0 0; 0.0003733 0 0 0; 0.0004977 0 0 0; 0.0006221 0 0 0]  x5=0  V1=ones(3,3)  V2=ones(3,3)  I1=ones(3,3)  I2=ones(3,3)  nHarmo=1  Measurements=None
  _CN_171868832_110000_CN_257169562_110000 : powerlib/Elements/Distributed Parameters Line  Phases=3  Frequency=60  Resistance=[0.01273 0.3864]  Inductance="[0.9337e-3  4.1264e-3]"  Capacitance=[12.74e-9 7.751e-9]  Length=6.9424  x1=[0 0 0 0; 0.0001244 0 0 0; 0.0002488 0 0 0; 0.0003733 0 0 0; 0.0004977 0 0 0; 0.0006221 0 0 0]  x2=[0 0 0 0; 0.0001244 0 0 0; 0.0002488 0 0 0; 0.0003733 0 0 0; 0.0004977 0 0 0; 0.0006221 0 0 0]  x3=[0 0 0 0; 0.0001244 0 0 0; 0.0002488 0 0 0; 0.0003733 0 0 0; 0.0004977 0 0 0; 0.0006221 0 0 0]  x4=[0 0 0 0; 0.0001244 0 0 0; 0.0002488 0 0 0; 0.0003733 0 0 0; 0.0004977 0 0 0; 0.0006221 0 0 0]  x5=0  V1=ones(3,3)  V2=ones(3,3)  I1=ones(3,3)  I2=ones(3,3)  nHarmo=1  Measurements=None
  _CN_171987005_110000_CN_173944057_110000 : powerlib/Elements/Distributed Parameters Line  Phases=3  Frequency=60  Resistance=[0.01273 0.3864]  Inductance="[0.9337e-3  4.1264e-3]"  Capacitance=[12.74e-9 7.751e-9]  Length=6.4954  x1=[0 0 0 0; 0.0001244 0 0 0; 0.0002488 0 0 0; 0.0003733 0 0 0; 0.0004977 0 0 0; 0.0006221 0 0 0]  x2=[0 0 0 0; 0.0001244 0 0 0; 0.0002488 0 0 0; 0.0003733 0 0 0; 0.0004977 0 0 0; 0.0006221 0 0 0]  x3=[0 0 0 0; 0.0001244 0 0 0; 0.0002488 0 0 0; 0.0003733 0 0 0; 0.0004977 0 0 0; 0.0006221 0 0 0]  x4=[0 0 0 0; 0.0001244 0 0 0; 0.0002488 0 0 0; 0.0003733 0 0 0; 0.0004977 0 0 0; 0.0006221 0 0 0]  x5=0  V1=ones(3,3)  V2=ones(3,3)  I1=ones(3,3)  I2=ones(3,3)  nHarmo=1  Measurements=None
  _CN_171987005_110000_CN_173944061_110000 : powerlib/Elements/Distributed Parameters Line  Phases=3  Frequency=60  Resistance=[0.01273 0.3864]  Inductance="[0.9337e-3  4.1264e-3]"  Capacitance=[12.74e-9 7.751e-9]  Length=23.5236  x1=[0 0 0 0; 0.0001244 0 0 0; 0.0002488 0 0 0; 0.0003733 0 0 0; 0.0004977 0 0 0; 0.0006221 0 0 0]  x2=[0 0 0 0; 0.0001244 0 0 0; 0.0002488 0 0 0; 0.0003733 0 0 0; 0.0004977 0 0 0; 0.0006221 0 0 0]  x3=[0 0 0 0; 0.0001244 0 0 0; 0.0002488 0 0 0; 0.0003733 0 0 0; 0.0004977 0 0 0; 0.0006221 0 0 0]  x4=[0 0 0 0; 0.0001244 0 0 0; 0.0002488 0 0 0; 0.0003733 0 0 0; 0.0004977 0 0 0; 0.0006221 0 0 0]  x5=0  V1=ones(3,3)  V2=ones(3,3)  I1=ones(3,3)  I2=ones(3,3)  nHarmo=1  Measurements=None
  _CN_172018985_110000_CN_172019090_110000 : powerlib/Elements/Distributed Parameters Line  Phases=3  Frequency=60  Resistance=[0.01273 0.3864]  Inductance="[0.9337e-3  4.1264e-3]"  Capacitance=[12.74e-9 7.751e-9]  Length=16.9563  x1=[0 0 0 0; 0.0001244 0 0 0; 0.0002488 0 0 0; 0.0003733 0 0 0; 0.0004977 0 0 0; 0.0006221 0 0 0]  x2=[0 0 0 0; 0.0001244 0 0 0; 0.0002488 0 0 0; 0.0003733 0 0 0; 0.0004977 0 0 0; 0.0006221 0 0 0]  x3=[0 0 0 0; 0.0001244 0 0 0; 0.0002488 0 0 0; 0.0003733 0 0 0; 0.0004977 0 0 0; 0.0006221 0 0 0]  x4=[0 0 0 0; 0.0001244 0 0 0; 0.0002488 0 0 0; 0.0003733 0 0 0; 0.0004977 0 0 0; 0.0006221 0 0 0]  x5=0  V1=ones(3,3)  V2=ones(3,3)  I1=ones(3,3)  I2=ones(3,3)  nHarmo=1  Measurements=None
  _CN_172178550_110000_CN_172178562_110000 : powerlib/Elements/Distributed Parameters Line  Phases=3  Frequency=60  Resistance=[0.01273 0.3864]  Inductance="[0.9337e-3  4.1264e-3]"  Capacitance=[12.74e-9 7.751e-9]  Length=23.0232  x1=[0 0 0 0; 0.0001244 0 0 0; 0.0002488 0 0 0; 0.0003733 0 0 0; 0.0004977 0 0 0; 0.0006221 0 0 0]  x2=[0 0 0 0; 0.0001244 0 0 0; 0.0002488 0 0 0; 0.0003733 0 0 0; 0.0004977 0 0 0; 0.0006221 0 0 0]  x3=[0 0 0 0; 0.0001244 0 0 0; 0.0002488 0 0 0; 0.0003733 0 0 0; 0.0004977 0 0 0; 0.0006221 0 0 0]  x4=[0 0 0 0; 0.0001244 0 0 0; 0.0002488 0 0 0; 0.0003733 0 0 0; 0.0004977 0 0 0; 0.0006221 0 0 0]  x5=0  V1=ones(3,3)  V2=ones(3,3)  I1=ones(3,3)  I2=ones(3,3)  nHarmo=1  Measurements=None
  _CN_172178550_110000_CN_172590051_110000 : powerlib/Elements/Distributed Parameters Line  Phases=3  Frequency=60  Resistance=[0.01273 0.3864]  Inductance="[0.9337e-3  4.1264e-3]"  Capacitance=[12.74e-9 7.751e-9]  Length=10.2605  x1=[0 0 0 0; 0.0001244 0 0 0; 0.0002488 0 0 0; 0.0003733 0 0 0; 0.0004977 0 0 0; 0.0006221 0 0 0]  x2=[0 0 0 0; 0.0001244 0 0 0; 0.0002488 0 0 0; 0.0003733 0 0 0; 0.0004977 0 0 0; 0.0006221 0 0 0]  x3=[0 0 0 0; 0.0001244 0 0 0; 0.0002488 0 0 0; 0.0003733 0 0 0; 0.0004977 0 0 0; 0.0006221 0 0 0]  x4=[0 0 0 0; 0.0001244 0 0 0; 0.0002488 0 0 0; 0.0003733 0 0 0; 0.0004977 0 0 0; 0.0006221 0 0 0]  x5=0  V1=ones(3,3)  V2=ones(3,3)  I1=ones(3,3)  I2=ones(3,3)  nHarmo=1  Measurements=None
  _CN_172178551_110000_CN_172178560_110000 : powerlib/Elements/Distributed Parameters Line  Phases=3  Frequency=60  Resistance=[0.01273 0.3864]  Inductance="[0.9337e-3  4.1264e-3]"  Capacitance=[12.74e-9 7.751e-9]  Length=14.6225  x1=[0 0 0 0; 0.0001244 0 0 0; 0.0002488 0 0 0; 0.0003733 0 0 0; 0.0004977 0 0 0; 0.0006221 0 0 0]  x2=[0 0 0 0; 0.0001244 0 0 0; 0.0002488 0 0 0; 0.0003733 0 0 0; 0.0004977 0 0 0; 0.0006221 0 0 0]  x3=[0 0 0 0; 0.0001244 0 0 0; 0.0002488 0 0 0; 0.0003733 0 0 0; 0.0004977 0 0 0; 0.0006221 0 0 0]  x4=[0 0 0 0; 0.0001244 0 0 0; 0.0002488 0 0 0; 0.0003733 0 0 0; 0.0004977 0 0 0; 0.0006221 0 0 0]  x5=0  V1=ones(3,3)  V2=ones(3,3)  I1=ones(3,3)  I2=ones(3,3)  nHarmo=1  Measurements=None
  _CN_172178551_110000_CN_172178562_110000 : powerlib/Elements/Distributed Parameters Line  Phases=3  Frequency=60  Resistance=[0.01273 0.3864]  Inductance="[0.9337e-3  4.1264e-3]"  Capacitance=[12.74e-9 7.751e-9]  Length=16.4011  x1=[0 0 0 0; 0.0001244 0 0 0; 0.0002488 0 0 0; 0.0003733 0 0 0; 0.0004977 0 0 0; 0.0006221 0 0 0]  x2=[0 0 0 0; 0.0001244 0 0 0; 0.0002488 0 0 0; 0.0003733 0 0 0; 0.0004977 0 0 0; 0.0006221 0 0 0]  x3=[0 0 0 0; 0.0001244 0 0 0; 0.0002488 0 0 0; 0.0003733 0 0 0; 0.0004977 0 0 0; 0.0006221 0 0 0]  x4=[0 0 0 0; 0.0001244 0 0 0; 0.0002488 0 0 0; 0.0003733 0 0 0; 0.0004977 0 0 0; 0.0006221 0 0 0]  x5=0  V1=ones(3,3)  V2=ones(3,3)  I1=ones(3,3)  I2=ones(3,3)  nHarmo=1  Measurements=None
  _CN_172178551_110000_CN_172178563_110000 : powerlib/Elements/Distributed Parameters Line  Phases=3  Frequency=60  Resistance=[0.01273 0.3864]  Inductance="[0.9337e-3  4.1264e-3]"  Capacitance=[12.74e-9 7.751e-9]  Length=23.264  x1=[0 0 0 0; 0.0001244 0 0 0; 0.0002488 0 0 0; 0.0003733 0 0 0; 0.0004977 0 0 0; 0.0006221 0 0 0]  x2=[0 0 0 0; 0.0001244 0 0 0; 0.0002488 0 0 0; 0.0003733 0 0 0; 0.0004977 0 0 0; 0.0006221 0 0 0]  x3=[0 0 0 0; 0.0001244 0 0 0; 0.0002488 0 0 0; 0.0003733 0 0 0; 0.0004977 0 0 0; 0.0006221 0 0 0]  x4=[0 0 0 0; 0.0001244 0 0 0; 0.0002488 0 0 0; 0.0003733 0 0 0; 0.0004977 0 0 0; 0.0006221 0 0 0]  x5=0  V1=ones(3,3)  V2=ones(3,3)  I1=ones(3,3)  I2=ones(3,3)  nHarmo=1  Measurements=None
  _CN_172178556_110000_CN_166814917_110000 : powerlib/Elements/Distributed Parameters Line  Phases=3  Frequency=60  Resistance=[0.01273 0.3864]  Inductance="[0.9337e-3  4.1264e-3]"  Capacitance=[12.74e-9 7.751e-9]  Length=0.13567  x1=[0 0 0 0; 0.0001244 0 0 0; 0.0002488 0 0 0; 0.0003733 0 0 0; 0.0004977 0 0 0; 0.0006221 0 0 0]  x2=[0 0 0 0; 0.0001244 0 0 0; 0.0002488 0 0 0; 0.0003733 0 0 0; 0.0004977 0 0 0; 0.0006221 0 0 0]  x3=[0 0 0 0; 0.0001244 0 0 0; 0.0002488 0 0 0; 0.0003733 0 0 0; 0.0004977 0 0 0; 0.0006221 0 0 0]  x4=[0 0 0 0; 0.0001244 0 0 0; 0.0002488 0 0 0; 0.0003733 0 0 0; 0.0004977 0 0 0; 0.0006221 0 0 0]  x5=0  V1=ones(3,3)  V2=ones(3,3)  I1=ones(3,3)  I2=ones(3,3)  nHarmo=1  Measurements=None
  _CN_172178563_110000_CN_172394893_110000 : powerlib/Elements/Distributed Parameters Line  Phases=3  Frequency=60  Resistance=[0.01273 0.3864]  Inductance="[0.9337e-3  4.1264e-3]"  Capacitance=[12.74e-9 7.751e-9]  Length=64.2529  x1=[0 0 0 0; 0.0001244 0 0 0; 0.0002488 0 0 0; 0.0003733 0 0 0; 0.0004977 0 0 0; 0.0006221 0 0 0]  x2=[0 0 0 0; 0.0001244 0 0 0; 0.0002488 0 0 0; 0.0003733 0 0 0; 0.0004977 0 0 0; 0.0006221 0 0 0]  x3=[0 0 0 0; 0.0001244 0 0 0; 0.0002488 0 0 0; 0.0003733 0 0 0; 0.0004977 0 0 0; 0.0006221 0 0 0]  x4=[0 0 0 0; 0.0001244 0 0 0; 0.0002488 0 0 0; 0.0003733 0 0 0; 0.0004977 0 0 0; 0.0006221 0 0 0]  x5=0  V1=ones(3,3)  V2=ones(3,3)  I1=ones(3,3)  I2=ones(3,3)  nHarmo=1  Measurements=None
  _CN_172178563_110000_CN_172394924_110000 : powerlib/Elements/Distributed Parameters Line  Phases=3  Frequency=60  Resistance=[0.01273 0.3864]  Inductance="[0.9337e-3  4.1264e-3]"  Capacitance=[12.74e-9 7.751e-9]  Length=48.637  x1=[0 0 0 0; 0.0001244 0 0 0; 0.0002488 0 0 0; 0.0003733 0 0 0; 0.0004977 0 0 0; 0.0006221 0 0 0]  x2=[0 0 0 0; 0.0001244 0 0 0; 0.0002488 0 0 0; 0.0003733 0 0 0; 0.0004977 0 0 0; 0.0006221 0 0 0]  x3=[0 0 0 0; 0.0001244 0 0 0; 0.0002488 0 0 0; 0.0003733 0 0 0; 0.0004977 0 0 0; 0.0006221 0 0 0]  x4=[0 0 0 0; 0.0001244 0 0 0; 0.0002488 0 0 0; 0.0003733 0 0 0; 0.0004977 0 0 0; 0.0006221 0 0 0]  x5=0  V1=ones(3,3)  V2=ones(3,3)  I1=ones(3,3)  I2=ones(3,3)  nHarmo=1  Measurements=None
